simulink model "ImpedanceControl"  (R2017a)
(part 7 of 14)

(((real(dq6.*cos(q6).*(sin(q2-q3).*sin(q5).*8.191520442889917e-1-cos(q2-q3).*cos(q4).*cos(q5)+cos(q2-q3).*sin(q4).*sin(q5).*5.735764363510462e-1))+real(sin(q6).*(dq5.*sin(q2-q3).*cos(q5).*8.191520442889917e-1+cos(q2-q3).*sin(q5).*(dq2-dq3).*8.191520442889917e-1+dq4.*cos(q2-q3).*cos(q4).*sin(q5).*5.735764363510462e-1+dq4.*cos(q2-q3).*cos(q5).*sin(q4)+dq5.*cos(q2-q3).*cos(q4).*sin(q5)+dq5.*cos(q2-q3).*cos(q5).*sin(q4).*5.735764363510462e-1+sin(q2-q3).*cos(q4).*cos(q5).*(dq2-dq3)-sin(q2-q3).*sin(q4).*sin(q5).*(dq2-dq3).*5.735764363510462e-1))-imag(sin(q2-q3).*sin(q4).*(dq2-dq3)).*4.698463103929542e-1-imag(dq5.*sin(q5).*(sin(q2-q3).*8.191520442889917e-1+cos(q2-q3).*sin(q4).*5.735764363510462e-1)).*8.191520442889917e-1-imag(cos(q2-q3).*(dq2-dq3)).*3.289899283371657e-1-real(cos(q6).*(cos(q5).*(cos(q2-q3).*(dq2-dq3).*8.191520442889917e-1+dq4.*cos(q2-q3).*cos(q4).*5.735764363510462e-1-sin(q2-q3).*sin(q4).*(dq2-dq3).*5.735764363510462e-1).*5.735764363510462e-1+cos(q2-q3).*(dq2-dq3).*4.698463103929542e-1-dq4.*cos(q2-q3).*cos(q4).*6.710100716628342e-1+sin(q2-q3).*sin(q4).*(dq2-dq3).*6.710100716628342e-1-dq5.*sin(q5).*(sin(q2-q3).*8.191520442889917e-1+cos(q2-q3).*sin(q4).*5.735764363510462e-1).*5.735764363510462e-1+dq5.*cos(q2-q3).*cos(q4).*cos(q5).*5.735764363510462e-1-dq4.*cos(q2-q3).*sin(q4).*sin(q5).*5.735764363510462e-1-sin(q2-q3).*cos(q4).*sin(q5).*(dq2-dq3).*5.735764363510462e-1))+imag(cos(q5).*(cos(q2-q3).*(dq2-dq3).*8.191520442889917e-1+dq4.*cos(q2-q3).*cos(q4).*5.735764363510462e-1-sin(q2-q3).*sin(q4).*(dq2-dq3).*5.735764363510462e-1)).*8.191520442889917e-1+real(dq6.*sin(q6).*(sin(q2-q3).*4.698463103929542e-1-cos(q2-q3).*sin(q4).*6.710100716628342e-1+cos(q5).*(sin(q2-q3).*8.191520442889917e-1+cos(q2-q3).*sin(q4).*5.735764363510462e-1).*5.735764363510462e-1+cos(q2-q3).*cos(q4).*sin(q5).*5.735764363510462e-1))+imag(dq5.*cos(q2-q3).*cos(q4).*cos(q5)).*8.191520442889917e-1-imag(dq4.*cos(q2-q3).*sin(q4).*sin(q5)).*8.191520442889917e-1+imag(dq4.*cos(q2-q3).*cos(q4)).*4.698463103929542e-1-imag(sin(q2-q3).*cos(q4).*sin(q5).*(dq2-dq3)).*8.191520442889917e-1)./(real(cos(q2-q3)).*3.289899283371657e-1+real(sin(q2-q3).*cos(q4).*sin(q5)).*8.191520442889917e-1+real(sin(q2-q3).*sin(q4)).*4.698463103929542e-1+imag(sin(q6).*(cos(q2-q3).*sin(q5).*8.191520442889917e-1+sin(q2-q3).*cos(q4).*cos(q5)-sin(q2-q3).*sin(q4).*sin(q5).*5.735764363510462e-1))-real(cos(q5).*(cos(q2-q3).*8.191520442889917e-1-sin(q2-q3).*sin(q4).*5.735764363510462e-1)).*8.191520442889917e-1-imag(cos(q6).*(cos(q2-q3).*4.698463103929542e-1+sin(q2-q3).*sin(q4).*6.710100716628342e-1+cos(q5).*(cos(q2-q3).*8.191520442889917e-1-sin(q2-q3).*sin(q4).*5.735764363510462e-1).*5.735764363510462e-1-sin(q2-q3).*cos(q4).*sin(q5).*5.735764363510462e-1)))-(real(sin(q2-q3)).*(-3.289899283371657e-1)+real(cos(q2-q3).*cos(q4).*sin(q5)).*8.191520442889917e-1+real(cos(q2-q3).*sin(q4)).*4.698463103929542e-1-imag(sin(q6).*(sin(q2-q3).*sin(q5).*8.191520442889917e-1-cos(q2-q3).*cos(q4).*cos(q5)+cos(q2-q3).*sin(q4).*sin(q5).*5.735764363510462e-1))+real(cos(q5).*(sin(q2-q3).*8.191520442889917e-1+cos(q2-q3).*sin(q4).*5.735764363510462e-1)).*8.191520442889917e-1+imag(cos(q6).*(sin(q2-q3).*4.698463103929542e-1-cos(q2-q3).*sin(q4).*6.710100716628342e-1+cos(q5).*(sin(q2-q3).*8.191520442889917e-1+cos(q2-q3).*sin(q4).*5.735764363510462e-1).*5.735764363510462e-1+cos(q2-q3).*cos(q4).*sin(q5).*5.735764363510462e-1))).*1.0./(real(cos(q2-q3)).*3.289899283371657e-1+real(sin(q2-q3).*cos(q4).*sin(q5)).*8.191520442889917e-1+real(sin(q2-q3).*sin(q4)).*4.698463103929542e-1+imag(sin(q6).*(cos(q2-q3).*sin(q5).*8.191520442889917e-1+sin(q2-q3).*cos(q4).*cos(q5)-sin(q2-q3).*sin(q4).*sin(q5).*5.735764363510462e-1))-real(cos(q5).*(cos(q2-q3).*8.191520442889917e-1-sin(q2-q3).*sin(q4).*5.735764363510462e-1)).*8.191520442889917e-1-imag(cos(q6).*(cos(q2-q3).*4.698463103929542e-1+sin(q2-q3).*sin(q4).*6.710100716628342e-1+cos(q5).*(cos(q2-q3).*8.191520442889917e-1-sin(q2-q3).*sin(q4).*5.735764363510462e-1).*5.735764363510462e-1-sin(q2-q3).*cos(q4).*sin(q5).*5.735764363510462e-1))).^2.*(-real(dq6.*cos(q6).*(cos(q2-q3).*sin(q5).*8.191520442889917e-1+sin(q2-q3).*cos(q4).*cos(q5)-sin(q2-q3).*sin(q4).*sin(q5).*5.735764363510462e-1))+imag(cos(q2-q3).*sin(q4).*(dq2-dq3)).*4.698463103929542e-1+imag(dq5.*sin(q5).*(cos(q2-q3).*8.191520442889917e-1-sin(q2-q3).*sin(q4).*5.735764363510462e-1)).*8.191520442889917e-1+real(sin(q6).*(dq5.*cos(q2-q3).*cos(q5).*(-8.191520442889917e-1)+sin(q2-q3).*sin(q5).*(dq2-dq3).*8.191520442889917e-1+dq4.*sin(q2-q3).*cos(q4).*sin(q5).*5.735764363510462e-1+dq4.*sin(q2-q3).*cos(q5).*sin(q4)+dq5.*sin(q2-q3).*cos(q4).*sin(q5)+dq5.*sin(q2-q3).*cos(q5).*sin(q4).*5.735764363510462e-1-cos(q2-q3).*cos(q4).*cos(q5).*(dq2-dq3)+cos(q2-q3).*sin(q4).*sin(q5).*(dq2-dq3).*5.735764363510462e-1))-imag(sin(q2-q3).*(dq2-dq3)).*3.289899283371657e-1-real(cos(q6).*(cos(q5).*(sin(q2-q3).*(dq2-dq3).*8.191520442889917e-1+dq4.*sin(q2-q3).*cos(q4).*5.735764363510462e-1+cos(q2-q3).*sin(q4).*(dq2-dq3).*5.735764363510462e-1).*5.735764363510462e-1+sin(q2-q3).*(dq2-dq3).*4.698463103929542e-1-dq4.*sin(q2-q3).*cos(q4).*6.710100716628342e-1-cos(q2-q3).*sin(q4).*(dq2-dq3).*6.710100716628342e-1+dq5.*sin(q5).*(cos(q2-q3).*8.191520442889917e-1-sin(q2-q3).*sin(q4).*5.735764363510462e-1).*5.735764363510462e-1+dq5.*sin(q2-q3).*cos(q4).*cos(q5).*5.735764363510462e-1-dq4.*sin(q2-q3).*sin(q4).*sin(q5).*5.735764363510462e-1+cos(q2-q3).*cos(q4).*sin(q5).*(dq2-dq3).*5.735764363510462e-1))+imag(cos(q5).*(sin(q2-q3).*(dq2-dq3).*8.191520442889917e-1+dq4.*sin(q2-q3).*cos(q4).*5.735764363510462e-1+cos(q2-q3).*sin(q4).*(dq2-dq3).*5.735764363510462e-1)).*8.191520442889917e-1-real(dq6.*sin(q6).*(cos(q2-q3).*4.698463103929542e-1+sin(q2-q3).*sin(q4).*6.710100716628342e-1+cos(q5).*(cos(q2-q3).*8.191520442889917e-1-sin(q2-q3).*sin(q4).*5.735764363510462e-1).*5.735764363510462e-1-sin(q2-q3).*cos(q4).*sin(q5).*5.735764363510462e-1))+imag(dq5.*sin(q2-q3).*cos(q4).*cos(q5)).*8.191520442889917e-1-imag(dq4.*sin(q2-q3).*sin(q4).*sin(q5)).*8.191520442889917e-1+imag(cos(q2-q3).*cos(q4).*sin(q5).*(dq2-dq3)).*8.191520442889917e-1+imag(dq4.*sin(q2-q3).*cos(q4)).*4.698463103929542e-1)-(imag(sin(q2-q3)).*(-3.289899283371657e-1)+imag(cos(q2-q3).*cos(q4).*sin(q5)).*8.191520442889917e-1+imag(cos(q2-q3).*sin(q4)).*4.698463103929542e-1+real(sin(q6).*(sin(q2-q3).*sin(q5).*8.191520442889917e-1-cos(q2-q3).*cos(q4).*cos(q5)+cos(q2-q3).*sin(q4).*sin(q5).*5.735764363510462e-1))+imag(cos(q5).*(sin(q2-q3).*8.191520442889917e-1+cos(q2-q3).*sin(q4).*5.735764363510462e-1)).*8.191520442889917e-1-real(cos(q6).*(sin(q2-q3).*4.698463103929542e-1-cos(q2-q3).*sin(q4).*6.710100716628342e-1+cos(q5).*(sin(q2-q3).*8.191520442889917e-1+cos(q2-q3).*sin(q4).*5.735764363510462e-1).*5.735764363510462e-1+cos(q2-q3).*cos(q4).*sin(q5).*5.735764363510462e-1))).*1.0./(real(cos(q2-q3)).*3.289899283371657e-1+real(sin(q2-q3).*cos(q4).*sin(q5)).*8.191520442889917e-1+real(sin(q2-q3).*sin(q4)).*4.698463103929542e-1+imag(sin(q6).*(cos(q2-q3).*sin(q5).*8.191520442889917e-1+sin(q2-q3).*cos(q4).*cos(q5)-sin(q2-q3).*sin(q4).*sin(q5).*5.735764363510462e-1))-real(cos(q5).*(cos(q2-q3).*8.191520442889917e-1-sin(q2-q3).*sin(q4).*5.735764363510462e-1)).*8.191520442889917e-1-imag(cos(q6).*(cos(q2-q3).*4.698463103929542e-1+sin(q2-q3).*sin(q4).*6.710100716628342e-1+cos(q5).*(cos(q2-q3).*8.191520442889917e-1-sin(q2-q3).*sin(q4).*5.735764363510462e-1).*5.735764363510462e-1-sin(q2-q3).*cos(q4).*sin(q5).*5.735764363510462e-1))).^2.*(imag(dq6.*cos(q6).*(cos(q2-q3).*sin(q5).*8.191520442889917e-1+sin(q2-q3).*cos(q4).*cos(q5)-sin(q2-q3).*sin(q4).*sin(q5).*5.735764363510462e-1))+real(cos(q2-q3).*sin(q4).*(dq2-dq3)).*4.698463103929542e-1-imag(sin(q6).*(dq5.*cos(q2-q3).*cos(q5).*(-8.191520442889917e-1)+sin(q2-q3).*sin(q5).*(dq2-dq3).*8.191520442889917e-1+dq4.*sin(q2-q3).*cos(q4).*sin(q5).*5.735764363510462e-1+dq4.*sin(q2-q3).*cos(q5).*sin(q4)+dq5.*sin(q2-q3).*cos(q4).*sin(q5)+dq5.*sin(q2-q3).*cos(q5).*sin(q4).*5.735764363510462e-1-cos(q2-q3).*cos(q4).*cos(q5).*(dq2-dq3)+cos(q2-q3).*sin(q4).*sin(q5).*(dq2-dq3).*5.735764363510462e-1))+real(dq5.*sin(q5).*(cos(q2-q3).*8.191520442889917e-1-sin(q2-q3).*sin(q4).*5.735764363510462e-1)).*8.191520442889917e-1-real(sin(q2-q3).*(dq2-dq3)).*3.289899283371657e-1+imag(cos(q6).*(cos(q5).*(sin(q2-q3).*(dq2-dq3).*8.191520442889917e-1+dq4.*sin(q2-q3).*cos(q4).*5.735764363510462e-1+cos(q2-q3).*sin(q4).*(dq2-dq3).*5.735764363510462e-1).*5.735764363510462e-1+sin(q2-q3).*(dq2-dq3).*4.698463103929542e-1-dq4.*sin(q2-q3).*cos(q4).*6.710100716628342e-1-cos(q2-q3).*sin(q4).*(dq2-dq3).*6.710100716628342e-1+dq5.*sin(q5).*(cos(q2-q3).*8.191520442889917e-1-sin(q2-q3).*sin(q4).*5.735764363510462e-1).*5.735764363510462e-1+dq5.*sin(q2-q3).*cos(q4).*cos(q5).*5.735764363510462e-1-dq4.*sin(q2-q3).*sin(q4).*sin(q5).*5.735764363510462e-1+cos(q2-q3).*cos(q4).*sin(q5).*(dq2-dq3).*5.735764363510462e-1))+imag(dq6.*sin(q6).*(cos(q2-q3).*4.698463103929542e-1+sin(q2-q3).*sin(q4).*6.710100716628342e-1+cos(q5).*(cos(q2-q3).*8.191520442889917e-1-sin(q2-q3).*sin(q4).*5.735764363510462e-1).*5.735764363510462e-1-sin(q2-q3).*cos(q4).*sin(q5).*5.735764363510462e-1))+real(cos(q5).*(sin(q2-q3).*(dq2-dq3).*8.191520442889917e-1+dq4.*sin(q2-q3).*cos(q4).*5.735764363510462e-1+cos(q2-q3).*sin(q4).*(dq2-dq3).*5.735764363510462e-1)).*8.191520442889917e-1+real(dq5.*sin(q2-q3).*cos(q4).*cos(q5)).*8.191520442889917e-1-real(dq4.*sin(q2-q3).*sin(q4).*sin(q5)).*8.191520442889917e-1+real(cos(q2-q3).*cos(q4).*sin(q5).*(dq2-dq3)).*8.191520442889917e-1+real(dq4.*sin(q2-q3).*cos(q4)).*4.698463103929542e-1)+(real(cos(q6).*(cos(q2-q3).*4.698463103929542e-1+sin(q2-q3).*sin(q4).*6.710100716628342e-1+cos(q5).*(cos(q2-q3).*8.191520442889917e-1-sin(q2-q3).*sin(q4).*5.735764363510462e-1).*5.735764363510462e-1-sin(q2-q3).*cos(q4).*sin(q5).*5.735764363510462e-1))+imag(cos(q2-q3)).*3.289899283371657e-1+imag(sin(q2-q3).*cos(q4).*sin(q5)).*8.191520442889917e-1+imag(sin(q2-q3).*sin(q4)).*4.698463103929542e-1-real(sin(q6).*(cos(q2-q3).*sin(q5).*8.191520442889917e-1+sin(q2-q3).*cos(q4).*cos(q5)-sin(q2-q3).*sin(q4).*sin(q5).*5.735764363510462e-1))-imag(cos(q5).*(cos(q2-q3).*8.191520442889917e-1-sin(q2-q3).*sin(q4).*5.735764363510462e-1)).*8.191520442889917e-1).*1.0./(real(cos(q2-q3)).*3.289899283371657e-1+real(sin(q2-q3).*cos(q4).*sin(q5)).*8.191520442889917e-1+real(sin(q2-q3).*sin(q4)).*4.698463103929542e-1+imag(sin(q6).*(cos(q2-q3).*sin(q5).*8.191520442889917e-1+sin(q2-q3).*cos(q4).*cos(q5)-sin(q2-q3).*sin(q4).*sin(q5).*5.735764363510462e-1))-real(cos(q5).*(cos(q2-q3).*8.191520442889917e-1-sin(q2-q3).*sin(q4).*5.735764363510462e-1)).*8.191520442889917e-1-imag(cos(q6).*(cos(q2-q3).*4.698463103929542e-1+sin(q2-q3).*sin(q4).*6.710100716628342e-1+cos(q5).*(cos(q2-q3).*8.191520442889917e-1-sin(q2-q3).*sin(q4).*5.735764363510462e-1).*5.735764363510462e-1-sin(q2-q3).*cos(q4).*sin(q5).*5.735764363510462e-1))).^2.*(real(sin(q2-q3).*cos(q4).*sin(q5).*(dq2-dq3)).*8.191520442889917e-1+imag(sin(q6).*(dq5.*sin(q2-q3).*cos(q5).*8.191520442889917e-1+cos(q2-q3).*sin(q5).*(dq2-dq3).*8.191520442889917e-1+dq4.*cos(q2-q3).*cos(q4).*sin(q5).*5.735764363510462e-1+dq4.*cos(q2-q3).*cos(q5).*sin(q4)+dq5.*cos(q2-q3).*cos(q4).*sin(q5)+dq5.*cos(q2-q3).*cos(q5).*sin(q4).*5.735764363510462e-1+sin(q2-q3).*cos(q4).*cos(q5).*(dq2-dq3)-sin(q2-q3).*sin(q4).*sin(q5).*(dq2-dq3).*5.735764363510462e-1))+real(sin(q2-q3).*sin(q4).*(dq2-dq3)).*4.698463103929542e-1-imag(cos(q6).*(cos(q5).*(cos(q2-q3).*(dq2-dq3).*8.191520442889917e-1+dq4.*cos(q2-q3).*cos(q4).*5.735764363510462e-1-sin(q2-q3).*sin(q4).*(dq2-dq3).*5.735764363510462e-1).*5.735764363510462e-1+cos(q2-q3).*(dq2-dq3).*4.698463103929542e-1-dq4.*cos(q2-q3).*cos(q4).*6.710100716628342e-1+sin(q2-q3).*sin(q4).*(dq2-dq3).*6.710100716628342e-1-dq5.*sin(q5).*(sin(q2-q3).*8.191520442889917e-1+cos(q2-q3).*sin(q4).*5.735764363510462e-1).*5.735764363510462e-1+dq5.*cos(q2-q3).*cos(q4).*cos(q5).*5.735764363510462e-1-dq4.*cos(q2-q3).*sin(q4).*sin(q5).*5.735764363510462e-1-sin(q2-q3).*cos(q4).*sin(q5).*(dq2-dq3).*5.735764363510462e-1))+real(dq5.*sin(q5).*(sin(q2-q3).*8.191520442889917e-1+cos(q2-q3).*sin(q4).*5.735764363510462e-1)).*8.191520442889917e-1+real(cos(q2-q3).*(dq2-dq3)).*3.289899283371657e-1+imag(dq6.*sin(q6).*(sin(q2-q3).*4.698463103929542e-1-cos(q2-q3).*sin(q4).*6.710100716628342e-1+cos(q5).*(sin(q2-q3).*8.191520442889917e-1+cos(q2-q3).*sin(q4).*5.735764363510462e-1).*5.735764363510462e-1+cos(q2-q3).*cos(q4).*sin(q5).*5.735764363510462e-1))-real(cos(q5).*(cos(q2-q3).*(dq2-dq3).*8.191520442889917e-1+dq4.*cos(q2-q3).*cos(q4).*5.735764363510462e-1-sin(q2-q3).*sin(q4).*(dq2-dq3).*5.735764363510462e-1)).*8.191520442889917e-1-real(dq5.*cos(q2-q3).*cos(q4).*cos(q5)).*8.191520442889917e-1+real(dq4.*cos(q2-q3).*sin(q4).*sin(q5)).*8.191520442889917e-1-real(dq4.*cos(q2-q3).*cos(q4)).*4.698463103929542e-1+imag(dq6.*cos(q6).*(sin(q2-q3).*sin(q5).*8.191520442889917e-1-cos(q2-q3).*cos(q4).*cos(q5)+cos(q2-q3).*sin(q4).*sin(q5).*5.735764363510462e-1)))+(real(sin(q2-q3)).*(-3.289899283371657e-1)+real(cos(q2-q3).*cos(q4).*sin(q5)).*8.191520442889917e-1+real(cos(q2-q3).*sin(q4)).*4.698463103929542e-1-imag(sin(q6).*(sin(q2-q3).*sin(q5).*8.191520442889917e-1-cos(q2-q3).*cos(q4).*cos(q5)+cos(q2-q3).*sin(q4).*sin(q5).*5.735764363510462e-1))+real(cos(q5).*(sin(q2-q3).*8.191520442889917e-1+cos(q2-q3).*sin(q4).*5.735764363510462e-1)).*8.191520442889917e-1+imag(cos(q6).*(sin(q2-q3).*4.698463103929542e-1-cos(q2-q3).*sin(q4).*6.710100716628342e-1+cos(q5).*(sin(q2-q3).*8.191520442889917e-1+cos(q2-q3).*sin(q4).*5.735764363510462e-1).*5.735764363510462e-1+cos(q2-q3).*cos(q4).*sin(q5).*5.735764363510462e-1))).*(real(cos(q6).*(cos(q2-q3).*4.698463103929542e-1+sin(q2-q3).*sin(q4).*6.710100716628342e-1+cos(q5).*(cos(q2-q3).*8.191520442889917e-1-sin(q2-q3).*sin(q4).*5.735764363510462e-1).*5.735764363510462e-1-sin(q2-q3).*cos(q4).*sin(q5).*5.735764363510462e-1))+imag(cos(q2-q3)).*3.289899283371657e-1+imag(sin(q2-q3).*cos(q4).*sin(q5)).*8.191520442889917e-1+imag(sin(q2-q3).*sin(q4)).*4.698463103929542e-1-real(sin(q6).*(cos(q2-q3).*sin(q5).*8.191520442889917e-1+sin(q2-q3).*cos(q4).*cos(q5)-sin(q2-q3).*sin(q4).*sin(q5).*5.735764363510462e-1))-imag(cos(q5).*(cos(q2-q3).*8.191520442889917e-1-sin(q2-q3).*sin(q4).*5.735764363510462e-1)).*8.191520442889917e-1).*1.0./(real(cos(q2-q3)).*3.289899283371657e-1+real(sin(q2-q3).*cos(q4).*sin(q5)).*8.191520442889917e-1+real(sin(q2-q3).*sin(q4)).*4.698463103929542e-1+imag(sin(q6).*(cos(q2-q3).*sin(q5).*8.191520442889917e-1+sin(q2-q3).*cos(q4).*cos(q5)-sin(q2-q3).*sin(q4).*sin(q5).*5.735764363510462e-1))-real(cos(q5).*(cos(q2-q3).*8.191520442889917e-1-sin(q2-q3).*sin(q4).*5.735764363510462e-1)).*8.191520442889917e-1-imag(cos(q6).*(cos(q2-q3).*4.698463103929542e-1+sin(q2-q3).*sin(q4).*6.710100716628342e-1+cos(q5).*(cos(q2-q3).*8.191520442889917e-1-sin(q2-q3).*sin(q4).*5.735764363510462e-1).*5.735764363510462e-1-sin(q2-q3).*cos(q4).*sin(q5).*5.735764363510462e-1))).^3.*(imag(dq6.*cos(q6).*(cos(q2-q3).*sin(q5).*8.191520442889917e-1+sin(q2-q3).*cos(q4).*cos(q5)-sin(q2-q3).*sin(q4).*sin(q5).*5.735764363510462e-1))+real(cos(q2-q3).*sin(q4).*(dq2-dq3)).*4.698463103929542e-1-imag(sin(q6).*(dq5.*cos(q2-q3).*cos(q5).*(-8.191520442889917e-1)+sin(q2-q3).*sin(q5).*(dq2-dq3).*8.191520442889917e-1+dq4.*sin(q2-q3).*cos(q4).*sin(q5).*5.735764363510462e-1+dq4.*sin(q2-q3).*cos(q5).*sin(q4)+dq5.*sin(q2-q3).*cos(q4).*sin(q5)+dq5.*sin(q2-q3).*cos(q5).*sin(q4).*5.735764363510462e-1-cos(q2-q3).*cos(q4).*cos(q5).*(dq2-dq3)+cos(q2-q3).*sin(q4).*sin(q5).*(dq2-dq3).*5.735764363510462e-1))+real(dq5.*sin(q5).*(cos(q2-q3).*8.191520442889917e-1-sin(q2-q3).*sin(q4).*5.735764363510462e-1)).*8.191520442889917e-1-real(sin(q2-q3).*(dq2-dq3)).*3.289899283371657e-1+imag(cos(q6).*(cos(q5).*(sin(q2-q3).*(dq2-dq3).*8.191520442889917e-1+dq4.*sin(q2-q3).*cos(q4).*5.735764363510462e-1+cos(q2-q3).*sin(q4).*(dq2-dq3).*5.735764363510462e-1).*5.735764363510462e-1+sin(q2-q3).*(dq2-dq3).*4.698463103929542e-1-dq4.*sin(q2-q3).*cos(q4).*6.710100716628342e-1-cos(q2-q3).*sin(q4).*(dq2-dq3).*6.710100716628342e-1+dq5.*sin(q5).*(cos(q2-q3).*8.191520442889917e-1-sin(q2-q3).*sin(q4).*5.735764363510462e-1).*5.735764363510462e-1+dq5.*sin(q2-q3).*cos(q4).*cos(q5).*5.735764363510462e-1-dq4.*sin(q2-q3).*sin(q4).*sin(q5).*5.735764363510462e-1+cos(q2-q3).*cos(q4).*sin(q5).*(dq2-dq3).*5.735764363510462e-1))+imag(dq6.*sin(q6).*(cos(q2-q3).*4.698463103929542e-1+sin(q2-q3).*sin(q4).*6.710100716628342e-1+cos(q5).*(cos(q2-q3).*8.191520442889917e-1-sin(q2-q3).*sin(q4).*5.735764363510462e-1).*5.735764363510462e-1-sin(q2-q3).*cos(q4).*sin(q5).*5.735764363510462e-1))+real(cos(q5).*(sin(q2-q3).*(dq2-dq3).*8.191520442889917e-1+dq4.*sin(q2-q3).*cos(q4).*5.735764363510462e-1+cos(q2-q3).*sin(q4).*(dq2-dq3).*5.735764363510462e-1)).*8.191520442889917e-1+real(dq5.*sin(q2-q3).*cos(q4).*cos(q5)).*8.191520442889917e-1-real(dq4.*sin(q2-q3).*sin(q4).*sin(q5)).*8.191520442889917e-1+real(cos(q2-q3).*cos(q4).*sin(q5).*(dq2-dq3)).*8.191520442889917e-1+real(dq4.*sin(q2-q3).*cos(q4)).*4.698463103929542e-1).*2.0).*(real(cos(q2-q3)).*3.289899283371657e-1+real(sin(q2-q3).*cos(q4).*sin(q5)).*8.191520442889917e-1+real(sin(q2-q3).*sin(q4)).*4.698463103929542e-1+imag(sin(q6).*(cos(q2-q3).*sin(q5).*8.191520442889917e-1+sin(q2-q3).*cos(q4).*cos(q5)-sin(q2-q3).*sin(q4).*sin(q5).*5.735764363510462e-1))-real(cos(q5).*(cos(q2-q3).*8.191520442889917e-1-sin(q2-q3).*sin(q4).*5.735764363510462e-1)).*8.191520442889917e-1-imag(cos(q6).*(cos(q2-q3).*4.698463103929542e-1+sin(q2-q3).*sin(q4).*6.710100716628342e-1+cos(q5).*(cos(q2-q3).*8.191520442889917e-1-sin(q2-q3).*sin(q4).*5.735764363510462e-1).*5.735764363510462e-1-sin(q2-q3).*cos(q4).*sin(q5).*5.735764363510462e-1))).^2)./((real(cos(q6).*(cos(q2-q3).*4.698463103929542e-1+sin(q2-q3).*sin(q4).*6.710100716628342e-1+cos(q5).*(cos(q2-q3).*8.191520442889917e-1-sin(q2-q3).*sin(q4).*5.735764363510462e-1).*5.735764363510462e-1-sin(q2-q3).*cos(q4).*sin(q5).*5.735764363510462e-1))+imag(cos(q2-q3)).*3.289899283371657e-1+imag(sin(q2-q3).*cos(q4).*sin(q5)).*8.191520442889917e-1+imag(sin(q2-q3).*sin(q4)).*4.698463103929542e-1-real(sin(q6).*(cos(q2-q3).*sin(q5).*8.191520442889917e-1+sin(q2-q3).*cos(q4).*cos(q5)-sin(q2-q3).*sin(q4).*sin(q5).*5.735764363510462e-1))-imag(cos(q5).*(cos(q2-q3).*8.191520442889917e-1-sin(q2-q3).*sin(q4).*5.735764363510462e-1)).*8.191520442889917e-1).^2+(real(cos(q2-q3)).*3.289899283371657e-1+real(sin(q2-q3).*cos(q4).*sin(q5)).*8.191520442889917e-1+real(sin(q2-q3).*sin(q4)).*4.698463103929542e-1+imag(sin(q6).*(cos(q2-q3).*sin(q5).*8.191520442889917e-1+sin(q2-q3).*cos(q4).*cos(q5)-sin(q2-q3).*sin(q4).*sin(q5).*5.735764363510462e-1))-real(cos(q5).*(cos(q2-q3).*8.191520442889917e-1-sin(q2-q3).*sin(q4).*5.735764363510462e-1)).*8.191520442889917e-1-imag(cos(q6).*(cos(q2-q3).*4.698463103929542e-1+sin(q2-q3).*sin(q4).*6.710100716628342e-1+cos(q5).*(cos(q2-q3).*8.191520442889917e-1-sin(q2-q3).*sin(q4).*5.735764363510462e-1).*5.735764363510462e-1-sin(q2-q3).*cos(q4).*sin(q5).*5.735764363510462e-1))).^2)-((imag(sin(q2-q3)).*(-3.289899283371657e-1)+imag(cos(q2-q3).*cos(q4).*sin(q5)).*8.191520442889917e-1+imag(cos(q2-q3).*sin(q4)).*4.698463103929542e-1+real(sin(q6).*(sin(q2-q3).*sin(q5).*8.191520442889917e-1-cos(q2-q3).*cos(q4).*cos(q5)+cos(q2-q3).*sin(q4).*sin(q5).*5.735764363510462e-1))+imag(cos(q5).*(sin(q2-q3).*8.191520442889917e-1+cos(q2-q3).*sin(q4).*5.735764363510462e-1)).*8.191520442889917e-1-real(cos(q6).*(sin(q2-q3).*4.698463103929542e-1-cos(q2-q3).*sin(q4).*6.710100716628342e-1+cos(q5).*(sin(q2-q3).*8.191520442889917e-1+cos(q2-q3).*sin(q4).*5.735764363510462e-1).*5.735764363510462e-1+cos(q2-q3).*cos(q4).*sin(q5).*5.735764363510462e-1)))./(real(cos(q2-q3)).*3.289899283371657e-1+real(sin(q2-q3).*cos(q4).*sin(q5)).*8.191520442889917e-1+real(sin(q2-q3).*sin(q4)).*4.698463103929542e-1+imag(sin(q6).*(cos(q2-q3).*sin(q5).*8.191520442889917e-1+sin(q2-q3).*cos(q4).*cos(q5)-sin(q2-q3).*sin(q4).*sin(q5).*5.735764363510462e-1))-real(cos(q5).*(cos(q2-q3).*8.191520442889917e-1-sin(q2-q3).*sin(q4).*5.735764363510462e-1)).*8.191520442889917e-1-imag(cos(q6).*(cos(q2-q3).*4.698463103929542e-1+sin(q2-q3).*sin(q4).*6.710100716628342e-1+cos(q5).*(cos(q2-q3).*8.191520442889917e-1-sin(q2-q3).*sin(q4).*5.735764363510462e-1).*5.735764363510462e-1-sin(q2-q3).*cos(q4).*sin(q5).*5.735764363510462e-1)))-(real(sin(q2-q3)).*(-3.289899283371657e-1)+real(cos(q2-q3).*cos(q4).*sin(q5)).*8.191520442889917e-1+real(cos(q2-q3).*sin(q4)).*4.698463103929542e-1-imag(sin(q6).*(sin(q2-q3).*sin(q5).*8.191520442889917e-1-cos(q2-q3).*cos(q4).*cos(q5)+cos(q2-q3).*sin(q4).*sin(q5).*5.735764363510462e-1))+real(cos(q5).*(sin(q2-q3).*8.191520442889917e-1+cos(q2-q3).*sin(q4).*5.735764363510462e-1)).*8.191520442889917e-1+imag(cos(q6).*(sin(q2-q3).*4.698463103929542e-1-cos(q2-q3).*sin(q4).*6.710100716628342e-1+cos(q5).*(sin(q2-q3).*8.191520442889917e-1+cos(q2-q3).*sin(q4).*5.735764363510462e-1).*5.735764363510462e-1+cos(q2-q3).*cos(q4).*sin(q5).*5.735764363510462e-1))).*(real(cos(q6).*(cos(q2-q3).*4.698463103929542e-1+sin(q2-q3).*sin(q4).*6.710100716628342e-1+cos(q5).*(cos(q2-q3).*8.191520442889917e-1-sin(q2-q3).*sin(q4).*5.735764363510462e-1).*5.735764363510462e-1-sin(q2-q3).*cos(q4).*sin(q5).*5.735764363510462e-1))+imag(cos(q2-q3)).*3.289899283371657e-1+imag(sin(q2-q3).*cos(q4).*sin(q5)).*8.191520442889917e-1+imag(sin(q2-q3).*sin(q4)).*4.698463103929542e-1-real(sin(q6).*(cos(q2-q3).*sin(q5).*8.191520442889917e-1+sin(q2-q3).*cos(q4).*cos(q5)-sin(q2-q3).*sin(q4).*sin(q5).*5.735764363510462e-1))-imag(cos(q5).*(cos(q2-q3).*8.191520442889917e-1-sin(q2-q3).*sin(q4).*5.735764363510462e-1)).*8.191520442889917e-1).*1.0./(real(cos(q2-q3)).*3.289899283371657e-1+real(sin(q2-q3).*cos(q4).*sin(q5)).*8.191520442889917e-1+real(sin(q2-q3).*sin(q4)).*4.698463103929542e-1+imag(sin(q6).*(cos(q2-q3).*sin(q5).*8.191520442889917e-1+sin(q2-q3).*cos(q4).*cos(q5)-sin(q2-q3).*sin(q4).*sin(q5).*5.735764363510462e-1))-real(cos(q5).*(cos(q2-q3).*8.191520442889917e-1-sin(q2-q3).*sin(q4).*5.735764363510462e-1)).*8.191520442889917e-1-imag(cos(q6).*(cos(q2-q3).*4.698463103929542e-1+sin(q2-q3).*sin(q4).*6.710100716628342e-1+cos(q5).*(cos(q2-q3).*8.191520442889917e-1-sin(q2-q3).*sin(q4).*5.735764363510462e-1).*5.735764363510462e-1-sin(q2-q3).*cos(q4).*sin(q5).*5.735764363510462e-1))).^2).*1.0./((real(cos(q6).*(cos(q2-q3).*4.698463103929542e-1+sin(q2-q3).*sin(q4).*6.710100716628342e-1+cos(q5).*(cos(q2-q3).*8.191520442889917e-1-sin(q2-q3).*sin(q4).*5.735764363510462e-1).*5.735764363510462e-1-sin(q2-q3).*cos(q4).*sin(q5).*5.735764363510462e-1))+imag(cos(q2-q3)).*3.289899283371657e-1+imag(sin(q2-q3).*cos(q4).*sin(q5)).*8.191520442889917e-1+imag(sin(q2-q3).*sin(q4)).*4.698463103929542e-1-real(sin(q6).*(cos(q2-q3).*sin(q5).*8.191520442889917e-1+sin(q2-q3).*cos(q4).*cos(q5)-sin(q2-q3).*sin(q4).*sin(q5).*5.735764363510462e-1))-imag(cos(q5).*(cos(q2-q3).*8.191520442889917e-1-sin(q2-q3).*sin(q4).*5.735764363510462e-1)).*8.191520442889917e-1).^2+(real(cos(q2-q3)).*3.289899283371657e-1+real(sin(q2-q3).*cos(q4).*sin(q5)).*8.191520442889917e-1+real(sin(q2-q3).*sin(q4)).*4.698463103929542e-1+imag(sin(q6).*(cos(q2-q3).*sin(q5).*8.191520442889917e-1+sin(q2-q3).*cos(q4).*cos(q5)-sin(q2-q3).*sin(q4).*sin(q5).*5.735764363510462e-1))-real(cos(q5).*(cos(q2-q3).*8.191520442889917e-1-sin(q2-q3).*sin(q4).*5.735764363510462e-1)).*8.191520442889917e-1-imag(cos(q6).*(cos(q2-q3).*4.698463103929542e-1+sin(q2-q3).*sin(q4).*6.710100716628342e-1+cos(q5).*(cos(q2-q3).*8.191520442889917e-1-sin(q2-q3).*sin(q4).*5.735764363510462e-1).*5.735764363510462e-1-sin(q2-q3).*cos(q4).*sin(q5).*5.735764363510462e-1))).^2).^2.*((real(cos(q6).*(cos(q2-q3).*4.698463103929542e-1+sin(q2-q3).*sin(q4).*6.710100716628342e-1+cos(q5).*(cos(q2-q3).*8.191520442889917e-1-sin(q2-q3).*sin(q4).*5.735764363510462e-1).*5.735764363510462e-1-sin(q2-q3).*cos(q4).*sin(q5).*5.735764363510462e-1))+imag(cos(q2-q3)).*3.289899283371657e-1+imag(sin(q2-q3).*cos(q4).*sin(q5)).*8.191520442889917e-1+imag(sin(q2-q3).*sin(q4)).*4.698463103929542e-1-real(sin(q6).*(cos(q2-q3).*sin(q5).*8.191520442889917e-1+sin(q2-q3).*cos(q4).*cos(q5)-sin(q2-q3).*sin(q4).*sin(q5).*5.735764363510462e-1))-imag(cos(q5).*(cos(q2-q3).*8.191520442889917e-1-sin(q2-q3).*sin(q4).*5.735764363510462e-1)).*8.191520442889917e-1).*(-real(dq6.*cos(q6).*(cos(q2-q3).*sin(q5).*8.191520442889917e-1+sin(q2-q3).*cos(q4).*cos(q5)-sin(q2-q3).*sin(q4).*sin(q5).*5.735764363510462e-1))+imag(cos(q2-q3).*sin(q4).*(dq2-dq3)).*4.698463103929542e-1+imag(dq5.*sin(q5).*(cos(q2-q3).*8.191520442889917e-1-sin(q2-q3).*sin(q4).*5.735764363510462e-1)).*8.191520442889917e-1+real(sin(q6).*(dq5.*cos(q2-q3).*cos(q5).*(-8.191520442889917e-1)+sin(q2-q3).*sin(q5).*(dq2-dq3).*8.191520442889917e-1+dq4.*sin(q2-q3).*cos(q4).*sin(q5).*5.735764363510462e-1+dq4.*sin(q2-q3).*cos(q5).*sin(q4)+dq5.*sin(q2-q3).*cos(q4).*sin(q5)+dq5.*sin(q2-q3).*cos(q5).*sin(q4).*5.735764363510462e-1-cos(q2-q3).*cos(q4).*cos(q5).*(dq2-dq3)+cos(q2-q3).*sin(q4).*sin(q5).*(dq2-dq3).*5.735764363510462e-1))-imag(sin(q2-q3).*(dq2-dq3)).*3.289899283371657e-1-real(cos(q6).*(cos(q5).*(sin(q2-q3).*(dq2-dq3).*8.191520442889917e-1+dq4.*sin(q2-q3).*cos(q4).*5.735764363510462e-1+cos(q2-q3).*sin(q4).*(dq2-dq3).*5.735764363510462e-1).*5.735764363510462e-1+sin(q2-q3).*(dq2-dq3).*4.698463103929542e-1-dq4.*sin(q2-q3).*cos(q4).*6.710100716628342e-1-cos(q2-q3).*sin(q4).*(dq2-dq3).*6.710100716628342e-1+dq5.*sin(q5).*(cos(q2-q3).*8.191520442889917e-1-sin(q2-q3).*sin(q4).*5.735764363510462e-1).*5.735764363510462e-1+dq5.*sin(q2-q3).*cos(q4).*cos(q5).*5.735764363510462e-1-dq4.*sin(q2-q3).*sin(q4).*sin(q5).*5.735764363510462e-1+cos(q2-q3).*cos(q4).*sin(q5).*(dq2-dq3).*5.735764363510462e-1))+imag(cos(q5).*(sin(q2-q3).*(dq2-dq3).*8.191520442889917e-1+dq4.*sin(q2-q3).*cos(q4).*5.735764363510462e-1+cos(q2-q3).*sin(q4).*(dq2-dq3).*5.735764363510462e-1)).*8.191520442889917e-1-real(dq6.*sin(q6).*(cos(q2-q3).*4.698463103929542e-1+sin(q2-q3).*sin(q4).*6.710100716628342e-1+cos(q5).*(cos(q2-q3).*8.191520442889917e-1-sin(q2-q3).*sin(q4).*5.735764363510462e-1).*5.735764363510462e-1-sin(q2-q3).*cos(q4).*sin(q5).*5.735764363510462e-1))+imag(dq5.*sin(q2-q3).*cos(q4).*cos(q5)).*8.191520442889917e-1-imag(dq4.*sin(q2-q3).*sin(q4).*sin(q5)).*8.191520442889917e-1+imag(cos(q2-q3).*cos(q4).*sin(q5).*(dq2-dq3)).*8.191520442889917e-1+imag(dq4.*sin(q2-q3).*cos(q4)).*4.698463103929542e-1).*2.0+(real(cos(q2-q3)).*3.289899283371657e-1+real(sin(q2-q3).*cos(q4).*sin(q5)).*8.191520442889917e-1+real(sin(q2-q3).*sin(q4)).*4.698463103929542e-1+imag(sin(q6).*(cos(q2-q3).*sin(q5).*8.191520442889917e-1+sin(q2-q3).*cos(q4).*cos(q5)-sin(q2-q3).*sin(q4).*sin(q5).*5.735764363510462e-1))-real(cos(q5).*(cos(q2-q3).*8.191520442889917e-1-sin(q2-q3).*sin(q4).*5.735764363510462e-1)).*8.191520442889917e-1-imag(cos(q6).*(cos(q2-q3).*4.698463103929542e-1+sin(q2-q3).*sin(q4).*6.710100716628342e-1+cos(q5).*(cos(q2-q3).*8.191520442889917e-1-sin(q2-q3).*sin(q4).*5.735764363510462e-1).*5.735764363510462e-1-sin(q2-q3).*cos(q4).*sin(q5).*5.735764363510462e-1))).*(imag(dq6.*cos(q6).*(cos(q2-q3).*sin(q5).*8.191520442889917e-1+sin(q2-q3).*cos(q4).*cos(q5)-sin(q2-q3).*sin(q4).*sin(q5).*5.735764363510462e-1))+real(cos(q2-q3).*sin(q4).*(dq2-dq3)).*4.698463103929542e-1-imag(sin(q6).*(dq5.*cos(q2-q3).*cos(q5).*(-8.191520442889917e-1)+sin(q2-q3).*sin(q5).*(dq2-dq3).*8.191520442889917e-1+dq4.*sin(q2-q3).*cos(q4).*sin(q5).*5.735764363510462e-1+dq4.*sin(q2-q3).*cos(q5).*sin(q4)+dq5.*sin(q2-q3).*cos(q4).*sin(q5)+dq5.*sin(q2-q3).*cos(q5).*sin(q4).*5.735764363510462e-1-cos(q2-q3).*cos(q4).*cos(q5).*(dq2-dq3)+cos(q2-q3).*sin(q4).*sin(q5).*(dq2-dq3).*5.735764363510462e-1))+real(dq5.*sin(q5).*(cos(q2-q3).*8.191520442889917e-1-sin(q2-q3).*sin(q4).*5.735764363510462e-1)).*8.191520442889917e-1-real(sin(q2-q3).*(dq2-dq3)).*3.289899283371657e-1+imag(cos(q6).*(cos(q5).*(sin(q2-q3).*(dq2-dq3).*8.191520442889917e-1+dq4.*sin(q2-q3).*cos(q4).*5.735764363510462e-1+cos(q2-q3).*sin(q4).*(dq2-dq3).*5.735764363510462e-1).*5.735764363510462e-1+sin(q2-q3).*(dq2-dq3).*4.698463103929542e-1-dq4.*sin(q2-q3).*cos(q4).*6.710100716628342e-1-cos(q2-q3).*sin(q4).*(dq2-dq3).*6.710100716628342e-1+dq5.*sin(q5).*(cos(q2-q3).*8.191520442889917e-1-sin(q2-q3).*sin(q4).*5.735764363510462e-1).*5.735764363510462e-1+dq5.*sin(q2-q3).*cos(q4).*cos(q5).*5.735764363510462e-1-dq4.*sin(q2-q3).*sin(q4).*sin(q5).*5.735764363510462e-1+cos(q2-q3).*cos(q4).*sin(q5).*(dq2-dq3).*5.735764363510462e-1))+imag(dq6.*sin(q6).*(cos(q2-q3).*4.698463103929542e-1+sin(q2-q3).*sin(q4).*6.710100716628342e-1+cos(q5).*(cos(q2-q3).*8.191520442889917e-1-sin(q2-q3).*sin(q4).*5.735764363510462e-1).*5.735764363510462e-1-sin(q2-q3).*cos(q4).*sin(q5).*5.735764363510462e-1))+real(cos(q5).*(sin(q2-q3).*(dq2-dq3).*8.191520442889917e-1+dq4.*sin(q2-q3).*cos(q4).*5.735764363510462e-1+cos(q2-q3).*sin(q4).*(dq2-dq3).*5.735764363510462e-1)).*8.191520442889917e-1+real(dq5.*sin(q2-q3).*cos(q4).*cos(q5)).*8.191520442889917e-1-real(dq4.*sin(q2-q3).*sin(q4).*sin(q5)).*8.191520442889917e-1+real(cos(q2-q3).*cos(q4).*sin(q5).*(dq2-dq3)).*8.191520442889917e-1+real(dq4.*sin(q2-q3).*cos(q4)).*4.698463103929542e-1).*2.0).*(real(cos(q2-q3)).*3.289899283371657e-1+real(sin(q2-q3).*cos(q4).*sin(q5)).*8.191520442889917e-1+real(sin(q2-q3).*sin(q4)).*4.698463103929542e-1+imag(sin(q6).*(cos(q2-q3).*sin(q5).*8.191520442889917e-1+sin(q2-q3).*cos(q4).*cos(q5)-sin(q2-q3).*sin(q4).*sin(q5).*5.735764363510462e-1))-real(cos(q5).*(cos(q2-q3).*8.191520442889917e-1-sin(q2-q3).*sin(q4).*5.735764363510462e-1)).*8.191520442889917e-1-imag(cos(q6).*(cos(q2-q3).*4.698463103929542e-1+sin(q2-q3).*sin(q4).*6.710100716628342e-1+cos(q5).*(cos(q2-q3).*8.191520442889917e-1-sin(q2-q3).*sin(q4).*5.735764363510462e-1).*5.735764363510462e-1-sin(q2-q3).*cos(q4).*sin(q5).*5.735764363510462e-1))).^2+(((imag(sin(q2-q3)).*(-3.289899283371657e-1)+imag(cos(q2-q3).*cos(q4).*sin(q5)).*8.191520442889917e-1+imag(cos(q2-q3).*sin(q4)).*4.698463103929542e-1+real(sin(q6).*(sin(q2-q3).*sin(q5).*8.191520442889917e-1-cos(q2-q3).*cos(q4).*cos(q5)+cos(q2-q3).*sin(q4).*sin(q5).*5.735764363510462e-1))+imag(cos(q5).*(sin(q2-q3).*8.191520442889917e-1+cos(q2-q3).*sin(q4).*5.735764363510462e-1)).*8.191520442889917e-1-real(cos(q6).*(sin(q2-q3).*4.698463103929542e-1-cos(q2-q3).*sin(q4).*6.710100716628342e-1+cos(q5).*(sin(q2-q3).*8.191520442889917e-1+cos(q2-q3).*sin(q4).*5.735764363510462e-1).*5.735764363510462e-1+cos(q2-q3).*cos(q4).*sin(q5).*5.735764363510462e-1)))./(real(cos(q2-q3)).*3.289899283371657e-1+real(sin(q2-q3).*cos(q4).*sin(q5)).*8.191520442889917e-1+real(sin(q2-q3).*sin(q4)).*4.698463103929542e-1+imag(sin(q6).*(cos(q2-q3).*sin(q5).*8.191520442889917e-1+sin(q2-q3).*cos(q4).*cos(q5)-sin(q2-q3).*sin(q4).*sin(q5).*5.735764363510462e-1))-real(cos(q5).*(cos(q2-q3).*8.191520442889917e-1-sin(q2-q3).*sin(q4).*5.735764363510462e-1)).*8.191520442889917e-1-imag(cos(q6).*(cos(q2-q3).*4.698463103929542e-1+sin(q2-q3).*sin(q4).*6.710100716628342e-1+cos(q5).*(cos(q2-q3).*8.191520442889917e-1-sin(q2-q3).*sin(q4).*5.735764363510462e-1).*5.735764363510462e-1-sin(q2-q3).*cos(q4).*sin(q5).*5.735764363510462e-1)))-(real(sin(q2-q3)).*(-3.289899283371657e-1)+real(cos(q2-q3).*cos(q4).*sin(q5)).*8.191520442889917e-1+real(cos(q2-q3).*sin(q4)).*4.698463103929542e-1-imag(sin(q6).*(sin(q2-q3).*sin(q5).*8.191520442889917e-1-cos(q2-q3).*cos(q4).*cos(q5)+cos(q2-q3).*sin(q4).*sin(q5).*5.735764363510462e-1))+real(cos(q5).*(sin(q2-q3).*8.191520442889917e-1+cos(q2-q3).*sin(q4).*5.735764363510462e-1)).*8.191520442889917e-1+imag(cos(q6).*(sin(q2-q3).*4.698463103929542e-1-cos(q2-q3).*sin(q4).*6.710100716628342e-1+cos(q5).*(sin(q2-q3).*8.191520442889917e-1+cos(q2-q3).*sin(q4).*5.735764363510462e-1).*5.735764363510462e-1+cos(q2-q3).*cos(q4).*sin(q5).*5.735764363510462e-1))).*(real(cos(q6).*(cos(q2-q3).*4.698463103929542e-1+sin(q2-q3).*sin(q4).*6.710100716628342e-1+cos(q5).*(cos(q2-q3).*8.191520442889917e-1-sin(q2-q3).*sin(q4).*5.735764363510462e-1).*5.735764363510462e-1-sin(q2-q3).*cos(q4).*sin(q5).*5.735764363510462e-1))+imag(cos(q2-q3)).*3.289899283371657e-1+imag(sin(q2-q3).*cos(q4).*sin(q5)).*8.191520442889917e-1+imag(sin(q2-q3).*sin(q4)).*4.698463103929542e-1-real(sin(q6).*(cos(q2-q3).*sin(q5).*8.191520442889917e-1+sin(q2-q3).*cos(q4).*cos(q5)-sin(q2-q3).*sin(q4).*sin(q5).*5.735764363510462e-1))-imag(cos(q5).*(cos(q2-q3).*8.191520442889917e-1-sin(q2-q3).*sin(q4).*5.735764363510462e-1)).*8.191520442889917e-1).*1.0./(real(cos(q2-q3)).*3.289899283371657e-1+real(sin(q2-q3).*cos(q4).*sin(q5)).*8.191520442889917e-1+real(sin(q2-q3).*sin(q4)).*4.698463103929542e-1+imag(sin(q6).*(cos(q2-q3).*sin(q5).*8.191520442889917e-1+sin(q2-q3).*cos(q4).*cos(q5)-sin(q2-q3).*sin(q4).*sin(q5).*5.735764363510462e-1))-real(cos(q5).*(cos(q2-q3).*8.191520442889917e-1-sin(q2-q3).*sin(q4).*5.735764363510462e-1)).*8.191520442889917e-1-imag(cos(q6).*(cos(q2-q3).*4.698463103929542e-1+sin(q2-q3).*sin(q4).*6.710100716628342e-1+cos(q5).*(cos(q2-q3).*8.191520442889917e-1-sin(q2-q3).*sin(q4).*5.735764363510462e-1).*5.735764363510462e-1-sin(q2-q3).*cos(q4).*sin(q5).*5.735764363510462e-1))).^2).*(real(cos(q2-q3)).*3.289899283371657e-1+real(sin(q2-q3).*cos(q4).*sin(q5)).*8.191520442889917e-1+real(sin(q2-q3).*sin(q4)).*4.698463103929542e-1+imag(sin(q6).*(cos(q2-q3).*sin(q5).*8.191520442889917e-1+sin(q2-q3).*cos(q4).*cos(q5)-sin(q2-q3).*sin(q4).*sin(q5).*5.735764363510462e-1))-real(cos(q5).*(cos(q2-q3).*8.191520442889917e-1-sin(q2-q3).*sin(q4).*5.735764363510462e-1)).*8.191520442889917e-1-imag(cos(q6).*(cos(q2-q3).*4.698463103929542e-1+sin(q2-q3).*sin(q4).*6.710100716628342e-1+cos(q5).*(cos(q2-q3).*8.191520442889917e-1-sin(q2-q3).*sin(q4).*5.735764363510462e-1).*5.735764363510462e-1-sin(q2-q3).*cos(q4).*sin(q5).*5.735764363510462e-1))).*(imag(dq6.*cos(q6).*(cos(q2-q3).*sin(q5).*8.191520442889917e-1+sin(q2-q3).*cos(q4).*cos(q5)-sin(q2-q3).*sin(q4).*sin(q5).*5.735764363510462e-1))+real(cos(q2-q3).*sin(q4).*(dq2-dq3)).*4.698463103929542e-1-imag(sin(q6).*(dq5.*cos(q2-q3).*cos(q5).*(-8.191520442889917e-1)+sin(q2-q3).*sin(q5).*(dq2-dq3).*8.191520442889917e-1+dq4.*sin(q2-q3).*cos(q4).*sin(q5).*5.735764363510462e-1+dq4.*sin(q2-q3).*cos(q5).*sin(q4)+dq5.*sin(q2-q3).*cos(q4).*sin(q5)+dq5.*sin(q2-q3).*cos(q5).*sin(q4).*5.735764363510462e-1-cos(q2-q3).*cos(q4).*cos(q5).*(dq2-dq3)+cos(q2-q3).*sin(q4).*sin(q5).*(dq2-dq3).*5.735764363510462e-1))+real(dq5.*sin(q5).*(cos(q2-q3).*8.191520442889917e-1-sin(q2-q3).*sin(q4).*5.735764363510462e-1)).*8.191520442889917e-1-real(sin(q2-q3).*(dq2-dq3)).*3.289899283371657e-1+imag(cos(q6).*(cos(q5).*(sin(q2-q3).*(dq2-dq3).*8.191520442889917e-1+dq4.*sin(q2-q3).*cos(q4).*5.735764363510462e-1+cos(q2-q3).*sin(q4).*(dq2-dq3).*5.735764363510462e-1).*5.735764363510462e-1+sin(q2-q3).*(dq2-dq3).*4.698463103929542e-1-dq4.*sin(q2-q3).*cos(q4).*6.710100716628342e-1-cos(q2-q3).*sin(q4).*(dq2-dq3).*6.710100716628342e-1+dq5.*sin(q5).*(cos(q2-q3).*8.191520442889917e-1-sin(q2-q3).*sin(q4).*5.735764363510462e-1).*5.735764363510462e-1+dq5.*sin(q2-q3).*cos(q4).*cos(q5).*5.735764363510462e-1-dq4.*sin(q2-q3).*sin(q4).*sin(q5).*5.735764363510462e-1+cos(q2-q3).*cos(q4).*sin(q5).*(dq2-dq3).*5.735764363510462e-1))+imag(dq6.*sin(q6).*(cos(q2-q3).*4.698463103929542e-1+sin(q2-q3).*sin(q4).*6.710100716628342e-1+cos(q5).*(cos(q2-q3).*8.191520442889917e-1-sin(q2-q3).*sin(q4).*5.735764363510462e-1).*5.735764363510462e-1-sin(q2-q3).*cos(q4).*sin(q5).*5.735764363510462e-1))+real(cos(q5).*(sin(q2-q3).*(dq2-dq3).*8.191520442889917e-1+dq4.*sin(q2-q3).*cos(q4).*5.735764363510462e-1+cos(q2-q3).*sin(q4).*(dq2-dq3).*5.735764363510462e-1)).*8.191520442889917e-1+real(dq5.*sin(q2-q3).*cos(q4).*cos(q5)).*8.191520442889917e-1-real(dq4.*sin(q2-q3).*sin(q4).*sin(q5)).*8.191520442889917e-1+real(cos(q2-q3).*cos(q4).*sin(q5).*(dq2-dq3)).*8.191520442889917e-1+real(dq4.*sin(q2-q3).*cos(q4)).*4.698463103929542e-1).*2.0)./((real(cos(q6).*(cos(q2-q3).*4.698463103929542e-1+sin(q2-q3).*sin(q4).*6.710100716628342e-1+cos(q5).*(cos(q2-q3).*8.191520442889917e-1-sin(q2-q3).*sin(q4).*5.735764363510462e-1).*5.735764363510462e-1-sin(q2-q3).*cos(q4).*sin(q5).*5.735764363510462e-1))+imag(cos(q2-q3)).*3.289899283371657e-1+imag(sin(q2-q3).*cos(q4).*sin(q5)).*8.191520442889917e-1+imag(sin(q2-q3).*sin(q4)).*4.698463103929542e-1-real(sin(q6).*(cos(q2-q3).*sin(q5).*8.191520442889917e-1+sin(q2-q3).*cos(q4).*cos(q5)-sin(q2-q3).*sin(q4).*sin(q5).*5.735764363510462e-1))-imag(cos(q5).*(cos(q2-q3).*8.191520442889917e-1-sin(q2-q3).*sin(q4).*5.735764363510462e-1)).*8.191520442889917e-1).^2+(real(cos(q2-q3)).*3.289899283371657e-1+real(sin(q2-q3).*cos(q4).*sin(q5)).*8.191520442889917e-1+real(sin(q2-q3).*sin(q4)).*4.698463103929542e-1+imag(sin(q6).*(cos(q2-q3).*sin(q5).*8.191520442889917e-1+sin(q2-q3).*cos(q4).*cos(q5)-sin(q2-q3).*sin(q4).*sin(q5).*5.735764363510462e-1))-real(cos(q5).*(cos(q2-q3).*8.191520442889917e-1-sin(q2-q3).*sin(q4).*5.735764363510462e-1)).*8.191520442889917e-1-imag(cos(q6).*(cos(q2-q3).*4.698463103929542e-1+sin(q2-q3).*sin(q4).*6.710100716628342e-1+cos(q5).*(cos(q2-q3).*8.191520442889917e-1-sin(q2-q3).*sin(q4).*5.735764363510462e-1).*5.735764363510462e-1-sin(q2-q3).*cos(q4).*sin(q5).*5.735764363510462e-1))).^2),cos(q1).*cos(q5).*(sin(q2-q3).*(dq2-dq3).*7.378265682839366e15+dq4.*sin(q2-q3).*cos(q4).*5.166317250038137e15+cos(q2-q3).*sin(q4).*(dq2-dq3).*5.166317250038137e15).*(-1.915122192329876e-17)+dq1.*cos(q2-q3).*sin(q1).*3.665070063091676e-1+sin(q2-q3).*cos(q1).*(dq2-dq3).*3.665070063091676e-1-dq4.*sin(q2-q3).*cos(q1).*cos(q4).*1.675571321083729e-1+dq1.*sin(q2-q3).*sin(q1).*sin(q4).*1.675571321083729e-1-cos(q2-q3).*cos(q1).*sin(q4).*(dq2-dq3).*1.675571321083729e-1-dq1.*cos(q5).*sin(q1).*(cos(q2-q3).*7.378265682839366e15-sin(q2-q3).*sin(q4).*5.166317250038137e15).*1.915122192329876e-17-dq5.*cos(q1).*sin(q5).*(cos(q2-q3).*7.378265682839366e15-sin(q2-q3).*sin(q4).*5.166317250038137e15).*1.915122192329876e-17-dq5.*sin(q2-q3).*cos(q1).*cos(q4).*cos(q5).*1.724988718349159e-1+dq1.*sin(q2-q3).*cos(q4).*sin(q1).*sin(q5).*1.724988718349159e-1+dq4.*sin(q2-q3).*cos(q1).*sin(q4).*sin(q5).*1.724988718349159e-1-cos(q2-q3).*cos(q1).*cos(q4).*sin(q5).*(dq2-dq3).*1.724988718349159e-1,cos(q5).*sin(q1).*(sin(q2-q3).*(dq2-dq3).*7.378265682839366e15+dq4.*sin(q2-q3).*cos(q4).*5.166317250038137e15+cos(q2-q3).*sin(q4).*(dq2-dq3).*5.166317250038137e15).*(-1.915122192329876e-17)-dq1.*cos(q2-q3).*cos(q1).*3.665070063091676e-1+sin(q2-q3).*sin(q1).*(dq2-dq3).*3.665070063091676e-1-dq1.*sin(q2-q3).*cos(q1).*sin(q4).*1.675571321083729e-1-dq4.*sin(q2-q3).*cos(q4).*sin(q1).*1.675571321083729e-1-cos(q2-q3).*sin(q1).*sin(q4).*(dq2-dq3).*1.675571321083729e-1+dq1.*cos(q1).*cos(q5).*(cos(q2-q3).*7.378265682839366e15-sin(q2-q3).*sin(q4).*5.166317250038137e15).*1.915122192329876e-17-dq5.*sin(q1).*sin(q5).*(cos(q2-q3).*7.378265682839366e15-sin(q2-q3).*sin(q4).*5.166317250038137e15).*1.915122192329876e-17-dq1.*sin(q2-q3).*cos(q1).*cos(q4).*sin(q5).*1.724988718349159e-1-dq5.*sin(q2-q3).*cos(q4).*cos(q5).*sin(q1).*1.724988718349159e-1+dq4.*sin(q2-q3).*sin(q1).*sin(q4).*sin(q5).*1.724988718349159e-1-cos(q2-q3).*cos(q4).*sin(q1).*sin(q5).*(dq2-dq3).*1.724988718349159e-1,cos(q5).*(cos(q2-q3).*(dq2-dq3).*8.191520442889917e-1+dq4.*cos(q2-q3).*cos(q4).*5.735764363510462e-1-sin(q2-q3).*sin(q4).*(dq2-dq3).*5.735764363510462e-1).*1.724988718349159e-1-cos(q2-q3).*(dq2-dq3).*3.665070063091676e-1+dq4.*cos(q2-q3).*cos(q4).*1.675571321083729e-1-sin(q2-q3).*sin(q4).*(dq2-dq3).*1.675571321083729e-1-dq5.*sin(q5).*(sin(q2-q3).*8.191520442889917e-1+cos(q2-q3).*sin(q4).*5.735764363510462e-1).*1.724988718349159e-1+dq5.*cos(q2-q3).*cos(q4).*cos(q5).*1.724988718349159e-1-dq4.*cos(q2-q3).*sin(q4).*sin(q5).*1.724988718349159e-1-sin(q2-q3).*cos(q4).*sin(q5).*(dq2-dq3).*1.724988718349159e-1,-((real(sin(q6).*(cos(q4).*sin(q1).*(-6.710100716628342e-1)+cos(q5).*(cos(q4).*sin(q1).*5.735764363510462e-1+sin(q2-q3).*cos(q1).*8.191520442889917e-1+cos(q2-q3).*cos(q1).*sin(q4).*5.735764363510462e-1).*5.735764363510462e-1+sin(q2-q3).*cos(q1).*4.698463103929542e-1+sin(q5).*(-sin(q1).*sin(q4)+cos(q1).*cos(q2).*cos(q3).*cos(q4)+cos(q1).*cos(q4).*sin(q2).*sin(q3)).*5.735764363510462e-1-cos(q2-q3).*cos(q1).*sin(q4).*6.710100716628342e-1))+real(cos(q6).*(sin(q5).*(cos(q4).*sin(q1).*5.735764363510462e-1+sin(q2-q3).*cos(q1).*8.191520442889917e-1+cos(q2-q3).*cos(q1).*sin(q4).*5.735764363510462e-1)-cos(q5).*(-sin(q1).*sin(q4)+cos(q1).*cos(q2).*cos(q3).*cos(q4)+cos(q1).*cos(q4).*sin(q2).*sin(q3))))-imag(sin(q6).*(cos(q1).*cos(q4).*6.710100716628342e-1+cos(q5).*(cos(q1).*cos(q4).*(-5.735764363510462e-1)+sin(q2-q3).*sin(q1).*8.191520442889917e-1+cos(q2-q3).*sin(q1).*sin(q4).*5.735764363510462e-1).*5.735764363510462e-1+sin(q2-q3).*sin(q1).*4.698463103929542e-1+sin(q5).*(cos(q1).*sin(q4)+cos(q2).*cos(q3).*cos(q4).*sin(q1)+cos(q4).*sin(q1).*sin(q2).*sin(q3)).*5.735764363510462e-1-cos(q2-q3).*sin(q1).*sin(q4).*6.710100716628342e-1))-imag(cos(q6).*(sin(q5).*(cos(q1).*cos(q4).*(-5.735764363510462e-1)+sin(q2-q3).*sin(q1).*8.191520442889917e-1+cos(q2-q3).*sin(q1).*sin(q4).*5.735764363510462e-1)-cos(q5).*(cos(q1).*sin(q4)+cos(q2).*cos(q3).*cos(q4).*sin(q1)+cos(q4).*sin(q1).*sin(q2).*sin(q3))))).^2.*((imag(cos(q6).*(-sin(q5).*(dq1.*cos(q2-q3).*sin(q1).*8.191520442889917e-1+sin(q2-q3).*cos(q1).*(dq2-dq3).*8.191520442889917e-1+dq4.*sin(q2-q3).*cos(q1).*cos(q4).*5.735764363510462e-1-dq1.*sin(q2-q3).*sin(q1).*sin(q4).*5.735764363510462e-1+cos(q2-q3).*cos(q1).*sin(q4).*(dq2-dq3).*5.735764363510462e-1)+cos(q5).*(dq2.*cos(q1).*cos(q2).*cos(q3).*cos(q4)-dq3.*cos(q1).*cos(q2).*cos(q3).*cos(q4)+dq1.*cos(q2).*cos(q4).*sin(q1).*sin(q3)-dq1.*cos(q3).*cos(q4).*sin(q1).*sin(q2)+dq2.*cos(q1).*cos(q4).*sin(q2).*sin(q3)-dq3.*cos(q1).*cos(q4).*sin(q2).*sin(q3)+dq4.*cos(q1).*cos(q2).*sin(q3).*sin(q4)-dq4.*cos(q1).*cos(q3).*sin(q2).*sin(q4))+dq5.*cos(q5).*(cos(q2-q3).*cos(q1).*8.191520442889917e-1-sin(q2-q3).*cos(q1).*sin(q4).*5.735764363510462e-1)+dq5.*sin(q5).*(cos(q1).*cos(q2).*cos(q4).*sin(q3)-cos(q1).*cos(q3).*cos(q4).*sin(q2))))+real(dq6.*cos(q6).*(cos(q5).*(cos(q2-q3).*sin(q1).*8.191520442889917e-1-sin(q2-q3).*sin(q1).*sin(q4).*5.735764363510462e-1).*5.735764363510462e-1+sin(q5).*(cos(q2).*cos(q4).*sin(q1).*sin(q3)-cos(q3).*cos(q4).*sin(q1).*sin(q2)).*5.735764363510462e-1+cos(q2-q3).*sin(q1).*4.698463103929542e-1+sin(q2-q3).*sin(q1).*sin(q4).*6.710100716628342e-1))+real(sin(q6).*(cos(q5).*(dq1.*cos(q2-q3).*cos(q1).*(-8.191520442889917e-1)+sin(q2-q3).*sin(q1).*(dq2-dq3).*8.191520442889917e-1+dq1.*sin(q2-q3).*cos(q1).*sin(q4).*5.735764363510462e-1+dq4.*sin(q2-q3).*cos(q4).*sin(q1).*5.735764363510462e-1+cos(q2-q3).*sin(q1).*sin(q4).*(dq2-dq3).*5.735764363510462e-1).*(-5.735764363510462e-1)+sin(q5).*(dq1.*cos(q1).*cos(q2).*cos(q4).*sin(q3)-dq1.*cos(q1).*cos(q3).*cos(q4).*sin(q2)-dq2.*cos(q2).*cos(q3).*cos(q4).*sin(q1)+dq3.*cos(q2).*cos(q3).*cos(q4).*sin(q1)-dq2.*cos(q4).*sin(q1).*sin(q2).*sin(q3)+dq3.*cos(q4).*sin(q1).*sin(q2).*sin(q3)-dq4.*cos(q2).*sin(q1).*sin(q3).*sin(q4)+dq4.*cos(q3).*sin(q1).*sin(q2).*sin(q4)).*5.735764363510462e-1+dq5.*cos(q5).*(cos(q2).*cos(q4).*sin(q1).*sin(q3)-cos(q3).*cos(q4).*sin(q1).*sin(q2)).*5.735764363510462e-1+dq1.*cos(q2-q3).*cos(q1).*4.698463103929542e-1-dq5.*sin(q5).*(cos(q2-q3).*sin(q1).*8.191520442889917e-1-sin(q2-q3).*sin(q1).*sin(q4).*5.735764363510462e-1).*5.735764363510462e-1-sin(q2-q3).*sin(q1).*(dq2-dq3).*4.698463103929542e-1+dq1.*sin(q2-q3).*cos(q1).*sin(q4).*6.710100716628342e-1+dq4.*sin(q2-q3).*cos(q4).*sin(q1).*6.710100716628342e-1+cos(q2-q3).*sin(q1).*sin(q4).*(dq2-dq3).*6.710100716628342e-1))-imag(sin(q6).*(sin(q5).*(dq2.*cos(q1).*cos(q2).*cos(q3).*cos(q4)-dq3.*cos(q1).*cos(q2).*cos(q3).*cos(q4)+dq1.*cos(q2).*cos(q4).*sin(q1).*sin(q3)-dq1.*cos(q3).*cos(q4).*sin(q1).*sin(q2)+dq2.*cos(q1).*cos(q4).*sin(q2).*sin(q3)-dq3.*cos(q1).*cos(q4).*sin(q2).*sin(q3)+dq4.*cos(q1).*cos(q2).*sin(q3).*sin(q4)-dq4.*cos(q1).*cos(q3).*sin(q2).*sin(q4)).*5.735764363510462e-1+cos(q5).*(dq1.*cos(q2-q3).*sin(q1).*8.191520442889917e-1+sin(q2-q3).*cos(q1).*(dq2-dq3).*8.191520442889917e-1+dq4.*sin(q2-q3).*cos(q1).*cos(q4).*5.735764363510462e-1-dq1.*sin(q2-q3).*sin(q1).*sin(q4).*5.735764363510462e-1+cos(q2-q3).*cos(q1).*sin(q4).*(dq2-dq3).*5.735764363510462e-1).*5.735764363510462e-1-dq5.*cos(q5).*(cos(q1).*cos(q2).*cos(q4).*sin(q3)-cos(q1).*cos(q3).*cos(q4).*sin(q2)).*5.735764363510462e-1+dq5.*sin(q5).*(cos(q2-q3).*cos(q1).*8.191520442889917e-1-sin(q2-q3).*cos(q1).*sin(q4).*5.735764363510462e-1).*5.735764363510462e-1+dq1.*cos(q2-q3).*sin(q1).*4.698463103929542e-1+sin(q2-q3).*cos(q1).*(dq2-dq3).*4.698463103929542e-1-dq4.*sin(q2-q3).*cos(q1).*cos(q4).*6.710100716628342e-1+dq1.*sin(q2-q3).*sin(q1).*sin(q4).*6.710100716628342e-1-cos(q2-q3).*cos(q1).*sin(q4).*(dq2-dq3).*6.710100716628342e-1))+imag(dq6.*sin(q6).*(cos(q5).*(cos(q1).*cos(q2).*cos(q4).*sin(q3)-cos(q1).*cos(q3).*cos(q4).*sin(q2))-sin(q5).*(cos(q2-q3).*cos(q1).*8.191520442889917e-1-sin(q2-q3).*cos(q1).*sin(q4).*5.735764363510462e-1)))-real(cos(q6).*(sin(q5).*(dq1.*cos(q2-q3).*cos(q1).*(-8.191520442889917e-1)+sin(q2-q3).*sin(q1).*(dq2-dq3).*8.191520442889917e-1+dq1.*sin(q2-q3).*cos(q1).*sin(q4).*5.735764363510462e-1+dq4.*sin(q2-q3).*cos(q4).*sin(q1).*5.735764363510462e-1+cos(q2-q3).*sin(q1).*sin(q4).*(dq2-dq3).*5.735764363510462e-1)+cos(q5).*(dq1.*cos(q1).*cos(q2).*cos(q4).*sin(q3)-dq1.*cos(q1).*cos(q3).*cos(q4).*sin(q2)-dq2.*cos(q2).*cos(q3).*cos(q4).*sin(q1)+dq3.*cos(q2).*cos(q3).*cos(q4).*sin(q1)-dq2.*cos(q4).*sin(q1).*sin(q2).*sin(q3)+dq3.*cos(q4).*sin(q1).*sin(q2).*sin(q3)-dq4.*cos(q2).*sin(q1).*sin(q3).*sin(q4)+dq4.*cos(q3).*sin(q1).*sin(q2).*sin(q4))-dq5.*cos(q5).*(cos(q2-q3).*sin(q1).*8.191520442889917e-1-sin(q2-q3).*sin(q1).*sin(q4).*5.735764363510462e-1)-dq5.*sin(q5).*(cos(q2).*cos(q4).*sin(q1).*sin(q3)-cos(q3).*cos(q4).*sin(q1).*sin(q2))))+imag(dq6.*cos(q6).*(cos(q5).*(cos(q2-q3).*cos(q1).*8.191520442889917e-1-sin(q2-q3).*cos(q1).*sin(q4).*5.735764363510462e-1).*5.735764363510462e-1+sin(q5).*(cos(q1).*cos(q2).*cos(q4).*sin(q3)-cos(q1).*cos(q3).*cos(q4).*sin(q2)).*5.735764363510462e-1+cos(q2-q3).*cos(q1).*4.698463103929542e-1+sin(q2-q3).*cos(q1).*sin(q4).*6.710100716628342e-1))+real(dq6.*sin(q6).*(cos(q5).*(cos(q2).*cos(q4).*sin(q1).*sin(q3)-cos(q3).*cos(q4).*sin(q1).*sin(q2))-sin(q5).*(cos(q2-q3).*sin(q1).*8.191520442889917e-1-sin(q2-q3).*sin(q1).*sin(q4).*5.735764363510462e-1))))./(real(sin(q6).*(cos(q4).*sin(q1).*(-6.710100716628342e-1)+cos(q5).*(cos(q4).*sin(q1).*5.735764363510462e-1+sin(q2-q3).*cos(q1).*8.191520442889917e-1+cos(q2-q3).*cos(q1).*sin(q4).*5.735764363510462e-1).*5.735764363510462e-1+sin(q2-q3).*cos(q1).*4.698463103929542e-1+sin(q5).*(-sin(q1).*sin(q4)+cos(q1).*cos(q2).*cos(q3).*cos(q4)+cos(q1).*cos(q4).*sin(q2).*sin(q3)).*5.735764363510462e-1-cos(q2-q3).*cos(q1).*sin(q4).*6.710100716628342e-1))+real(cos(q6).*(sin(q5).*(cos(q4).*sin(q1).*5.735764363510462e-1+sin(q2-q3).*cos(q1).*8.191520442889917e-1+cos(q2-q3).*cos(q1).*sin(q4).*5.735764363510462e-1)-cos(q5).*(-sin(q1).*sin(q4)+cos(q1).*cos(q2).*cos(q3).*cos(q4)+cos(q1).*cos(q4).*sin(q2).*sin(q3))))-imag(sin(q6).*(cos(q1).*cos(q4).*6.710100716628342e-1+cos(q5).*(cos(q1).*cos(q4).*(-5.735764363510462e-1)+sin(q2-q3).*sin(q1).*8.191520442889917e-1+cos(q2-q3).*sin(q1).*sin(q4).*5.735764363510462e-1).*5.735764363510462e-1+sin(q2-q3).*sin(q1).*4.698463103929542e-1+sin(q5).*(cos(q1).*sin(q4)+cos(q2).*cos(q3).*cos(q4).*sin(q1)+cos(q4).*sin(q1).*sin(q2).*sin(q3)).*5.735764363510462e-1-cos(q2-q3).*sin(q1).*sin(q4).*6.710100716628342e-1))-imag(cos(q6).*(sin(q5).*(cos(q1).*cos(q4).*(-5.735764363510462e-1)+sin(q2-q3).*sin(q1).*8.191520442889917e-1+cos(q2-q3).*sin(q1).*sin(q4).*5.735764363510462e-1)-cos(q5).*(cos(q1).*sin(q4)+cos(q2).*cos(q3).*cos(q4).*sin(q1)+cos(q4).*sin(q1).*sin(q2).*sin(q3)))))+1.0./(real(sin(q6).*(cos(q4).*sin(q1).*(-6.710100716628342e-1)+cos(q5).*(cos(q4).*sin(q1).*5.735764363510462e-1+sin(q2-q3).*cos(q1).*8.191520442889917e-1+cos(q2-q3).*cos(q1).*sin(q4).*5.735764363510462e-1).*5.735764363510462e-1+sin(q2-q3).*cos(q1).*4.698463103929542e-1+sin(q5).*(-sin(q1).*sin(q4)+cos(q1).*cos(q2).*cos(q3).*cos(q4)+cos(q1).*cos(q4).*sin(q2).*sin(q3)).*5.735764363510462e-1-cos(q2-q3).*cos(q1).*sin(q4).*6.710100716628342e-1))+real(cos(q6).*(sin(q5).*(cos(q4).*sin(q1).*5.735764363510462e-1+sin(q2-q3).*cos(q1).*8.191520442889917e-1+cos(q2-q3).*cos(q1).*sin(q4).*5.735764363510462e-1)-cos(q5).*(-sin(q1).*sin(q4)+cos(q1).*cos(q2).*cos(q3).*cos(q4)+cos(q1).*cos(q4).*sin(q2).*sin(q3))))-imag(sin(q6).*(cos(q1).*cos(q4).*6.710100716628342e-1+cos(q5).*(cos(q1).*cos(q4).*(-5.735764363510462e-1)+sin(q2-q3).*sin(q1).*8.191520442889917e-1+cos(q2-q3).*sin(q1).*sin(q4).*5.735764363510462e-1).*5.735764363510462e-1+sin(q2-q3).*sin(q1).*4.698463103929542e-1+sin(q5).*(cos(q1).*sin(q4)+cos(q2).*cos(q3).*cos(q4).*sin(q1)+cos(q4).*sin(q1).*sin(q2).*sin(q3)).*5.735764363510462e-1-cos(q2-q3).*sin(q1).*sin(q4).*6.710100716628342e-1))-imag(cos(q6).*(sin(q5).*(cos(q1).*cos(q4).*(-5.735764363510462e-1)+sin(q2-q3).*sin(q1).*8.191520442889917e-1+cos(q2-q3).*sin(q1).*sin(q4).*5.735764363510462e-1)-cos(q5).*(cos(q1).*sin(q4)+cos(q2).*cos(q3).*cos(q4).*sin(q1)+cos(q4).*sin(q1).*sin(q2).*sin(q3))))).^2.*(imag(sin(q6).*(cos(q4).*sin(q1).*(-6.710100716628342e-1)+cos(q5).*(cos(q4).*sin(q1).*5.735764363510462e-1+sin(q2-q3).*cos(q1).*8.191520442889917e-1+cos(q2-q3).*cos(q1).*sin(q4).*5.735764363510462e-1).*5.735764363510462e-1+sin(q2-q3).*cos(q1).*4.698463103929542e-1+sin(q5).*(-sin(q1).*sin(q4)+cos(q1).*cos(q2).*cos(q3).*cos(q4)+cos(q1).*cos(q4).*sin(q2).*sin(q3)).*5.735764363510462e-1-cos(q2-q3).*cos(q1).*sin(q4).*6.710100716628342e-1))+imag(cos(q6).*(sin(q5).*(cos(q4).*sin(q1).*5.735764363510462e-1+sin(q2-q3).*cos(q1).*8.191520442889917e-1+cos(q2-q3).*cos(q1).*sin(q4).*5.735764363510462e-1)-cos(q5).*(-sin(q1).*sin(q4)+cos(q1).*cos(q2).*cos(q3).*cos(q4)+cos(q1).*cos(q4).*sin(q2).*sin(q3))))+real(sin(q6).*(cos(q1).*cos(q4).*6.710100716628342e-1+cos(q5).*(cos(q1).*cos(q4).*(-5.735764363510462e-1)+sin(q2-q3).*sin(q1).*8.191520442889917e-1+cos(q2-q3).*sin(q1).*sin(q4).*5.735764363510462e-1).*5.735764363510462e-1+sin(q2-q3).*sin(q1).*4.698463103929542e-1+sin(q5).*(cos(q1).*sin(q4)+cos(q2).*cos(q3).*cos(q4).*sin(q1)+cos(q4).*sin(q1).*sin(q2).*sin(q3)).*5.735764363510462e-1-cos(q2-q3).*sin(q1).*sin(q4).*6.710100716628342e-1))+real(cos(q6).*(sin(q5).*(cos(q1).*cos(q4).*(-5.735764363510462e-1)+sin(q2-q3).*sin(q1).*8.191520442889917e-1+cos(q2-q3).*sin(q1).*sin(q4).*5.735764363510462e-1)-cos(q5).*(cos(q1).*sin(q4)+cos(q2).*cos(q3).*cos(q4).*sin(q1)+cos(q4).*sin(q1).*sin(q2).*sin(q3))))).*(imag(dq6.*cos(q6).*(cos(q5).*(cos(q2-q3).*sin(q1).*8.191520442889917e-1-sin(q2-q3).*sin(q1).*sin(q4).*5.735764363510462e-1).*5.735764363510462e-1+sin(q5).*(cos(q2).*cos(q4).*sin(q1).*sin(q3)-cos(q3).*cos(q4).*sin(q1).*sin(q2)).*5.735764363510462e-1+cos(q2-q3).*sin(q1).*4.698463103929542e-1+sin(q2-q3).*sin(q1).*sin(q4).*6.710100716628342e-1))+imag(sin(q6).*(cos(q5).*(dq1.*cos(q2-q3).*cos(q1).*(-8.191520442889917e-1)+sin(q2-q3).*sin(q1).*(dq2-dq3).*8.191520442889917e-1+dq1.*sin(q2-q3).*cos(q1).*sin(q4).*5.735764363510462e-1+dq4.*sin(q2-q3).*cos(q4).*sin(q1).*5.735764363510462e-1+cos(q2-q3).*sin(q1).*sin(q4).*(dq2-dq3).*5.735764363510462e-1).*(-5.735764363510462e-1)+sin(q5).*(dq1.*cos(q1).*cos(q2).*cos(q4).*sin(q3)-dq1.*cos(q1).*cos(q3).*cos(q4).*sin(q2)-dq2.*cos(q2).*cos(q3).*cos(q4).*sin(q1)+dq3.*cos(q2).*cos(q3).*cos(q4).*sin(q1)-dq2.*cos(q4).*sin(q1).*sin(q2).*sin(q3)+dq3.*cos(q4).*sin(q1).*sin(q2).*sin(q3)-dq4.*cos(q2).*sin(q1).*sin(q3).*sin(q4)+dq4.*cos(q3).*sin(q1).*sin(q2).*sin(q4)).*5.735764363510462e-1+dq5.*cos(q5).*(cos(q2).*cos(q4).*sin(q1).*sin(q3)-cos(q3).*cos(q4).*sin(q1).*sin(q2)).*5.735764363510462e-1+dq1.*cos(q2-q3).*cos(q1).*4.698463103929542e-1-dq5.*sin(q5).*(cos(q2-q3).*sin(q1).*8.191520442889917e-1-sin(q2-q3).*sin(q1).*sin(q4).*5.735764363510462e-1).*5.735764363510462e-1-sin(q2-q3).*sin(q1).*(dq2-dq3).*4.698463103929542e-1+dq1.*sin(q2-q3).*cos(q1).*sin(q4).*6.710100716628342e-1+dq4.*sin(q2-q3).*cos(q4).*sin(q1).*6.710100716628342e-1+cos(q2-q3).*sin(q1).*sin(q4).*(dq2-dq3).*6.710100716628342e-1))-real(cos(q6).*(-sin(q5).*(dq1.*cos(q2-q3).*sin(q1).*8.191520442889917e-1+sin(q2-q3).*cos(q1).*(dq2-dq3).*8.191520442889917e-1+dq4.*sin(q2-q3).*cos(q1).*cos(q4).*5.735764363510462e-1-dq1.*sin(q2-q3).*sin(q1).*sin(q4).*5.735764363510462e-1+cos(q2-q3).*cos(q1).*sin(q4).*(dq2-dq3).*5.735764363510462e-1)+cos(q5).*(dq2.*cos(q1).*cos(q2).*cos(q3).*cos(q4)-dq3.*cos(q1).*cos(q2).*cos(q3).*cos(q4)+dq1.*cos(q2).*cos(q4).*sin(q1).*sin(q3)-dq1.*cos(q3).*cos(q4).*sin(q1).*sin(q2)+dq2.*cos(q1).*cos(q4).*sin(q2).*sin(q3)-dq3.*cos(q1).*cos(q4).*sin(q2).*sin(q3)+dq4.*cos(q1).*cos(q2).*sin(q3).*sin(q4)-dq4.*cos(q1).*cos(q3).*sin(q2).*sin(q4))+dq5.*cos(q5).*(cos(q2-q3).*cos(q1).*8.191520442889917e-1-sin(q2-q3).*cos(q1).*sin(q4).*5.735764363510462e-1)+dq5.*sin(q5).*(cos(q1).*cos(q2).*cos(q4).*sin(q3)-cos(q1).*cos(q3).*cos(q4).*sin(q2))))+real(sin(q6).*(sin(q5).*(dq2.*cos(q1).*cos(q2).*cos(q3).*cos(q4)-dq3.*cos(q1).*cos(q2).*cos(q3).*cos(q4)+dq1.*cos(q2).*cos(q4).*sin(q1).*sin(q3)-dq1.*cos(q3).*cos(q4).*sin(q1).*sin(q2)+dq2.*cos(q1).*cos(q4).*sin(q2).*sin(q3)-dq3.*cos(q1).*cos(q4).*sin(q2).*sin(q3)+dq4.*cos(q1).*cos(q2).*sin(q3).*sin(q4)-dq4.*cos(q1).*cos(q3).*sin(q2).*sin(q4)).*5.735764363510462e-1+cos(q5).*(dq1.*cos(q2-q3).*sin(q1).*8.191520442889917e-1+sin(q2-q3).*cos(q1).*(dq2-dq3).*8.191520442889917e-1+dq4.*sin(q2-q3).*cos(q1).*cos(q4).*5.735764363510462e-1-dq1.*sin(q2-q3).*sin(q1).*sin(q4).*5.735764363510462e-1+cos(q2-q3).*cos(q1).*sin(q4).*(dq2-dq3).*5.735764363510462e-1).*5.735764363510462e-1-dq5.*cos(q5).*(cos(q1).*cos(q2).*cos(q4).*sin(q3)-cos(q1).*cos(q3).*cos(q4).*sin(q2)).*5.735764363510462e-1+dq5.*sin(q5).*(cos(q2-q3).*cos(q1).*8.191520442889917e-1-sin(q2-q3).*cos(q1).*sin(q4).*5.735764363510462e-1).*5.735764363510462e-1+dq1.*cos(q2-q3).*sin(q1).*4.698463103929542e-1+sin(q2-q3).*cos(q1).*(dq2-dq3).*4.698463103929542e-1-dq4.*sin(q2-q3).*cos(q1).*cos(q4).*6.710100716628342e-1+dq1.*sin(q2-q3).*sin(q1).*sin(q4).*6.710100716628342e-1-cos(q2-q3).*cos(q1).*sin(q4).*(dq2-dq3).*6.710100716628342e-1))-real(dq6.*sin(q6).*(cos(q5).*(cos(q1).*cos(q2).*cos(q4).*sin(q3)-cos(q1).*cos(q3).*cos(q4).*sin(q2))-sin(q5).*(cos(q2-q3).*cos(q1).*8.191520442889917e-1-sin(q2-q3).*cos(q1).*sin(q4).*5.735764363510462e-1)))-imag(cos(q6).*(sin(q5).*(dq1.*cos(q2-q3).*cos(q1).*(-8.191520442889917e-1)+sin(q2-q3).*sin(q1).*(dq2-dq3).*8.191520442889917e-1+dq1.*sin(q2-q3).*cos(q1).*sin(q4).*5.735764363510462e-1+dq4.*sin(q2-q3).*cos(q4).*sin(q1).*5.735764363510462e-1+cos(q2-q3).*sin(q1).*sin(q4).*(dq2-dq3).*5.735764363510462e-1)+cos(q5).*(dq1.*cos(q1).*cos(q2).*cos(q4).*sin(q3)-dq1.*cos(q1).*cos(q3).*cos(q4).*sin(q2)-dq2.*cos(q2).*cos(q3).*cos(q4).*sin(q1)+dq3.*cos(q2).*cos(q3).*cos(q4).*sin(q1)-dq2.*cos(q4).*sin(q1).*sin(q2).*sin(q3)+dq3.*cos(q4).*sin(q1).*sin(q2).*sin(q3)-dq4.*cos(q2).*sin(q1).*sin(q3).*sin(q4)+dq4.*cos(q3).*sin(q1).*sin(q2).*sin(q4))-dq5.*cos(q5).*(cos(q2-q3).*sin(q1).*8.191520442889917e-1-sin(q2-q3).*sin(q1).*sin(q4).*5.735764363510462e-1)-dq5.*sin(q5).*(cos(q2).*cos(q4).*sin(q1).*sin(q3)-cos(q3).*cos(q4).*sin(q1).*sin(q2))))-real(dq6.*cos(q6).*(cos(q5).*(cos(q2-q3).*cos(q1).*8.191520442889917e-1-sin(q2-q3).*cos(q1).*sin(q4).*5.735764363510462e-1).*5.735764363510462e-1+sin(q5).*(cos(q1).*cos(q2).*cos(q4).*sin(q3)-cos(q1).*cos(q3).*cos(q4).*sin(q2)).*5.735764363510462e-1+cos(q2-q3).*cos(q1).*4.698463103929542e-1+sin(q2-q3).*cos(q1).*sin(q4).*6.710100716628342e-1))+imag(dq6.*sin(q6).*(cos(q5).*(cos(q2).*cos(q4).*sin(q1).*sin(q3)-cos(q3).*cos(q4).*sin(q1).*sin(q2))-sin(q5).*(cos(q2-q3).*sin(q1).*8.191520442889917e-1-sin(q2-q3).*sin(q1).*sin(q4).*5.735764363510462e-1))))-1.0./(real(sin(q6).*(cos(q4).*sin(q1).*(-6.710100716628342e-1)+cos(q5).*(cos(q4).*sin(q1).*5.735764363510462e-1+sin(q2-q3).*cos(q1).*8.191520442889917e-1+cos(q2-q3).*cos(q1).*sin(q4).*5.735764363510462e-1).*5.735764363510462e-1+sin(q2-q3).*cos(q1).*4.698463103929542e-1+sin(q5).*(-sin(q1).*sin(q4)+cos(q1).*cos(q2).*cos(q3).*cos(q4)+cos(q1).*cos(q4).*sin(q2).*sin(q3)).*5.735764363510462e-1-cos(q2-q3).*cos(q1).*sin(q4).*6.710100716628342e-1))+real(cos(q6).*(sin(q5).*(cos(q4).*sin(q1).*5.735764363510462e-1+sin(q2-q3).*cos(q1).*8.191520442889917e-1+cos(q2-q3).*cos(q1).*sin(q4).*5.735764363510462e-1)-cos(q5).*(-sin(q1).*sin(q4)+cos(q1).*cos(q2).*cos(q3).*cos(q4)+cos(q1).*cos(q4).*sin(q2).*sin(q3))))-imag(sin(q6).*(cos(q1).*cos(q4).*6.710100716628342e-1+cos(q5).*(cos(q1).*cos(q4).*(-5.735764363510462e-1)+sin(q2-q3).*sin(q1).*8.191520442889917e-1+cos(q2-q3).*sin(q1).*sin(q4).*5.735764363510462e-1).*5.735764363510462e-1+sin(q2-q3).*sin(q1).*4.698463103929542e-1+sin(q5).*(cos(q1).*sin(q4)+cos(q2).*cos(q3).*cos(q4).*sin(q1)+cos(q4).*sin(q1).*sin(q2).*sin(q3)).*5.735764363510462e-1-cos(q2-q3).*sin(q1).*sin(q4).*6.710100716628342e-1))-imag(cos(q6).*(sin(q5).*(cos(q1).*cos(q4).*(-5.735764363510462e-1)+sin(q2-q3).*sin(q1).*8.191520442889917e-1+cos(q2-q3).*sin(q1).*sin(q4).*5.735764363510462e-1)-cos(q5).*(cos(q1).*sin(q4)+cos(q2).*cos(q3).*cos(q4).*sin(q1)+cos(q4).*sin(q1).*sin(q2).*sin(q3))))).^2.*(imag(cos(q6).*(cos(q5).*(cos(q1).*cos(q2).*cos(q4).*sin(q3)-cos(q1).*cos(q3).*cos(q4).*sin(q2))-sin(q5).*(cos(q2-q3).*cos(q1).*8.191520442889917e-1-sin(q2-q3).*cos(q1).*sin(q4).*5.735764363510462e-1)))-imag(sin(q6).*(cos(q5).*(cos(q2-q3).*cos(q1).*8.191520442889917e-1-sin(q2-q3).*cos(q1).*sin(q4).*5.735764363510462e-1).*5.735764363510462e-1+sin(q5).*(cos(q1).*cos(q2).*cos(q4).*sin(q3)-cos(q1).*cos(q3).*cos(q4).*sin(q2)).*5.735764363510462e-1+cos(q2-q3).*cos(q1).*4.698463103929542e-1+sin(q2-q3).*cos(q1).*sin(q4).*6.710100716628342e-1))+real(cos(q6).*(cos(q5).*(cos(q2).*cos(q4).*sin(q1).*sin(q3)-cos(q3).*cos(q4).*sin(q1).*sin(q2))-sin(q5).*(cos(q2-q3).*sin(q1).*8.191520442889917e-1-sin(q2-q3).*sin(q1).*sin(q4).*5.735764363510462e-1)))-real(sin(q6).*(cos(q5).*(cos(q2-q3).*sin(q1).*8.191520442889917e-1-sin(q2-q3).*sin(q1).*sin(q4).*5.735764363510462e-1).*5.735764363510462e-1+sin(q5).*(cos(q2).*cos(q4).*sin(q1).*sin(q3)-cos(q3).*cos(q4).*sin(q1).*sin(q2)).*5.735764363510462e-1+cos(q2-q3).*sin(q1).*4.698463103929542e-1+sin(q2-q3).*sin(q1).*sin(q4).*6.710100716628342e-1))).*(-real(cos(q6).*(-sin(q5).*(dq1.*cos(q1).*cos(q4).*(-5.735764363510462e-1)+dq4.*sin(q1).*sin(q4).*5.735764363510462e-1+dq1.*sin(q2-q3).*sin(q1).*8.191520442889917e-1-cos(q2-q3).*cos(q1).*(dq2-dq3).*8.191520442889917e-1-dq4.*cos(q2-q3).*cos(q1).*cos(q4).*5.735764363510462e-1+dq1.*cos(q2-q3).*sin(q1).*sin(q4).*5.735764363510462e-1+sin(q2-q3).*cos(q1).*sin(q4).*(dq2-dq3).*5.735764363510462e-1)+cos(q5).*(dq1.*cos(q1).*sin(q4)+dq4.*cos(q4).*sin(q1)+dq1.*cos(q2).*cos(q3).*cos(q4).*sin(q1)-dq2.*cos(q1).*cos(q2).*cos(q4).*sin(q3)+dq2.*cos(q1).*cos(q3).*cos(q4).*sin(q2)+dq3.*cos(q1).*cos(q2).*cos(q4).*sin(q3)-dq3.*cos(q1).*cos(q3).*cos(q4).*sin(q2)+dq4.*cos(q1).*cos(q2).*cos(q3).*sin(q4)+dq1.*cos(q4).*sin(q1).*sin(q2).*sin(q3)+dq4.*cos(q1).*sin(q2).*sin(q3).*sin(q4))+dq5.*cos(q5).*(cos(q4).*sin(q1).*5.735764363510462e-1+sin(q2-q3).*cos(q1).*8.191520442889917e-1+cos(q2-q3).*cos(q1).*sin(q4).*5.735764363510462e-1)+dq5.*sin(q5).*(-sin(q1).*sin(q4)+cos(q1).*cos(q2).*cos(q3).*cos(q4)+cos(q1).*cos(q4).*sin(q2).*sin(q3))))+real(sin(q6).*(sin(q5).*(dq1.*cos(q1).*sin(q4)+dq4.*cos(q4).*sin(q1)+dq1.*cos(q2).*cos(q3).*cos(q4).*sin(q1)-dq2.*cos(q1).*cos(q2).*cos(q4).*sin(q3)+dq2.*cos(q1).*cos(q3).*cos(q4).*sin(q2)+dq3.*cos(q1).*cos(q2).*cos(q4).*sin(q3)-dq3.*cos(q1).*cos(q3).*cos(q4).*sin(q2)+dq4.*cos(q1).*cos(q2).*cos(q3).*sin(q4)+dq1.*cos(q4).*sin(q1).*sin(q2).*sin(q3)+dq4.*cos(q1).*sin(q2).*sin(q3).*sin(q4)).*5.735764363510462e-1+cos(q5).*(dq1.*cos(q1).*cos(q4).*(-5.735764363510462e-1)+dq4.*sin(q1).*sin(q4).*5.735764363510462e-1+dq1.*sin(q2-q3).*sin(q1).*8.191520442889917e-1-cos(q2-q3).*cos(q1).*(dq2-dq3).*8.191520442889917e-1-dq4.*cos(q2-q3).*cos(q1).*cos(q4).*5.735764363510462e-1+dq1.*cos(q2-q3).*sin(q1).*sin(q4).*5.735764363510462e-1+sin(q2-q3).*cos(q1).*sin(q4).*(dq2-dq3).*5.735764363510462e-1).*5.735764363510462e-1+dq1.*cos(q1).*cos(q4).*6.710100716628342e-1-dq4.*sin(q1).*sin(q4).*6.710100716628342e-1+dq5.*sin(q5).*(cos(q4).*sin(q1).*5.735764363510462e-1+sin(q2-q3).*cos(q1).*8.191520442889917e-1+cos(q2-q3).*cos(q1).*sin(q4).*5.735764363510462e-1).*5.735764363510462e-1-dq5.*cos(q5).*(-sin(q1).*sin(q4)+cos(q1).*cos(q2).*cos(q3).*cos(q4)+cos(q1).*cos(q4).*sin(q2).*sin(q3)).*5.735764363510462e-1+dq1.*sin(q2-q3).*sin(q1).*4.698463103929542e-1-cos(q2-q3).*cos(q1).*(dq2-dq3).*4.698463103929542e-1+dq4.*cos(q2-q3).*cos(q1).*cos(q4).*6.710100716628342e-1-dq1.*cos(q2-q3).*sin(q1).*sin(q4).*6.710100716628342e-1-sin(q2-q3).*cos(q1).*sin(q4).*(dq2-dq3).*6.710100716628342e-1))+imag(cos(q6).*(sin(q5).*(dq1.*cos(q4).*sin(q1).*5.735764363510462e-1+dq4.*cos(q1).*sin(q4).*5.735764363510462e-1+dq1.*sin(q2-q3).*cos(q1).*8.191520442889917e-1+cos(q2-q3).*sin(q1).*(dq2-dq3).*8.191520442889917e-1+dq1.*cos(q2-q3).*cos(q1).*sin(q4).*5.735764363510462e-1+dq4.*cos(q2-q3).*cos(q4).*sin(q1).*5.735764363510462e-1-sin(q2-q3).*sin(q1).*sin(q4).*(dq2-dq3).*5.735764363510462e-1)-cos(q5).*(dq4.*cos(q1).*cos(q4)-dq1.*sin(q1).*sin(q4)+dq1.*cos(q1).*cos(q2).*cos(q3).*cos(q4)+dq1.*cos(q1).*cos(q4).*sin(q2).*sin(q3)+dq2.*cos(q2).*cos(q4).*sin(q1).*sin(q3)-dq2.*cos(q3).*cos(q4).*sin(q1).*sin(q2)-dq3.*cos(q2).*cos(q4).*sin(q1).*sin(q3)+dq3.*cos(q3).*cos(q4).*sin(q1).*sin(q2)-dq4.*cos(q2).*cos(q3).*sin(q1).*sin(q4)-dq4.*sin(q1).*sin(q2).*sin(q3).*sin(q4))+dq5.*cos(q5).*(cos(q1).*cos(q4).*(-5.735764363510462e-1)+sin(q2-q3).*sin(q1).*8.191520442889917e-1+cos(q2-q3).*sin(q1).*sin(q4).*5.735764363510462e-1)+dq5.*sin(q5).*(cos(q1).*sin(q4)+cos(q2).*cos(q3).*cos(q4).*sin(q1)+cos(q4).*sin(q1).*sin(q2).*sin(q3))))-real(dq6.*cos(q6).*(cos(q4).*sin(q1).*(-6.710100716628342e-1)+cos(q5).*(cos(q4).*sin(q1).*5.735764363510462e-1+sin(q2-q3).*cos(q1).*8.191520442889917e-1+cos(q2-q3).*cos(q1).*sin(q4).*5.735764363510462e-1).*5.735764363510462e-1+sin(q2-q3).*cos(q1).*4.698463103929542e-1+sin(q5).*(-sin(q1).*sin(q4)+cos(q1).*cos(q2).*cos(q3).*cos(q4)+cos(q1).*cos(q4).*sin(q2).*sin(q3)).*5.735764363510462e-1-cos(q2-q3).*cos(q1).*sin(q4).*6.710100716628342e-1))+imag(dq6.*cos(q6).*(cos(q1).*cos(q4).*6.710100716628342e-1+cos(q5).*(cos(q1).*cos(q4).*(-5.735764363510462e-1)+sin(q2-q3).*sin(q1).*8.191520442889917e-1+cos(q2-q3).*sin(q1).*sin(q4).*5.735764363510462e-1).*5.735764363510462e-1+sin(q2-q3).*sin(q1).*4.698463103929542e-1+sin(q5).*(cos(q1).*sin(q4)+cos(q2).*cos(q3).*cos(q4).*sin(q1)+cos(q4).*sin(q1).*sin(q2).*sin(q3)).*5.735764363510462e-1-cos(q2-q3).*sin(q1).*sin(q4).*6.710100716628342e-1))+real(dq6.*sin(q6).*(sin(q5).*(cos(q4).*sin(q1).*5.735764363510462e-1+sin(q2-q3).*cos(q1).*8.191520442889917e-1+cos(q2-q3).*cos(q1).*sin(q4).*5.735764363510462e-1)-cos(q5).*(-sin(q1).*sin(q4)+cos(q1).*cos(q2).*cos(q3).*cos(q4)+cos(q1).*cos(q4).*sin(q2).*sin(q3))))-imag(dq6.*sin(q6).*(sin(q5).*(cos(q1).*cos(q4).*(-5.735764363510462e-1)+sin(q2-q3).*sin(q1).*8.191520442889917e-1+cos(q2-q3).*sin(q1).*sin(q4).*5.735764363510462e-1)-cos(q5).*(cos(q1).*sin(q4)+cos(q2).*cos(q3).*cos(q4).*sin(q1)+cos(q4).*sin(q1).*sin(q2).*sin(q3))))+imag(sin(q6).*(cos(q5).*(dq1.*cos(q4).*sin(q1).*5.735764363510462e-1+dq4.*cos(q1).*sin(q4).*5.735764363510462e-1+dq1.*sin(q2-q3).*cos(q1).*8.191520442889917e-1+cos(q2-q3).*sin(q1).*(dq2-dq3).*8.191520442889917e-1+dq1.*cos(q2-q3).*cos(q1).*sin(q4).*5.735764363510462e-1+dq4.*cos(q2-q3).*cos(q4).*sin(q1).*5.735764363510462e-1-sin(q2-q3).*sin(q1).*sin(q4).*(dq2-dq3).*5.735764363510462e-1).*5.735764363510462e-1+sin(q5).*(dq4.*cos(q1).*cos(q4)-dq1.*sin(q1).*sin(q4)+dq1.*cos(q1).*cos(q2).*cos(q3).*cos(q4)+dq1.*cos(q1).*cos(q4).*sin(q2).*sin(q3)+dq2.*cos(q2).*cos(q4).*sin(q1).*sin(q3)-dq2.*cos(q3).*cos(q4).*sin(q1).*sin(q2)-dq3.*cos(q2).*cos(q4).*sin(q1).*sin(q3)+dq3.*cos(q3).*cos(q4).*sin(q1).*sin(q2)-dq4.*cos(q2).*cos(q3).*sin(q1).*sin(q4)-dq4.*sin(q1).*sin(q2).*sin(q3).*sin(q4)).*5.735764363510462e-1-dq1.*cos(q4).*sin(q1).*6.710100716628342e-1-dq4.*cos(q1).*sin(q4).*6.710100716628342e-1+dq1.*sin(q2-q3).*cos(q1).*4.698463103929542e-1-dq5.*sin(q5).*(cos(q1).*cos(q4).*(-5.735764363510462e-1)+sin(q2-q3).*sin(q1).*8.191520442889917e-1+cos(q2-q3).*sin(q1).*sin(q4).*5.735764363510462e-1).*5.735764363510462e-1+dq5.*cos(q5).*(cos(q1).*sin(q4)+cos(q2).*cos(q3).*cos(q4).*sin(q1)+cos(q4).*sin(q1).*sin(q2).*sin(q3)).*5.735764363510462e-1+cos(q2-q3).*sin(q1).*(dq2-dq3).*4.698463103929542e-1-dq1.*cos(q2-q3).*cos(q1).*sin(q4).*6.710100716628342e-1-dq4.*cos(q2-q3).*cos(q4).*sin(q1).*6.710100716628342e-1+sin(q2-q3).*sin(q1).*sin(q4).*(dq2-dq3).*6.710100716628342e-1)))+1.0./(real(sin(q6).*(cos(q4).*sin(q1).*(-6.710100716628342e-1)+cos(q5).*(cos(q4).*sin(q1).*5.735764363510462e-1+sin(q2-q3).*cos(q1).*8.191520442889917e-1+cos(q2-q3).*cos(q1).*sin(q4).*5.735764363510462e-1).*5.735764363510462e-1+sin(q2-q3).*cos(q1).*4.698463103929542e-1+sin(q5).*(-sin(q1).*sin(q4)+cos(q1).*cos(q2).*cos(q3).*cos(q4)+cos(q1).*cos(q4).*sin(q2).*sin(q3)).*5.735764363510462e-1-cos(q2-q3).*cos(q1).*sin(q4).*6.710100716628342e-1))+real(cos(q6).*(sin(q5).*(cos(q4).*sin(q1).*5.735764363510462e-1+sin(q2-q3).*cos(q1).*8.191520442889917e-1+cos(q2-q3).*cos(q1).*sin(q4).*5.735764363510462e-1)-cos(q5).*(-sin(q1).*sin(q4)+cos(q1).*cos(q2).*cos(q3).*cos(q4)+cos(q1).*cos(q4).*sin(q2).*sin(q3))))-imag(sin(q6).*(cos(q1).*cos(q4).*6.710100716628342e-1+cos(q5).*(cos(q1).*cos(q4).*(-5.735764363510462e-1)+sin(q2-q3).*sin(q1).*8.191520442889917e-1+cos(q2-q3).*sin(q1).*sin(q4).*5.735764363510462e-1).*5.735764363510462e-1+sin(q2-q3).*sin(q1).*4.698463103929542e-1+sin(q5).*(cos(q1).*sin(q4)+cos(q2).*cos(q3).*cos(q4).*sin(q1)+cos(q4).*sin(q1).*sin(q2).*sin(q3)).*5.735764363510462e-1-cos(q2-q3).*sin(q1).*sin(q4).*6.710100716628342e-1))-imag(cos(q6).*(sin(q5).*(cos(q1).*cos(q4).*(-5.735764363510462e-1)+sin(q2-q3).*sin(q1).*8.191520442889917e-1+cos(q2-q3).*sin(q1).*sin(q4).*5.735764363510462e-1)-cos(q5).*(cos(q1).*sin(q4)+cos(q2).*cos(q3).*cos(q4).*sin(q1)+cos(q4).*sin(q1).*sin(q2).*sin(q3))))).^2.*(real(cos(q6).*(cos(q5).*(cos(q1).*cos(q2).*cos(q4).*sin(q3)-cos(q1).*cos(q3).*cos(q4).*sin(q2))-sin(q5).*(cos(q2-q3).*cos(q1).*8.191520442889917e-1-sin(q2-q3).*cos(q1).*sin(q4).*5.735764363510462e-1)))-imag(cos(q6).*(cos(q5).*(cos(q2).*cos(q4).*sin(q1).*sin(q3)-cos(q3).*cos(q4).*sin(q1).*sin(q2))-sin(q5).*(cos(q2-q3).*sin(q1).*8.191520442889917e-1-sin(q2-q3).*sin(q1).*sin(q4).*5.735764363510462e-1)))-real(sin(q6).*(cos(q5).*(cos(q2-q3).*cos(q1).*8.191520442889917e-1-sin(q2-q3).*cos(q1).*sin(q4).*5.735764363510462e-1).*5.735764363510462e-1+sin(q5).*(cos(q1).*cos(q2).*cos(q4).*sin(q3)-cos(q1).*cos(q3).*cos(q4).*sin(q2)).*5.735764363510462e-1+cos(q2-q3).*cos(q1).*4.698463103929542e-1+sin(q2-q3).*cos(q1).*sin(q4).*6.710100716628342e-1))+imag(sin(q6).*(cos(q5).*(cos(q2-q3).*sin(q1).*8.191520442889917e-1-sin(q2-q3).*sin(q1).*sin(q4).*5.735764363510462e-1).*5.735764363510462e-1+sin(q5).*(cos(q2).*cos(q4).*sin(q1).*sin(q3)-cos(q3).*cos(q4).*sin(q1).*sin(q2)).*5.735764363510462e-1+cos(q2-q3).*sin(q1).*4.698463103929542e-1+sin(q2-q3).*sin(q1).*sin(q4).*6.710100716628342e-1))).*(real(sin(q6).*(cos(q5).*(dq1.*cos(q4).*sin(q1).*5.735764363510462e-1+dq4.*cos(q1).*sin(q4).*5.735764363510462e-1+dq1.*sin(q2-q3).*cos(q1).*8.191520442889917e-1+cos(q2-q3).*sin(q1).*(dq2-dq3).*8.191520442889917e-1+dq1.*cos(q2-q3).*cos(q1).*sin(q4).*5.735764363510462e-1+dq4.*cos(q2-q3).*cos(q4).*sin(q1).*5.735764363510462e-1-sin(q2-q3).*sin(q1).*sin(q4).*(dq2-dq3).*5.735764363510462e-1).*5.735764363510462e-1+sin(q5).*(dq4.*cos(q1).*cos(q4)-dq1.*sin(q1).*sin(q4)+dq1.*cos(q1).*cos(q2).*cos(q3).*cos(q4)+dq1.*cos(q1).*cos(q4).*sin(q2).*sin(q3)+dq2.*cos(q2).*cos(q4).*sin(q1).*sin(q3)-dq2.*cos(q3).*cos(q4).*sin(q1).*sin(q2)-dq3.*cos(q2).*cos(q4).*sin(q1).*sin(q3)+dq3.*cos(q3).*cos(q4).*sin(q1).*sin(q2)-dq4.*cos(q2).*cos(q3).*sin(q1).*sin(q4)-dq4.*sin(q1).*sin(q2).*sin(q3).*sin(q4)).*5.735764363510462e-1-dq1.*cos(q4).*sin(q1).*6.710100716628342e-1-dq4.*cos(q1).*sin(q4).*6.710100716628342e-1+dq1.*sin(q2-q3).*cos(q1).*4.698463103929542e-1-dq5.*sin(q5).*(cos(q1).*cos(q4).*(-5.735764363510462e-1)+sin(q2-q3).*sin(q1).*8.191520442889917e-1+cos(q2-q3).*sin(q1).*sin(q4).*5.735764363510462e-1).*5.735764363510462e-1+dq5.*cos(q5).*(cos(q1).*sin(q4)+cos(q2).*cos(q3).*cos(q4).*sin(q1)+cos(q4).*sin(q1).*sin(q2).*sin(q3)).*5.735764363510462e-1+cos(q2-q3).*sin(q1).*(dq2-dq3).*4.698463103929542e-1-dq1.*cos(q2-q3).*cos(q1).*sin(q4).*6.710100716628342e-1-dq4.*cos(q2-q3).*cos(q4).*sin(q1).*6.710100716628342e-1+sin(q2-q3).*sin(q1).*sin(q4).*(dq2-dq3).*6.710100716628342e-1))+imag(cos(q6).*(-sin(q5).*(dq1.*cos(q1).*cos(q4).*(-5.735764363510462e-1)+dq4.*sin(q1).*sin(q4).*5.735764363510462e-1+dq1.*sin(q2-q3).*sin(q1).*8.191520442889917e-1-cos(q2-q3).*cos(q1).*(dq2-dq3).*8.191520442889917e-1-dq4.*cos(q2-q3).*cos(q1).*cos(q4).*5.735764363510462e-1+dq1.*cos(q2-q3).*sin(q1).*sin(q4).*5.735764363510462e-1+sin(q2-q3).*cos(q1).*sin(q4).*(dq2-dq3).*5.735764363510462e-1)+cos(q5).*(dq1.*cos(q1).*sin(q4)+dq4.*cos(q4).*sin(q1)+dq1.*cos(q2).*cos(q3).*cos(q4).*sin(q1)-dq2.*cos(q1).*cos(q2).*cos(q4).*sin(q3)+dq2.*cos(q1).*cos(q3).*cos(q4).*sin(q2)+dq3.*cos(q1).*cos(q2).*cos(q4).*sin(q3)-dq3.*cos(q1).*cos(q3).*cos(q4).*sin(q2)+dq4.*cos(q1).*cos(q2).*cos(q3).*sin(q4)+dq1.*cos(q4).*sin(q1).*sin(q2).*sin(q3)+dq4.*cos(q1).*sin(q2).*sin(q3).*sin(q4))+dq5.*cos(q5).*(cos(q4).*sin(q1).*5.735764363510462e-1+sin(q2-q3).*cos(q1).*8.191520442889917e-1+cos(q2-q3).*cos(q1).*sin(q4).*5.735764363510462e-1)+dq5.*sin(q5).*(-sin(q1).*sin(q4)+cos(q1).*cos(q2).*cos(q3).*cos(q4)+cos(q1).*cos(q4).*sin(q2).*sin(q3))))-imag(sin(q6).*(sin(q5).*(dq1.*cos(q1).*sin(q4)+dq4.*cos(q4).*sin(q1)+dq1.*cos(q2).*cos(q3).*cos(q4).*sin(q1)-dq2.*cos(q1).*cos(q2).*cos(q4).*sin(q3)+dq2.*cos(q1).*cos(q3).*cos(q4).*sin(q2)+dq3.*cos(q1).*cos(q2).*cos(q4).*sin(q3)-dq3.*cos(q1).*cos(q3).*cos(q4).*sin(q2)+dq4.*cos(q1).*cos(q2).*cos(q3).*sin(q4)+dq1.*cos(q4).*sin(q1).*sin(q2).*sin(q3)+dq4.*cos(q1).*sin(q2).*sin(q3).*sin(q4)).*5.735764363510462e-1+cos(q5).*(dq1.*cos(q1).*cos(q4).*(-5.735764363510462e-1)+dq4.*sin(q1).*sin(q4).*5.735764363510462e-1+dq1.*sin(q2-q3).*sin(q1).*8.191520442889917e-1-cos(q2-q3).*cos(q1).*(dq2-dq3).*8.191520442889917e-1-dq4.*cos(q2-q3).*cos(q1).*cos(q4).*5.735764363510462e-1+dq1.*cos(q2-q3).*sin(q1).*sin(q4).*5.735764363510462e-1+sin(q2-q3).*cos(q1).*sin(q4).*(dq2-dq3).*5.735764363510462e-1).*5.735764363510462e-1+dq1.*cos(q1).*cos(q4).*6.710100716628342e-1-dq4.*sin(q1).*sin(q4).*6.710100716628342e-1+dq5.*sin(q5).*(cos(q4).*sin(q1).*5.735764363510462e-1+sin(q2-q3).*cos(q1).*8.191520442889917e-1+cos(q2-q3).*cos(q1).*sin(q4).*5.735764363510462e-1).*5.735764363510462e-1-dq5.*cos(q5).*(-sin(q1).*sin(q4)+cos(q1).*cos(q2).*cos(q3).*cos(q4)+cos(q1).*cos(q4).*sin(q2).*sin(q3)).*5.735764363510462e-1+dq1.*sin(q2-q3).*sin(q1).*4.698463103929542e-1-cos(q2-q3).*cos(q1).*(dq2-dq3).*4.698463103929542e-1+dq4.*cos(q2-q3).*cos(q1).*cos(q4).*6.710100716628342e-1-dq1.*cos(q2-q3).*sin(q1).*sin(q4).*6.710100716628342e-1-sin(q2-q3).*cos(q1).*sin(q4).*(dq2-dq3).*6.710100716628342e-1))+imag(dq6.*cos(q6).*(cos(q4).*sin(q1).*(-6.710100716628342e-1)+cos(q5).*(cos(q4).*sin(q1).*5.735764363510462e-1+sin(q2-q3).*cos(q1).*8.191520442889917e-1+cos(q2-q3).*cos(q1).*sin(q4).*5.735764363510462e-1).*5.735764363510462e-1+sin(q2-q3).*cos(q1).*4.698463103929542e-1+sin(q5).*(-sin(q1).*sin(q4)+cos(q1).*cos(q2).*cos(q3).*cos(q4)+cos(q1).*cos(q4).*sin(q2).*sin(q3)).*5.735764363510462e-1-cos(q2-q3).*cos(q1).*sin(q4).*6.710100716628342e-1))+real(cos(q6).*(sin(q5).*(dq1.*cos(q4).*sin(q1).*5.735764363510462e-1+dq4.*cos(q1).*sin(q4).*5.735764363510462e-1+dq1.*sin(q2-q3).*cos(q1).*8.191520442889917e-1+cos(q2-q3).*sin(q1).*(dq2-dq3).*8.191520442889917e-1+dq1.*cos(q2-q3).*cos(q1).*sin(q4).*5.735764363510462e-1+dq4.*cos(q2-q3).*cos(q4).*sin(q1).*5.735764363510462e-1-sin(q2-q3).*sin(q1).*sin(q4).*(dq2-dq3).*5.735764363510462e-1)-cos(q5).*(dq4.*cos(q1).*cos(q4)-dq1.*sin(q1).*sin(q4)+dq1.*cos(q1).*cos(q2).*cos(q3).*cos(q4)+dq1.*cos(q1).*cos(q4).*sin(q2).*sin(q3)+dq2.*cos(q2).*cos(q4).*sin(q1).*sin(q3)-dq2.*cos(q3).*cos(q4).*sin(q1).*sin(q2)-dq3.*cos(q2).*cos(q4).*sin(q1).*sin(q3)+dq3.*cos(q3).*cos(q4).*sin(q1).*sin(q2)-dq4.*cos(q2).*cos(q3).*sin(q1).*sin(q4)-dq4.*sin(q1).*sin(q2).*sin(q3).*sin(q4))+dq5.*cos(q5).*(cos(q1).*cos(q4).*(-5.735764363510462e-1)+sin(q2-q3).*sin(q1).*8.191520442889917e-1+cos(q2-q3).*sin(q1).*sin(q4).*5.735764363510462e-1)+dq5.*sin(q5).*(cos(q1).*sin(q4)+cos(q2).*cos(q3).*cos(q4).*sin(q1)+cos(q4).*sin(q1).*sin(q2).*sin(q3))))+real(dq6.*cos(q6).*(cos(q1).*cos(q4).*6.710100716628342e-1+cos(q5).*(cos(q1).*cos(q4).*(-5.735764363510462e-1)+sin(q2-q3).*sin(q1).*8.191520442889917e-1+cos(q2-q3).*sin(q1).*sin(q4).*5.735764363510462e-1).*5.735764363510462e-1+sin(q2-q3).*sin(q1).*4.698463103929542e-1+sin(q5).*(cos(q1).*sin(q4)+cos(q2).*cos(q3).*cos(q4).*sin(q1)+cos(q4).*sin(q1).*sin(q2).*sin(q3)).*5.735764363510462e-1-cos(q2-q3).*sin(q1).*sin(q4).*6.710100716628342e-1))-imag(dq6.*sin(q6).*(sin(q5).*(cos(q4).*sin(q1).*5.735764363510462e-1+sin(q2-q3).*cos(q1).*8.191520442889917e-1+cos(q2-q3).*cos(q1).*sin(q4).*5.735764363510462e-1)-cos(q5).*(-sin(q1).*sin(q4)+cos(q1).*cos(q2).*cos(q3).*cos(q4)+cos(q1).*cos(q4).*sin(q2).*sin(q3))))-real(dq6.*sin(q6).*(sin(q5).*(cos(q1).*cos(q4).*(-5.735764363510462e-1)+sin(q2-q3).*sin(q1).*8.191520442889917e-1+cos(q2-q3).*sin(q1).*sin(q4).*5.735764363510462e-1)-cos(q5).*(cos(q1).*sin(q4)+cos(q2).*cos(q3).*cos(q4).*sin(q1)+cos(q4).*sin(q1).*sin(q2).*sin(q3)))))+1.0./(real(sin(q6).*(cos(q4).*sin(q1).*(-6.710100716628342e-1)+cos(q5).*(cos(q4).*sin(q1).*5.735764363510462e-1+sin(q2-q3).*cos(q1).*8.191520442889917e-1+cos(q2-q3).*cos(q1).*sin(q4).*5.735764363510462e-1).*5.735764363510462e-1+sin(q2-q3).*cos(q1).*4.698463103929542e-1+sin(q5).*(-sin(q1).*sin(q4)+cos(q1).*cos(q2).*cos(q3).*cos(q4)+cos(q1).*cos(q4).*sin(q2).*sin(q3)).*5.735764363510462e-1-cos(q2-q3).*cos(q1).*sin(q4).*6.710100716628342e-1))+real(cos(q6).*(sin(q5).*(cos(q4).*sin(q1).*5.735764363510462e-1+sin(q2-q3).*cos(q1).*8.191520442889917e-1+cos(q2-q3).*cos(q1).*sin(q4).*5.735764363510462e-1)-cos(q5).*(-sin(q1).*sin(q4)+cos(q1).*cos(q2).*cos(q3).*cos(q4)+cos(q1).*cos(q4).*sin(q2).*sin(q3))))-imag(sin(q6).*(cos(q1).*cos(q4).*6.710100716628342e-1+cos(q5).*(cos(q1).*cos(q4).*(-5.735764363510462e-1)+sin(q2-q3).*sin(q1).*8.191520442889917e-1+cos(q2-q3).*sin(q1).*sin(q4).*5.735764363510462e-1).*5.735764363510462e-1+sin(q2-q3).*sin(q1).*4.698463103929542e-1+sin(q5).*(cos(q1).*sin(q4)+cos(q2).*cos(q3).*cos(q4).*sin(q1)+cos(q4).*sin(q1).*sin(q2).*sin(q3)).*5.735764363510462e-1-cos(q2-q3).*sin(q1).*sin(q4).*6.710100716628342e-1))-imag(cos(q6).*(sin(q5).*(cos(q1).*cos(q4).*(-5.735764363510462e-1)+sin(q2-q3).*sin(q1).*8.191520442889917e-1+cos(q2-q3).*sin(q1).*sin(q4).*5.735764363510462e-1)-cos(q5).*(cos(q1).*sin(q4)+cos(q2).*cos(q3).*cos(q4).*sin(q1)+cos(q4).*sin(q1).*sin(q2).*sin(q3))))).^3.*(real(cos(q6).*(cos(q5).*(cos(q1).*cos(q2).*cos(q4).*sin(q3)-cos(q1).*cos(q3).*cos(q4).*sin(q2))-sin(q5).*(cos(q2-q3).*cos(q1).*8.191520442889917e-1-sin(q2-q3).*cos(q1).*sin(q4).*5.735764363510462e-1)))-imag(cos(q6).*(cos(q5).*(cos(q2).*cos(q4).*sin(q1).*sin(q3)-cos(q3).*cos(q4).*sin(q1).*sin(q2))-sin(q5).*(cos(q2-q3).*sin(q1).*8.191520442889917e-1-sin(q2-q3).*sin(q1).*sin(q4).*5.735764363510462e-1)))-real(sin(q6).*(cos(q5).*(cos(q2-q3).*cos(q1).*8.191520442889917e-1-sin(q2-q3).*cos(q1).*sin(q4).*5.735764363510462e-1).*5.735764363510462e-1+sin(q5).*(cos(q1).*cos(q2).*cos(q4).*sin(q3)-cos(q1).*cos(q3).*cos(q4).*sin(q2)).*5.735764363510462e-1+cos(q2-q3).*cos(q1).*4.698463103929542e-1+sin(q2-q3).*cos(q1).*sin(q4).*6.710100716628342e-1))+imag(sin(q6).*(cos(q5).*(cos(q2-q3).*sin(q1).*8.191520442889917e-1-sin(q2-q3).*sin(q1).*sin(q4).*5.735764363510462e-1).*5.735764363510462e-1+sin(q5).*(cos(q2).*cos(q4).*sin(q1).*sin(q3)-cos(q3).*cos(q4).*sin(q1).*sin(q2)).*5.735764363510462e-1+cos(q2-q3).*sin(q1).*4.698463103929542e-1+sin(q2-q3).*sin(q1).*sin(q4).*6.710100716628342e-1))).*(imag(sin(q6).*(cos(q4).*sin(q1).*(-6.710100716628342e-1)+cos(q5).*(cos(q4).*sin(q1).*5.735764363510462e-1+sin(q2-q3).*cos(q1).*8.191520442889917e-1+cos(q2-q3).*cos(q1).*sin(q4).*5.735764363510462e-1).*5.735764363510462e-1+sin(q2-q3).*cos(q1).*4.698463103929542e-1+sin(q5).*(-sin(q1).*sin(q4)+cos(q1).*cos(q2).*cos(q3).*cos(q4)+cos(q1).*cos(q4).*sin(q2).*sin(q3)).*5.735764363510462e-1-cos(q2-q3).*cos(q1).*sin(q4).*6.710100716628342e-1))+imag(cos(q6).*(sin(q5).*(cos(q4).*sin(q1).*5.735764363510462e-1+sin(q2-q3).*cos(q1).*8.191520442889917e-1+cos(q2-q3).*cos(q1).*sin(q4).*5.735764363510462e-1)-cos(q5).*(-sin(q1).*sin(q4)+cos(q1).*cos(q2).*cos(q3).*cos(q4)+cos(q1).*cos(q4).*sin(q2).*sin(q3))))+real(sin(q6).*(cos(q1).*cos(q4).*6.710100716628342e-1+cos(q5).*(cos(q1).*cos(q4).*(-5.735764363510462e-1)+sin(q2-q3).*sin(q1).*8.191520442889917e-1+cos(q2-q3).*sin(q1).*sin(q4).*5.735764363510462e-1).*5.735764363510462e-1+sin(q2-q3).*sin(q1).*4.698463103929542e-1+sin(q5).*(cos(q1).*sin(q4)+cos(q2).*cos(q3).*cos(q4).*sin(q1)+cos(q4).*sin(q1).*sin(q2).*sin(q3)).*5.735764363510462e-1-cos(q2-q3).*sin(q1).*sin(q4).*6.710100716628342e-1))+real(cos(q6).*(sin(q5).*(cos(q1).*cos(q4).*(-5.735764363510462e-1)+sin(q2-q3).*sin(q1).*8.191520442889917e-1+cos(q2-q3).*sin(q1).*sin(q4).*5.735764363510462e-1)-cos(q5).*(cos(q1).*sin(q4)+cos(q2).*cos(q3).*cos(q4).*sin(q1)+cos(q4).*sin(q1).*sin(q2).*sin(q3))))).*(-real(cos(q6).*(-sin(q5).*(dq1.*cos(q1).*cos(q4).*(-5.735764363510462e-1)+dq4.*sin(q1).*sin(q4).*5.735764363510462e-1+dq1.*sin(q2-q3).*sin(q1).*8.191520442889917e-1-cos(q2-q3).*cos(q1).*(dq2-dq3).*8.191520442889917e-1-dq4.*cos(q2-q3).*cos(q1).*cos(q4).*5.735764363510462e-1+dq1.*cos(q2-q3).*sin(q1).*sin(q4).*5.735764363510462e-1+sin(q2-q3).*cos(q1).*sin(q4).*(dq2-dq3).*5.735764363510462e-1)+cos(q5).*(dq1.*cos(q1).*sin(q4)+dq4.*cos(q4).*sin(q1)+dq1.*cos(q2).*cos(q3).*cos(q4).*sin(q1)-dq2.*cos(q1).*cos(q2).*cos(q4).*sin(q3)+dq2.*cos(q1).*cos(q3).*cos(q4).*sin(q2)+dq3.*cos(q1).*cos(q2).*cos(q4).*sin(q3)-dq3.*cos(q1).*cos(q3).*cos(q4).*sin(q2)+dq4.*cos(q1).*cos(q2).*cos(q3).*sin(q4)+dq1.*cos(q4).*sin(q1).*sin(q2).*sin(q3)+dq4.*cos(q1).*sin(q2).*sin(q3).*sin(q4))+dq5.*cos(q5).*(cos(q4).*sin(q1).*5.735764363510462e-1+sin(q2-q3).*cos(q1).*8.191520442889917e-1+cos(q2-q3).*cos(q1).*sin(q4).*5.735764363510462e-1)+dq5.*sin(q5).*(-sin(q1).*sin(q4)+cos(q1).*cos(q2).*cos(q3).*cos(q4)+cos(q1).*cos(q4).*sin(q2).*sin(q3))))+real(sin(q6).*(sin(q5).*(dq1.*cos(q1).*sin(q4)+dq4.*cos(q4).*sin(q1)+dq1.*cos(q2).*cos(q3).*cos(q4).*sin(q1)-dq2.*cos(q1).*cos(q2).*cos(q4).*sin(q3)+dq2.*cos(q1).*cos(q3).*cos(q4).*sin(q2)+dq3.*cos(q1).*cos(q2).*cos(q4).*sin(q3)-dq3.*cos(q1).*cos(q3).*cos(q4).*sin(q2)+dq4.*cos(q1).*cos(q2).*cos(q3).*sin(q4)+dq1.*cos(q4).*sin(q1).*sin(q2).*sin(q3)+dq4.*cos(q1).*sin(q2).*sin(q3).*sin(q4)).*5.735764363510462e-1+cos(q5).*(dq1.*cos(q1).*cos(q4).*(-5.735764363510462e-1)+dq4.*sin(q1).*sin(q4).*5.735764363510462e-1+dq1.*sin(q2-q3).*sin(q1).*8.191520442889917e-1-cos(q2-q3).*cos(q1).*(dq2-dq3).*8.191520442889917e-1-dq4.*cos(q2-q3).*cos(q1).*cos(q4).*5.735764363510462e-1+dq1.*cos(q2-q3).*sin(q1).*sin(q4).*5.735764363510462e-1+sin(q2-q3).*cos(q1).*sin(q4).*(dq2-dq3).*5.735764363510462e-1).*5.735764363510462e-1+dq1.*cos(q1).*cos(q4).*6.710100716628342e-1-dq4.*sin(q1).*sin(q4).*6.710100716628342e-1+dq5.*sin(q5).*(cos(q4).*sin(q1).*5.735764363510462e-1+sin(q2-q3).*cos(q1).*8.191520442889917e-1+cos(q2-q3).*cos(q1).*sin(q4).*5.735764363510462e-1).*5.735764363510462e-1-dq5.*cos(q5).*(-sin(q1).*sin(q4)+cos(q1).*cos(q2).*cos(q3).*cos(q4)+cos(q1).*cos(q4).*sin(q2).*sin(q3)).*5.735764363510462e-1+dq1.*sin(q2-q3).*sin(q1).*4.698463103929542e-1-cos(q2-q3).*cos(q1).*(dq2-dq3).*4.698463103929542e-1+dq4.*cos(q2-q3).*cos(q1).*cos(q4).*6.710100716628342e-1-dq1.*cos(q2-q3).*sin(q1).*sin(q4).*6.710100716628342e-1-sin(q2-q3).*cos(q1).*sin(q4).*(dq2-dq3).*6.710100716628342e-1))+imag(cos(q6).*(sin(q5).*(dq1.*cos(q4).*sin(q1).*5.735764363510462e-1+dq4.*cos(q1).*sin(q4).*5.735764363510462e-1+dq1.*sin(q2-q3).*cos(q1).*8.191520442889917e-1+cos(q2-q3).*sin(q1).*(dq2-dq3).*8.191520442889917e-1+dq1.*cos(q2-q3).*cos(q1).*sin(q4).*5.735764363510462e-1+dq4.*cos(q2-q3).*cos(q4).*sin(q1).*5.735764363510462e-1-sin(q2-q3).*sin(q1).*sin(q4).*(dq2-dq3).*5.735764363510462e-1)-cos(q5).*(dq4.*cos(q1).*cos(q4)-dq1.*sin(q1).*sin(q4)+dq1.*cos(q1).*cos(q2).*cos(q3).*cos(q4)+dq1.*cos(q1).*cos(q4).*sin(q2).*sin(q3)+dq2.*cos(q2).*cos(q4).*sin(q1).*sin(q3)-dq2.*cos(q3).*cos(q4).*sin(q1).*sin(q2)-dq3.*cos(q2).*cos(q4).*sin(q1).*sin(q3)+dq3.*cos(q3).*cos(q4).*sin(q1).*sin(q2)-dq4.*cos(q2).*cos(q3).*sin(q1).*sin(q4)-dq4.*sin(q1).*sin(q2).*sin(q3).*sin(q4))+dq5.*cos(q5).*(cos(q1).*cos(q4).*(-5.735764363510462e-1)+sin(q2-q3).*sin(q1).*8.191520442889917e-1+cos(q2-q3).*sin(q1).*sin(q4).*5.735764363510462e-1)+dq5.*sin(q5).*(cos(q1).*sin(q4)+cos(q2).*cos(q3).*cos(q4).*sin(q1)+cos(q4).*sin(q1).*sin(q2).*sin(q3))))-real(dq6.*cos(q6).*(cos(q4).*sin(q1).*(-6.710100716628342e-1)+cos(q5).*(cos(q4).*sin(q1).*5.735764363510462e-1+sin(q2-q3).*cos(q1).*8.191520442889917e-1+cos(q2-q3).*cos(q1).*sin(q4).*5.735764363510462e-1).*5.735764363510462e-1+sin(q2-q3).*cos(q1).*4.698463103929542e-1+sin(q5).*(-sin(q1).*sin(q4)+cos(q1).*cos(q2).*cos(q3).*cos(q4)+cos(q1).*cos(q4).*sin(q2).*sin(q3)).*5.735764363510462e-1-cos(q2-q3).*cos(q1).*sin(q4).*6.710100716628342e-1))+imag(dq6.*cos(q6).*(cos(q1).*cos(q4).*6.710100716628342e-1+cos(q5).*(cos(q1).*cos(q4).*(-5.735764363510462e-1)+sin(q2-q3).*sin(q1).*8.191520442889917e-1+cos(q2-q3).*sin(q1).*sin(q4).*5.735764363510462e-1).*5.735764363510462e-1+sin(q2-q3).*sin(q1).*4.698463103929542e-1+sin(q5).*(cos(q1).*sin(q4)+cos(q2).*cos(q3).*cos(q4).*sin(q1)+cos(q4).*sin(q1).*sin(q2).*sin(q3)).*5.735764363510462e-1-cos(q2-q3).*sin(q1).*sin(q4).*6.710100716628342e-1))+real(dq6.*sin(q6).*(sin(q5).*(cos(q4).*sin(q1).*5.735764363510462e-1+sin(q2-q3).*cos(q1).*8.191520442889917e-1+cos(q2-q3).*cos(q1).*sin(q4).*5.735764363510462e-1)-cos(q5).*(-sin(q1).*sin(q4)+cos(q1).*cos(q2).*cos(q3).*cos(q4)+cos(q1).*cos(q4).*sin(q2).*sin(q3))))-imag(dq6.*sin(q6).*(sin(q5).*(cos(q1).*cos(q4).*(-5.735764363510462e-1)+sin(q2-q3).*sin(q1).*8.191520442889917e-1+cos(q2-q3).*sin(q1).*sin(q4).*5.735764363510462e-1)-cos(q5).*(cos(q1).*sin(q4)+cos(q2).*cos(q3).*cos(q4).*sin(q1)+cos(q4).*sin(q1).*sin(q2).*sin(q3))))+imag(sin(q6).*(cos(q5).*(dq1.*cos(q4).*sin(q1).*5.735764363510462e-1+dq4.*cos(q1).*sin(q4).*5.735764363510462e-1+dq1.*sin(q2-q3).*cos(q1).*8.191520442889917e-1+cos(q2-q3).*sin(q1).*(dq2-dq3).*8.191520442889917e-1+dq1.*cos(q2-q3).*cos(q1).*sin(q4).*5.735764363510462e-1+dq4.*cos(q2-q3).*cos(q4).*sin(q1).*5.735764363510462e-1-sin(q2-q3).*sin(q1).*sin(q4).*(dq2-dq3).*5.735764363510462e-1).*5.735764363510462e-1+sin(q5).*(dq4.*cos(q1).*cos(q4)-dq1.*sin(q1).*sin(q4)+dq1.*cos(q1).*cos(q2).*cos(q3).*cos(q4)+dq1.*cos(q1).*cos(q4).*sin(q2).*sin(q3)+dq2.*cos(q2).*cos(q4).*sin(q1).*sin(q3)-dq2.*cos(q3).*cos(q4).*sin(q1).*sin(q2)-dq3.*cos(q2).*cos(q4).*sin(q1).*sin(q3)+dq3.*cos(q3).*cos(q4).*sin(q1).*sin(q2)-dq4.*cos(q2).*cos(q3).*sin(q1).*sin(q4)-dq4.*sin(q1).*sin(q2).*sin(q3).*sin(q4)).*5.735764363510462e-1-dq1.*cos(q4).*sin(q1).*6.710100716628342e-1-dq4.*cos(q1).*sin(q4).*6.710100716628342e-1+dq1.*sin(q2-q3).*cos(q1).*4.698463103929542e-1-dq5.*sin(q5).*(cos(q1).*cos(q4).*(-5.735764363510462e-1)+sin(q2-q3).*sin(q1).*8.191520442889917e-1+cos(q2-q3).*sin(q1).*sin(q4).*5.735764363510462e-1).*5.735764363510462e-1+dq5.*cos(q5).*(cos(q1).*sin(q4)+cos(q2).*cos(q3).*cos(q4).*sin(q1)+cos(q4).*sin(q1).*sin(q2).*sin(q3)).*5.735764363510462e-1+cos(q2-q3).*sin(q1).*(dq2-dq3).*4.698463103929542e-1-dq1.*cos(q2-q3).*cos(q1).*sin(q4).*6.710100716628342e-1-dq4.*cos(q2-q3).*cos(q4).*sin(q1).*6.710100716628342e-1+sin(q2-q3).*sin(q1).*sin(q4).*(dq2-dq3).*6.710100716628342e-1))).*2.0))./((imag(sin(q6).*(cos(q4).*sin(q1).*(-6.710100716628342e-1)+cos(q5).*(cos(q4).*sin(q1).*5.735764363510462e-1+sin(q2-q3).*cos(q1).*8.191520442889917e-1+cos(q2-q3).*cos(q1).*sin(q4).*5.735764363510462e-1).*5.735764363510462e-1+sin(q2-q3).*cos(q1).*4.698463103929542e-1+sin(q5).*(-sin(q1).*sin(q4)+cos(q1).*cos(q2).*cos(q3).*cos(q4)+cos(q1).*cos(q4).*sin(q2).*sin(q3)).*5.735764363510462e-1-cos(q2-q3).*cos(q1).*sin(q4).*6.710100716628342e-1))+imag(cos(q6).*(sin(q5).*(cos(q4).*sin(q1).*5.735764363510462e-1+sin(q2-q3).*cos(q1).*8.191520442889917e-1+cos(q2-q3).*cos(q1).*sin(q4).*5.735764363510462e-1)-cos(q5).*(-sin(q1).*sin(q4)+cos(q1).*cos(q2).*cos(q3).*cos(q4)+cos(q1).*cos(q4).*sin(q2).*sin(q3))))+real(sin(q6).*(cos(q1).*cos(q4).*6.710100716628342e-1+cos(q5).*(cos(q1).*cos(q4).*(-5.735764363510462e-1)+sin(q2-q3).*sin(q1).*8.191520442889917e-1+cos(q2-q3).*sin(q1).*sin(q4).*5.735764363510462e-1).*5.735764363510462e-1+sin(q2-q3).*sin(q1).*4.698463103929542e-1+sin(q5).*(cos(q1).*sin(q4)+cos(q2).*cos(q3).*cos(q4).*sin(q1)+cos(q4).*sin(q1).*sin(q2).*sin(q3)).*5.735764363510462e-1-cos(q2-q3).*sin(q1).*sin(q4).*6.710100716628342e-1))+real(cos(q6).*(sin(q5).*(cos(q1).*cos(q4).*(-5.735764363510462e-1)+sin(q2-q3).*sin(q1).*8.191520442889917e-1+cos(q2-q3).*sin(q1).*sin(q4).*5.735764363510462e-1)-cos(q5).*(cos(q1).*sin(q4)+cos(q2).*cos(q3).*cos(q4).*sin(q1)+cos(q4).*sin(q1).*sin(q2).*sin(q3))))).^2+(real(sin(q6).*(cos(q4).*sin(q1).*(-6.710100716628342e-1)+cos(q5).*(cos(q4).*sin(q1).*5.735764363510462e-1+sin(q2-q3).*cos(q1).*8.191520442889917e-1+cos(q2-q3).*cos(q1).*sin(q4).*5.735764363510462e-1).*5.735764363510462e-1+sin(q2-q3).*cos(q1).*4.698463103929542e-1+sin(q5).*(-sin(q1).*sin(q4)+cos(q1).*cos(q2).*cos(q3).*cos(q4)+cos(q1).*cos(q4).*sin(q2).*sin(q3)).*5.735764363510462e-1-cos(q2-q3).*cos(q1).*sin(q4).*6.710100716628342e-1))+real(cos(q6).*(sin(q5).*(cos(q4).*sin(q1).*5.735764363510462e-1+sin(q2-q3).*cos(q1).*8.191520442889917e-1+cos(q2-q3).*cos(q1).*sin(q4).*5.735764363510462e-1)-cos(q5).*(-sin(q1).*sin(q4)+cos(q1).*cos(q2).*cos(q3).*cos(q4)+cos(q1).*cos(q4).*sin(q2).*sin(q3))))-imag(sin(q6).*(cos(q1).*cos(q4).*6.710100716628342e-1+cos(q5).*(cos(q1).*cos(q4).*(-5.735764363510462e-1)+sin(q2-q3).*sin(q1).*8.191520442889917e-1+cos(q2-q3).*sin(q1).*sin(q4).*5.735764363510462e-1).*5.735764363510462e-1+sin(q2-q3).*sin(q1).*4.698463103929542e-1+sin(q5).*(cos(q1).*sin(q4)+cos(q2).*cos(q3).*cos(q4).*sin(q1)+cos(q4).*sin(q1).*sin(q2).*sin(q3)).*5.735764363510462e-1-cos(q2-q3).*sin(q1).*sin(q4).*6.710100716628342e-1))-imag(cos(q6).*(sin(q5).*(cos(q1).*cos(q4).*(-5.735764363510462e-1)+sin(q2-q3).*sin(q1).*8.191520442889917e-1+cos(q2-q3).*sin(q1).*sin(q4).*5.735764363510462e-1)-cos(q5).*(cos(q1).*sin(q4)+cos(q2).*cos(q3).*cos(q4).*sin(q1)+cos(q4).*sin(q1).*sin(q2).*sin(q3))))).^2)-(((imag(cos(q6).*(cos(q5).*(cos(q1).*cos(q2).*cos(q4).*sin(q3)-cos(q1).*cos(q3).*cos(q4).*sin(q2))-sin(q5).*(cos(q2-q3).*cos(q1).*8.191520442889917e-1-sin(q2-q3).*cos(q1).*sin(q4).*5.735764363510462e-1)))-imag(sin(q6).*(cos(q5).*(cos(q2-q3).*cos(q1).*8.191520442889917e-1-sin(q2-q3).*cos(q1).*sin(q4).*5.735764363510462e-1).*5.735764363510462e-1+sin(q5).*(cos(q1).*cos(q2).*cos(q4).*sin(q3)-cos(q1).*cos(q3).*cos(q4).*sin(q2)).*5.735764363510462e-1+cos(q2-q3).*cos(q1).*4.698463103929542e-1+sin(q2-q3).*cos(q1).*sin(q4).*6.710100716628342e-1))+real(cos(q6).*(cos(q5).*(cos(q2).*cos(q4).*sin(q1).*sin(q3)-cos(q3).*cos(q4).*sin(q1).*sin(q2))-sin(q5).*(cos(q2-q3).*sin(q1).*8.191520442889917e-1-sin(q2-q3).*sin(q1).*sin(q4).*5.735764363510462e-1)))-real(sin(q6).*(cos(q5).*(cos(q2-q3).*sin(q1).*8.191520442889917e-1-sin(q2-q3).*sin(q1).*sin(q4).*5.735764363510462e-1).*5.735764363510462e-1+sin(q5).*(cos(q2).*cos(q4).*sin(q1).*sin(q3)-cos(q3).*cos(q4).*sin(q1).*sin(q2)).*5.735764363510462e-1+cos(q2-q3).*sin(q1).*4.698463103929542e-1+sin(q2-q3).*sin(q1).*sin(q4).*6.710100716628342e-1)))./(real(sin(q6).*(cos(q4).*sin(q1).*(-6.710100716628342e-1)+cos(q5).*(cos(q4).*sin(q1).*5.735764363510462e-1+sin(q2-q3).*cos(q1).*8.191520442889917e-1+cos(q2-q3).*cos(q1).*sin(q4).*5.735764363510462e-1).*5.735764363510462e-1+sin(q2-q3).*cos(q1).*4.698463103929542e-1+sin(q5).*(-sin(q1).*sin(q4)+cos(q1).*cos(q2).*cos(q3).*cos(q4)+cos(q1).*cos(q4).*sin(q2).*sin(q3)).*5.735764363510462e-1-cos(q2-q3).*cos(q1).*sin(q4).*6.710100716628342e-1))+real(cos(q6).*(sin(q5).*(cos(q4).*sin(q1).*5.735764363510462e-1+sin(q2-q3).*cos(q1).*8.191520442889917e-1+cos(q2-q3).*cos(q1).*sin(q4).*5.735764363510462e-1)-cos(q5).*(-sin(q1).*sin(q4)+cos(q1).*cos(q2).*cos(q3).*cos(q4)+cos(q1).*cos(q4).*sin(q2).*sin(q3))))-imag(sin(q6).*(cos(q1).*cos(q4).*6.710100716628342e-1+cos(q5).*(cos(q1).*cos(q4).*(-5.735764363510462e-1)+sin(q2-q3).*sin(q1).*8.191520442889917e-1+cos(q2-q3).*sin(q1).*sin(q4).*5.735764363510462e-1).*5.735764363510462e-1+sin(q2-q3).*sin(q1).*4.698463103929542e-1+sin(q5).*(cos(q1).*sin(q4)+cos(q2).*cos(q3).*cos(q4).*sin(q1)+cos(q4).*sin(q1).*sin(q2).*sin(q3)).*5.735764363510462e-1-cos(q2-q3).*sin(q1).*sin(q4).*6.710100716628342e-1))-imag(cos(q6).*(sin(q5).*(cos(q1).*cos(q4).*(-5.735764363510462e-1)+sin(q2-q3).*sin(q1).*8.191520442889917e-1+cos(q2-q3).*sin(q1).*sin(q4).*5.735764363510462e-1)-cos(q5).*(cos(q1).*sin(q4)+cos(q2).*cos(q3).*cos(q4).*sin(q1)+cos(q4).*sin(q1).*sin(q2).*sin(q3)))))-1.0./(real(sin(q6).*(cos(q4).*sin(q1).*(-6.710100716628342e-1)+cos(q5).*(cos(q4).*sin(q1).*5.735764363510462e-1+sin(q2-q3).*cos(q1).*8.191520442889917e-1+cos(q2-q3).*cos(q1).*sin(q4).*5.735764363510462e-1).*5.735764363510462e-1+sin(q2-q3).*cos(q1).*4.698463103929542e-1+sin(q5).*(-sin(q1).*sin(q4)+cos(q1).*cos(q2).*cos(q3).*cos(q4)+cos(q1).*cos(q4).*sin(q2).*sin(q3)).*5.735764363510462e-1-cos(q2-q3).*cos(q1).*sin(q4).*6.710100716628342e-1))+real(cos(q6).*(sin(q5).*(cos(q4).*sin(q1).*5.735764363510462e-1+sin(q2-q3).*cos(q1).*8.191520442889917e-1+cos(q2-q3).*cos(q1).*sin(q4).*5.735764363510462e-1)-cos(q5).*(-sin(q1).*sin(q4)+cos(q1).*cos(q2).*cos(q3).*cos(q4)+cos(q1).*cos(q4).*sin(q2).*sin(q3))))-imag(sin(q6).*(cos(q1).*cos(q4).*6.710100716628342e-1+cos(q5).*(cos(q1).*cos(q4).*(-5.735764363510462e-1)+sin(q2-q3).*sin(q1).*8.191520442889917e-1+cos(q2-q3).*sin(q1).*sin(q4).*5.735764363510462e-1).*5.735764363510462e-1+sin(q2-q3).*sin(q1).*4.698463103929542e-1+sin(q5).*(cos(q1).*sin(q4)+cos(q2).*cos(q3).*cos(q4).*sin(q1)+cos(q4).*sin(q1).*sin(q2).*sin(q3)).*5.735764363510462e-1-cos(q2-q3).*sin(q1).*sin(q4).*6.710100716628342e-1))-imag(cos(q6).*(sin(q5).*(cos(q1).*cos(q4).*(-5.735764363510462e-1)+sin(q2-q3).*sin(q1).*8.191520442889917e-1+cos(q2-q3).*sin(q1).*sin(q4).*5.735764363510462e-1)-cos(q5).*(cos(q1).*sin(q4)+cos(q2).*cos(q3).*cos(q4).*sin(q1)+cos(q4).*sin(q1).*sin(q2).*sin(q3))))).^2.*(real(cos(q6).*(cos(q5).*(cos(q1).*cos(q2).*cos(q4).*sin(q3)-cos(q1).*cos(q3).*cos(q4).*sin(q2))-sin(q5).*(cos(q2-q3).*cos(q1).*8.191520442889917e-1-sin(q2-q3).*cos(q1).*sin(q4).*5.735764363510462e-1)))-imag(cos(q6).*(cos(q5).*(cos(q2).*cos(q4).*sin(q1).*sin(q3)-cos(q3).*cos(q4).*sin(q1).*sin(q2))-sin(q5).*(cos(q2-q3).*sin(q1).*8.191520442889917e-1-sin(q2-q3).*sin(q1).*sin(q4).*5.735764363510462e-1)))-real(sin(q6).*(cos(q5).*(cos(q2-q3).*cos(q1).*8.191520442889917e-1-sin(q2-q3).*cos(q1).*sin(q4).*5.735764363510462e-1).*5.735764363510462e-1+sin(q5).*(cos(q1).*cos(q2).*cos(q4).*sin(q3)-cos(q1).*cos(q3).*cos(q4).*sin(q2)).*5.735764363510462e-1+cos(q2-q3).*cos(q1).*4.698463103929542e-1+sin(q2-q3).*cos(q1).*sin(q4).*6.710100716628342e-1))+imag(sin(q6).*(cos(q5).*(cos(q2-q3).*sin(q1).*8.191520442889917e-1-sin(q2-q3).*sin(q1).*sin(q4).*5.735764363510462e-1).*5.735764363510462e-1+sin(q5).*(cos(q2).*cos(q4).*sin(q1).*sin(q3)-cos(q3).*cos(q4).*sin(q1).*sin(q2)).*5.735764363510462e-1+cos(q2-q3).*sin(q1).*4.698463103929542e-1+sin(q2-q3).*sin(q1).*sin(q4).*6.710100716628342e-1))).*(imag(sin(q6).*(cos(q4).*sin(q1).*(-6.710100716628342e-1)+cos(q5).*(cos(q4).*sin(q1).*5.735764363510462e-1+sin(q2-q3).*cos(q1).*8.191520442889917e-1+cos(q2-q3).*cos(q1).*sin(q4).*5.735764363510462e-1).*5.735764363510462e-1+sin(q2-q3).*cos(q1).*4.698463103929542e-1+sin(q5).*(-sin(q1).*sin(q4)+cos(q1).*cos(q2).*cos(q3).*cos(q4)+cos(q1).*cos(q4).*sin(q2).*sin(q3)).*5.735764363510462e-1-cos(q2-q3).*cos(q1).*sin(q4).*6.710100716628342e-1))+imag(cos(q6).*(sin(q5).*(cos(q4).*sin(q1).*5.735764363510462e-1+sin(q2-q3).*cos(q1).*8.191520442889917e-1+cos(q2-q3).*cos(q1).*sin(q4).*5.735764363510462e-1)-cos(q5).*(-sin(q1).*sin(q4)+cos(q1).*cos(q2).*cos(q3).*cos(q4)+cos(q1).*cos(q4).*sin(q2).*sin(q3))))+real(sin(q6).*(cos(q1).*cos(q4).*6.710100716628342e-1+cos(q5).*(cos(q1).*cos(q4).*(-5.735764363510462e-1)+sin(q2-q3).*sin(q1).*8.191520442889917e-1+cos(q2-q3).*sin(q1).*sin(q4).*5.735764363510462e-1).*5.735764363510462e-1+sin(q2-q3).*sin(q1).*4.698463103929542e-1+sin(q5).*(cos(q1).*sin(q4)+cos(q2).*cos(q3).*cos(q4).*sin(q1)+cos(q4).*sin(q1).*sin(q2).*sin(q3)).*5.735764363510462e-1-cos(q2-q3).*sin(q1).*sin(q4).*6.710100716628342e-1))+real(cos(q6).*(sin(q5).*(cos(q1).*cos(q4).*(-5.735764363510462e-1)+sin(q2-q3).*sin(q1).*8.191520442889917e-1+cos(q2-q3).*sin(q1).*sin(q4).*5.735764363510462e-1)-cos(q5).*(cos(q1).*sin(q4)+cos(q2).*cos(q3).*cos(q4).*sin(q1)+cos(q4).*sin(q1).*sin(q2).*sin(q3)))))).*(real(sin(q6).*(cos(q4).*sin(q1).*(-6.710100716628342e-1)+cos(q5).*(cos(q4).*sin(q1).*5.735764363510462e-1+sin(q2-q3).*cos(q1).*8.191520442889917e-1+cos(q2-q3).*cos(q1).*sin(q4).*5.735764363510462e-1).*5.735764363510462e-1+sin(q2-q3).*cos(q1).*4.698463103929542e-1+sin(q5).*(-sin(q1).*sin(q4)+cos(q1).*cos(q2).*cos(q3).*cos(q4)+cos(q1).*cos(q4).*sin(q2).*sin(q3)).*5.735764363510462e-1-cos(q2-q3).*cos(q1).*sin(q4).*6.710100716628342e-1))+real(cos(q6).*(sin(q5).*(cos(q4).*sin(q1).*5.735764363510462e-1+sin(q2-q3).*cos(q1).*8.191520442889917e-1+cos(q2-q3).*cos(q1).*sin(q4).*5.735764363510462e-1)-cos(q5).*(-sin(q1).*sin(q4)+cos(q1).*cos(q2).*cos(q3).*cos(q4)+cos(q1).*cos(q4).*sin(q2).*sin(q3))))-imag(sin(q6).*(cos(q1).*cos(q4).*6.710100716628342e-1+cos(q5).*(cos(q1).*cos(q4).*(-5.735764363510462e-1)+sin(q2-q3).*sin(q1).*8.191520442889917e-1+cos(q2-q3).*sin(q1).*sin(q4).*5.735764363510462e-1).*5.735764363510462e-1+sin(q2-q3).*sin(q1).*4.698463103929542e-1+sin(q5).*(cos(q1).*sin(q4)+cos(q2).*cos(q3).*cos(q4).*sin(q1)+cos(q4).*sin(q1).*sin(q2).*sin(q3)).*5.735764363510462e-1-cos(q2-q3).*sin(q1).*sin(q4).*6.710100716628342e-1))-imag(cos(q6).*(sin(q5).*(cos(q1).*cos(q4).*(-5.735764363510462e-1)+sin(q2-q3).*sin(q1).*8.191520442889917e-1+cos(q2-q3).*sin(q1).*sin(q4).*5.735764363510462e-1)-cos(q5).*(cos(q1).*sin(q4)+cos(q2).*cos(q3).*cos(q4).*sin(q1)+cos(q4).*sin(q1).*sin(q2).*sin(q3))))).*(-real(cos(q6).*(-sin(q5).*(dq1.*cos(q1).*cos(q4).*(-5.735764363510462e-1)+dq4.*sin(q1).*sin(q4).*5.735764363510462e-1+dq1.*sin(q2-q3).*sin(q1).*8.191520442889917e-1-cos(q2-q3).*cos(q1).*(dq2-dq3).*8.191520442889917e-1-dq4.*cos(q2-q3).*cos(q1).*cos(q4).*5.735764363510462e-1+dq1.*cos(q2-q3).*sin(q1).*sin(q4).*5.735764363510462e-1+sin(q2-q3).*cos(q1).*sin(q4).*(dq2-dq3).*5.735764363510462e-1)+cos(q5).*(dq1.*cos(q1).*sin(q4)+dq4.*cos(q4).*sin(q1)+dq1.*cos(q2).*cos(q3).*cos(q4).*sin(q1)-dq2.*cos(q1).*cos(q2).*cos(q4).*sin(q3)+dq2.*cos(q1).*cos(q3).*cos(q4).*sin(q2)+dq3.*cos(q1).*cos(q2).*cos(q4).*sin(q3)-dq3.*cos(q1).*cos(q3).*cos(q4).*sin(q2)+dq4.*cos(q1).*cos(q2).*cos(q3).*sin(q4)+dq1.*cos(q4).*sin(q1).*sin(q2).*sin(q3)+dq4.*cos(q1).*sin(q2).*sin(q3).*sin(q4))+dq5.*cos(q5).*(cos(q4).*sin(q1).*5.735764363510462e-1+sin(q2-q3).*cos(q1).*8.191520442889917e-1+cos(q2-q3).*cos(q1).*sin(q4).*5.735764363510462e-1)+dq5.*sin(q5).*(-sin(q1).*sin(q4)+cos(q1).*cos(q2).*cos(q3).*cos(q4)+cos(q1).*cos(q4).*sin(q2).*sin(q3))))+real(sin(q6).*(sin(q5).*(dq1.*cos(q1).*sin(q4)+dq4.*cos(q4).*sin(q1)+dq1.*cos(q2).*cos(q3).*cos(q4).*sin(q1)-dq2.*cos(q1).*cos(q2).*cos(q4).*sin(q3)+dq2.*cos(q1).*cos(q3).*cos(q4).*sin(q2)+dq3.*cos(q1).*cos(q2).*cos(q4).*sin(q3)-dq3.*cos(q1).*cos(q3).*cos(q4).*sin(q2)+dq4.*cos(q1).*cos(q2).*cos(q3).*sin(q4)+dq1.*cos(q4).*sin(q1).*sin(q2).*sin(q3)+dq4.*cos(q1).*sin(q2).*sin(q3).*sin(q4)).*5.735764363510462e-1+cos(q5).*(dq1.*cos(q1).*cos(q4).*(-5.735764363510462e-1)+dq4.*sin(q1).*sin(q4).*5.735764363510462e-1+dq1.*sin(q2-q3).*sin(q1).*8.191520442889917e-1-cos(q2-q3).*cos(q1).*(dq2-dq3).*8.191520442889917e-1-dq4.*cos(q2-q3).*cos(q1).*cos(q4).*5.735764363510462e-1+dq1.*cos(q2-q3).*sin(q1).*sin(q4).*5.735764363510462e-1+sin(q2-q3).*cos(q1).*sin(q4).*(dq2-dq3).*5.735764363510462e-1).*5.735764363510462e-1+dq1.*cos(q1).*cos(q4).*6.710100716628342e-1-dq4.*sin(q1).*sin(q4).*6.710100716628342e-1+dq5.*sin(q5).*(cos(q4).*sin(q1).*5.735764363510462e-1+sin(q2-q3).*cos(q1).*8.191520442889917e-1+cos(q2-q3).*cos(q1).*sin(q4).*5.735764363510462e-1).*5.735764363510462e-1-dq5.*cos(q5).*(-sin(q1).*sin(q4)+cos(q1).*cos(q2).*cos(q3).*cos(q4)+cos(q1).*cos(q4).*sin(q2).*sin(q3)).*5.735764363510462e-1+dq1.*sin(q2-q3).*sin(q1).*4.698463103929542e-1-cos(q2-q3).*cos(q1).*(dq2-dq3).*4.698463103929542e-1+dq4.*cos(q2-q3).*cos(q1).*cos(q4).*6.710100716628342e-1-dq1.*cos(q2-q3).*sin(q1).*sin(q4).*6.710100716628342e-1-sin(q2-q3).*cos(q1).*sin(q4).*(dq2-dq3).*6.710100716628342e-1))+imag(cos(q6).*(sin(q5).*(dq1.*cos(q4).*sin(q1).*5.735764363510462e-1+dq4.*cos(q1).*sin(q4).*5.735764363510462e-1+dq1.*sin(q2-q3).*cos(q1).*8.191520442889917e-1+cos(q2-q3).*sin(q1).*(dq2-dq3).*8.191520442889917e-1+dq1.*cos(q2-q3).*cos(q1).*sin(q4).*5.735764363510462e-1+dq4.*cos(q2-q3).*cos(q4).*sin(q1).*5.735764363510462e-1-sin(q2-q3).*sin(q1).*sin(q4).*(dq2-dq3).*5.735764363510462e-1)-cos(q5).*(dq4.*cos(q1).*cos(q4)-dq1.*sin(q1).*sin(q4)+dq1.*cos(q1).*cos(q2).*cos(q3).*cos(q4)+dq1.*cos(q1).*cos(q4).*sin(q2).*sin(q3)+dq2.*cos(q2).*cos(q4).*sin(q1).*sin(q3)-dq2.*cos(q3).*cos(q4).*sin(q1).*sin(q2)-dq3.*cos(q2).*cos(q4).*sin(q1).*sin(q3)+dq3.*cos(q3).*cos(q4).*sin(q1).*sin(q2)-dq4.*cos(q2).*cos(q3).*sin(q1).*sin(q4)-dq4.*sin(q1).*sin(q2).*sin(q3).*sin(q4))+dq5.*cos(q5).*(cos(q1).*cos(q4).*(-5.735764363510462e-1)+sin(q2-q3).*sin(q1).*8.191520442889917e-1+cos(q2-q3).*sin(q1).*sin(q4).*5.735764363510462e-1)+dq5.*sin(q5).*(cos(q1).*sin(q4)+cos(q2).*cos(q3).*cos(q4).*sin(q1)+cos(q4).*sin(q1).*sin(q2).*sin(q3))))-real(dq6.*cos(q6).*(cos(q4).*sin(q1).*(-6.710100716628342e-1)+cos(q5).*(cos(q4).*sin(q1).*5.735764363510462e-1+sin(q2-q3).*cos(q1).*8.191520442889917e-1+cos(q2-q3).*cos(q1).*sin(q4).*5.735764363510462e-1).*5.735764363510462e-1+sin(q2-q3).*cos(q1).*4.698463103929542e-1+sin(q5).*(-sin(q1).*sin(q4)+cos(q1).*cos(q2).*cos(q3).*cos(q4)+cos(q1).*cos(q4).*sin(q2).*sin(q3)).*5.735764363510462e-1-cos(q2-q3).*cos(q1).*sin(q4).*6.710100716628342e-1))+imag(dq6.*cos(q6).*(cos(q1).*cos(q4).*6.710100716628342e-1+cos(q5).*(cos(q1).*cos(q4).*(-5.735764363510462e-1)+sin(q2-q3).*sin(q1).*8.191520442889917e-1+cos(q2-q3).*sin(q1).*sin(q4).*5.735764363510462e-1).*5.735764363510462e-1+sin(q2-q3).*sin(q1).*4.698463103929542e-1+sin(q5).*(cos(q1).*sin(q4)+cos(q2).*cos(q3).*cos(q4).*sin(q1)+cos(q4).*sin(q1).*sin(q2).*sin(q3)).*5.735764363510462e-1-cos(q2-q3).*sin(q1).*sin(q4).*6.710100716628342e-1))+real(dq6.*sin(q6).*(sin(q5).*(cos(q4).*sin(q1).*5.735764363510462e-1+sin(q2-q3).*cos(q1).*8.191520442889917e-1+cos(q2-q3).*cos(q1).*sin(q4).*5.735764363510462e-1)-cos(q5).*(-sin(q1).*sin(q4)+cos(q1).*cos(q2).*cos(q3).*cos(q4)+cos(q1).*cos(q4).*sin(q2).*sin(q3))))-imag(dq6.*sin(q6).*(sin(q5).*(cos(q1).*cos(q4).*(-5.735764363510462e-1)+sin(q2-q3).*sin(q1).*8.191520442889917e-1+cos(q2-q3).*sin(q1).*sin(q4).*5.735764363510462e-1)-cos(q5).*(cos(q1).*sin(q4)+cos(q2).*cos(q3).*cos(q4).*sin(q1)+cos(q4).*sin(q1).*sin(q2).*sin(q3))))+imag(sin(q6).*(cos(q5).*(dq1.*cos(q4).*sin(q1).*5.735764363510462e-1+dq4.*cos(q1).*sin(q4).*5.735764363510462e-1+dq1.*sin(q2-q3).*cos(q1).*8.191520442889917e-1+cos(q2-q3).*sin(q1).*(dq2-dq3).*8.191520442889917e-1+dq1.*cos(q2-q3).*cos(q1).*sin(q4).*5.735764363510462e-1+dq4.*cos(q2-q3).*cos(q4).*sin(q1).*5.735764363510462e-1-sin(q2-q3).*sin(q1).*sin(q4).*(dq2-dq3).*5.735764363510462e-1).*5.735764363510462e-1+sin(q5).*(dq4.*cos(q1).*cos(q4)-dq1.*sin(q1).*sin(q4)+dq1.*cos(q1).*cos(q2).*cos(q3).*cos(q4)+dq1.*cos(q1).*cos(q4).*sin(q2).*sin(q3)+dq2.*cos(q2).*cos(q4).*sin(q1).*sin(q3)-dq2.*cos(q3).*cos(q4).*sin(q1).*sin(q2)-dq3.*cos(q2).*cos(q4).*sin(q1).*sin(q3)+dq3.*cos(q3).*cos(q4).*sin(q1).*sin(q2)-dq4.*cos(q2).*cos(q3).*sin(q1).*sin(q4)-dq4.*sin(q1).*sin(q2).*sin(q3).*sin(q4)).*5.735764363510462e-1-dq1.*cos(q4).*sin(q1).*6.710100716628342e-1-dq4.*cos(q1).*sin(q4).*6.710100716628342e-1+dq1.*sin(q2-q3).*cos(q1).*4.698463103929542e-1-dq5.*sin(q5).*(cos(q1).*cos(q4).*(-5.735764363510462e-1)+sin(q2-q3).*sin(q1).*8.191520442889917e-1+cos(q2-q3).*sin(q1).*sin(q4).*5.735764363510462e-1).*5.735764363510462e-1+dq5.*cos(q5).*(cos(q1).*sin(q4)+cos(q2).*cos(q3).*cos(q4).*sin(q1)+cos(q4).*sin(q1).*sin(q2).*sin(q3)).*5.735764363510462e-1+cos(q2-q3).*sin(q1).*(dq2-dq3).*4.698463103929542e-1-dq1.*cos(q2-q3).*cos(q1).*sin(q4).*6.710100716628342e-1-dq4.*cos(q2-q3).*cos(q4).*sin(q1).*6.710100716628342e-1+sin(q2-q3).*sin(q1).*sin(q4).*(dq2-dq3).*6.710100716628342e-1))).*2.0)./((imag(sin(q6).*(cos(q4).*sin(q1).*(-6.710100716628342e-1)+cos(q5).*(cos(q4).*sin(q1).*5.735764363510462e-1+sin(q2-q3).*cos(q1).*8.191520442889917e-1+cos(q2-q3).*cos(q1).*sin(q4).*5.735764363510462e-1).*5.735764363510462e-1+sin(q2-q3).*cos(q1).*4.698463103929542e-1+sin(q5).*(-sin(q1).*sin(q4)+cos(q1).*cos(q2).*cos(q3).*cos(q4)+cos(q1).*cos(q4).*sin(q2).*sin(q3)).*5.735764363510462e-1-cos(q2-q3).*cos(q1).*sin(q4).*6.710100716628342e-1))+imag(cos(q6).*(sin(q5).*(cos(q4).*sin(q1).*5.735764363510462e-1+sin(q2-q3).*cos(q1).*8.191520442889917e-1+cos(q2-q3).*cos(q1).*sin(q4).*5.735764363510462e-1)-cos(q5).*(-sin(q1).*sin(q4)+cos(q1).*cos(q2).*cos(q3).*cos(q4)+cos(q1).*cos(q4).*sin(q2).*sin(q3))))+real(sin(q6).*(cos(q1).*cos(q4).*6.710100716628342e-1+cos(q5).*(cos(q1).*cos(q4).*(-5.735764363510462e-1)+sin(q2-q3).*sin(q1).*8.191520442889917e-1+cos(q2-q3).*sin(q1).*sin(q4).*5.735764363510462e-1).*5.735764363510462e-1+sin(q2-q3).*sin(q1).*4.698463103929542e-1+sin(q5).*(cos(q1).*sin(q4)+cos(q2).*cos(q3).*cos(q4).*sin(q1)+cos(q4).*sin(q1).*sin(q2).*sin(q3)).*5.735764363510462e-1-cos(q2-q3).*sin(q1).*sin(q4).*6.710100716628342e-1))+real(cos(q6).*(sin(q5).*(cos(q1).*cos(q4).*(-5.735764363510462e-1)+sin(q2-q3).*sin(q1).*8.191520442889917e-1+cos(q2-q3).*sin(q1).*sin(q4).*5.735764363510462e-1)-cos(q5).*(cos(q1).*sin(q4)+cos(q2).*cos(q3).*cos(q4).*sin(q1)+cos(q4).*sin(q1).*sin(q2).*sin(q3))))).^2+(real(sin(q6).*(cos(q4).*sin(q1).*(-6.710100716628342e-1)+cos(q5).*(cos(q4).*sin(q1).*5.735764363510462e-1+sin(q2-q3).*cos(q1).*8.191520442889917e-1+cos(q2-q3).*cos(q1).*sin(q4).*5.735764363510462e-1).*5.735764363510462e-1+sin(q2-q3).*cos(q1).*4.698463103929542e-1+sin(q5).*(-sin(q1).*sin(q4)+cos(q1).*cos(q2).*cos(q3).*cos(q4)+cos(q1).*cos(q4).*sin(q2).*sin(q3)).*5.735764363510462e-1-cos(q2-q3).*cos(q1).*sin(q4).*6.710100716628342e-1))+real(cos(q6).*(sin(q5).*(cos(q4).*sin(q1).*5.735764363510462e-1+sin(q2-q3).*cos(q1).*8.191520442889917e-1+cos(q2-q3).*cos(q1).*sin(q4).*5.735764363510462e-1)-cos(q5).*(-sin(q1).*sin(q4)+cos(q1).*cos(q2).*cos(q3).*cos(q4)+cos(q1).*cos(q4).*sin(q2).*sin(q3))))-imag(sin(q6).*(cos(q1).*cos(q4).*6.710100716628342e-1+cos(q5).*(cos(q1).*cos(q4).*(-5.735764363510462e-1)+sin(q2-q3).*sin(q1).*8.191520442889917e-1+cos(q2-q3).*sin(q1).*sin(q4).*5.735764363510462e-1).*5.735764363510462e-1+sin(q2-q3).*sin(q1).*4.698463103929542e-1+sin(q5).*(cos(q1).*sin(q4)+cos(q2).*cos(q3).*cos(q4).*sin(q1)+cos(q4).*sin(q1).*sin(q2).*sin(q3)).*5.735764363510462e-1-cos(q2-q3).*sin(q1).*sin(q4).*6.710100716628342e-1))-imag(cos(q6).*(sin(q5).*(cos(q1).*cos(q4).*(-5.735764363510462e-1)+sin(q2-q3).*sin(q1).*8.191520442889917e-1+cos(q2-q3).*sin(q1).*sin(q4).*5.735764363510462e-1)-cos(q5).*(cos(q1).*sin(q4)+cos(q2).*cos(q3).*cos(q4).*sin(q1)+cos(q4).*sin(q1).*sin(q2).*sin(q3))))).^2)+((real(sin(q6).*(cos(q4).*sin(q1).*(-6.710100716628342e-1)+cos(q5).*(cos(q4).*sin(q1).*5.735764363510462e-1+sin(q2-q3).*cos(q1).*8.191520442889917e-1+cos(q2-q3).*cos(q1).*sin(q4).*5.735764363510462e-1).*5.735764363510462e-1+sin(q2-q3).*cos(q1).*4.698463103929542e-1+sin(q5).*(-sin(q1).*sin(q4)+cos(q1).*cos(q2).*cos(q3).*cos(q4)+cos(q1).*cos(q4).*sin(q2).*sin(q3)).*5.735764363510462e-1-cos(q2-q3).*cos(q1).*sin(q4).*6.710100716628342e-1))+real(cos(q6).*(sin(q5).*(cos(q4).*sin(q1).*5.735764363510462e-1+sin(q2-q3).*cos(q1).*8.191520442889917e-1+cos(q2-q3).*cos(q1).*sin(q4).*5.735764363510462e-1)-cos(q5).*(-sin(q1).*sin(q4)+cos(q1).*cos(q2).*cos(q3).*cos(q4)+cos(q1).*cos(q4).*sin(q2).*sin(q3))))-imag(sin(q6).*(cos(q1).*cos(q4).*6.710100716628342e-1+cos(q5).*(cos(q1).*cos(q4).*(-5.735764363510462e-1)+sin(q2-q3).*sin(q1).*8.191520442889917e-1+cos(q2-q3).*sin(q1).*sin(q4).*5.735764363510462e-1).*5.735764363510462e-1+sin(q2-q3).*sin(q1).*4.698463103929542e-1+sin(q5).*(cos(q1).*sin(q4)+cos(q2).*cos(q3).*cos(q4).*sin(q1)+cos(q4).*sin(q1).*sin(q2).*sin(q3)).*5.735764363510462e-1-cos(q2-q3).*sin(q1).*sin(q4).*6.710100716628342e-1))-imag(cos(q6).*(sin(q5).*(cos(q1).*cos(q4).*(-5.735764363510462e-1)+sin(q2-q3).*sin(q1).*8.191520442889917e-1+cos(q2-q3).*sin(q1).*sin(q4).*5.735764363510462e-1)-cos(q5).*(cos(q1).*sin(q4)+cos(q2).*cos(q3).*cos(q4).*sin(q1)+cos(q4).*sin(q1).*sin(q2).*sin(q3))))).*(-real(cos(q6).*(-sin(q5).*(dq1.*cos(q1).*cos(q4).*(-5.735764363510462e-1)+dq4.*sin(q1).*sin(q4).*5.735764363510462e-1+dq1.*sin(q2-q3).*sin(q1).*8.191520442889917e-1-cos(q2-q3).*cos(q1).*(dq2-dq3).*8.191520442889917e-1-dq4.*cos(q2-q3).*cos(q1).*cos(q4).*5.735764363510462e-1+dq1.*cos(q2-q3).*sin(q1).*sin(q4).*5.735764363510462e-1+sin(q2-q3).*cos(q1).*sin(q4).*(dq2-dq3).*5.735764363510462e-1)+cos(q5).*(dq1.*cos(q1).*sin(q4)+dq4.*cos(q4).*sin(q1)+dq1.*cos(q2).*cos(q3).*cos(q4).*sin(q1)-dq2.*cos(q1).*cos(q2).*cos(q4).*sin(q3)+dq2.*cos(q1).*cos(q3).*cos(q4).*sin(q2)+dq3.*cos(q1).*cos(q2).*cos(q4).*sin(q3)-dq3.*cos(q1).*cos(q3).*cos(q4).*sin(q2)+dq4.*cos(q1).*cos(q2).*cos(q3).*sin(q4)+dq1.*cos(q4).*sin(q1).*sin(q2).*sin(q3)+dq4.*cos(q1).*sin(q2).*sin(q3).*sin(q4))+dq5.*cos(q5).*(cos(q4).*sin(q1).*5.735764363510462e-1+sin(q2-q3).*cos(q1).*8.191520442889917e-1+cos(q2-q3).*cos(q1).*sin(q4).*5.735764363510462e-1)+dq5.*sin(q5).*(-sin(q1).*sin(q4)+cos(q1).*cos(q2).*cos(q3).*cos(q4)+cos(q1).*cos(q4).*sin(q2).*sin(q3))))+real(sin(q6).*(sin(q5).*(dq1.*cos(q1).*sin(q4)+dq4.*cos(q4).*sin(q1)+dq1.*cos(q2).*cos(q3).*cos(q4).*sin(q1)-dq2.*cos(q1).*cos(q2).*cos(q4).*sin(q3)+dq2.*cos(q1).*cos(q3).*cos(q4).*sin(q2)+dq3.*cos(q1).*cos(q2).*cos(q4).*sin(q3)-dq3.*cos(q1).*cos(q3).*cos(q4).*sin(q2)+dq4.*cos(q1).*cos(q2).*cos(q3).*sin(q4)+dq1.*cos(q4).*sin(q1).*sin(q2).*sin(q3)+dq4.*cos(q1).*sin(q2).*sin(q3).*sin(q4)).*5.735764363510462e-1+cos(q5).*(dq1.*cos(q1).*cos(q4).*(-5.735764363510462e-1)+dq4.*sin(q1).*sin(q4).*5.735764363510462e-1+dq1.*sin(q2-q3).*sin(q1).*8.191520442889917e-1-cos(q2-q3).*cos(q1).*(dq2-dq3).*8.191520442889917e-1-dq4.*cos(q2-q3).*cos(q1).*cos(q4).*5.735764363510462e-1+dq1.*cos(q2-q3).*sin(q1).*sin(q4).*5.735764363510462e-1+sin(q2-q3).*cos(q1).*sin(q4).*(dq2-dq3).*5.735764363510462e-1).*5.735764363510462e-1+dq1.*cos(q1).*cos(q4).*6.710100716628342e-1-dq4.*sin(q1).*sin(q4).*6.710100716628342e-1+dq5.*sin(q5).*(cos(q4).*sin(q1).*5.735764363510462e-1+sin(q2-q3).*cos(q1).*8.191520442889917e-1+cos(q2-q3).*cos(q1).*sin(q4).*5.735764363510462e-1).*5.735764363510462e-1-dq5.*cos(q5).*(-sin(q1).*sin(q4)+cos(q1).*cos(q2).*cos(q3).*cos(q4)+cos(q1).*cos(q4).*sin(q2).*sin(q3)).*5.735764363510462e-1+dq1.*sin(q2-q3).*sin(q1).*4.698463103929542e-1-cos(q2-q3).*cos(q1).*(dq2-dq3).*4.698463103929542e-1+dq4.*cos(q2-q3).*cos(q1).*cos(q4).*6.710100716628342e-1-dq1.*cos(q2-q3).*sin(q1).*sin(q4).*6.710100716628342e-1-sin(q2-q3).*cos(q1).*sin(q4).*(dq2-dq3).*6.710100716628342e-1))+imag(cos(q6).*(sin(q5).*(dq1.*cos(q4).*sin(q1).*5.735764363510462e-1+dq4.*cos(q1).*sin(q4).*5.735764363510462e-1+dq1.*sin(q2-q3).*cos(q1).*8.191520442889917e-1+cos(q2-q3).*sin(q1).*(dq2-dq3).*8.191520442889917e-1+dq1.*cos(q2-q3).*cos(q1).*sin(q4).*5.735764363510462e-1+dq4.*cos(q2-q3).*cos(q4).*sin(q1).*5.735764363510462e-1-sin(q2-q3).*sin(q1).*sin(q4).*(dq2-dq3).*5.735764363510462e-1)-cos(q5).*(dq4.*cos(q1).*cos(q4)-dq1.*sin(q1).*sin(q4)+dq1.*cos(q1).*cos(q2).*cos(q3).*cos(q4)+dq1.*cos(q1).*cos(q4).*sin(q2).*sin(q3)+dq2.*cos(q2).*cos(q4).*sin(q1).*sin(q3)-dq2.*cos(q3).*cos(q4).*sin(q1).*sin(q2)-dq3.*cos(q2).*cos(q4).*sin(q1).*sin(q3)+dq3.*cos(q3).*cos(q4).*sin(q1).*sin(q2)-dq4.*cos(q2).*cos(q3).*sin(q1).*sin(q4)-dq4.*sin(q1).*sin(q2).*sin(q3).*sin(q4))+dq5.*cos(q5).*(cos(q1).*cos(q4).*(-5.735764363510462e-1)+sin(q2-q3).*sin(q1).*8.191520442889917e-1+cos(q2-q3).*sin(q1).*sin(q4).*5.735764363510462e-1)+dq5.*sin(q5).*(cos(q1).*sin(q4)+cos(q2).*cos(q3).*cos(q4).*sin(q1)+cos(q4).*sin(q1).*sin(q2).*sin(q3))))-real(dq6.*cos(q6).*(cos(q4).*sin(q1).*(-6.710100716628342e-1)+cos(q5).*(cos(q4).*sin(q1).*5.735764363510462e-1+sin(q2-q3).*cos(q1).*8.191520442889917e-1+cos(q2-q3).*cos(q1).*sin(q4).*5.735764363510462e-1).*5.735764363510462e-1+sin(q2-q3).*cos(q1).*4.698463103929542e-1+sin(q5).*(-sin(q1).*sin(q4)+cos(q1).*cos(q2).*cos(q3).*cos(q4)+cos(q1).*cos(q4).*sin(q2).*sin(q3)).*5.735764363510462e-1-cos(q2-q3).*cos(q1).*sin(q4).*6.710100716628342e-1))+imag(dq6.*cos(q6).*(cos(q1).*cos(q4).*6.710100716628342e-1+cos(q5).*(cos(q1).*cos(q4).*(-5.735764363510462e-1)+sin(q2-q3).*sin(q1).*8.191520442889917e-1+cos(q2-q3).*sin(q1).*sin(q4).*5.735764363510462e-1).*5.735764363510462e-1+sin(q2-q3).*sin(q1).*4.698463103929542e-1+sin(q5).*(cos(q1).*sin(q4)+cos(q2).*cos(q3).*cos(q4).*sin(q1)+cos(q4).*sin(q1).*sin(q2).*sin(q3)).*5.735764363510462e-1-cos(q2-q3).*sin(q1).*sin(q4).*6.710100716628342e-1))+real(dq6.*sin(q6).*(sin(q5).*(cos(q4).*sin(q1).*5.735764363510462e-1+sin(q2-q3).*cos(q1).*8.191520442889917e-1+cos(q2-q3).*cos(q1).*sin(q4).*5.735764363510462e-1)-cos(q5).*(-sin(q1).*sin(q4)+cos(q1).*cos(q2).*cos(q3).*cos(q4)+cos(q1).*cos(q4).*sin(q2).*sin(q3))))-imag(dq6.*sin(q6).*(sin(q5).*(cos(q1).*cos(q4).*(-5.735764363510462e-1)+sin(q2-q3).*sin(q1).*8.191520442889917e-1+cos(q2-q3).*sin(q1).*sin(q4).*5.735764363510462e-1)-cos(q5).*(cos(q1).*sin(q4)+cos(q2).*cos(q3).*cos(q4).*sin(q1)+cos(q4).*sin(q1).*sin(q2).*sin(q3))))+imag(sin(q6).*(cos(q5).*(dq1.*cos(q4).*sin(q1).*5.735764363510462e-1+dq4.*cos(q1).*sin(q4).*5.735764363510462e-1+dq1.*sin(q2-q3).*cos(q1).*8.191520442889917e-1+cos(q2-q3).*sin(q1).*(dq2-dq3).*8.191520442889917e-1+dq1.*cos(q2-q3).*cos(q1).*sin(q4).*5.735764363510462e-1+dq4.*cos(q2-q3).*cos(q4).*sin(q1).*5.735764363510462e-1-sin(q2-q3).*sin(q1).*sin(q4).*(dq2-dq3).*5.735764363510462e-1).*5.735764363510462e-1+sin(q5).*(dq4.*cos(q1).*cos(q4)-dq1.*sin(q1).*sin(q4)+dq1.*cos(q1).*cos(q2).*cos(q3).*cos(q4)+dq1.*cos(q1).*cos(q4).*sin(q2).*sin(q3)+dq2.*cos(q2).*cos(q4).*sin(q1).*sin(q3)-dq2.*cos(q3).*cos(q4).*sin(q1).*sin(q2)-dq3.*cos(q2).*cos(q4).*sin(q1).*sin(q3)+dq3.*cos(q3).*cos(q4).*sin(q1).*sin(q2)-dq4.*cos(q2).*cos(q3).*sin(q1).*sin(q4)-dq4.*sin(q1).*sin(q2).*sin(q3).*sin(q4)).*5.735764363510462e-1-dq1.*cos(q4).*sin(q1).*6.710100716628342e-1-dq4.*cos(q1).*sin(q4).*6.710100716628342e-1+dq1.*sin(q2-q3).*cos(q1).*4.698463103929542e-1-dq5.*sin(q5).*(cos(q1).*cos(q4).*(-5.735764363510462e-1)+sin(q2-q3).*sin(q1).*8.191520442889917e-1+cos(q2-q3).*sin(q1).*sin(q4).*5.735764363510462e-1).*5.735764363510462e-1+dq5.*cos(q5).*(cos(q1).*sin(q4)+cos(q2).*cos(q3).*cos(q4).*sin(q1)+cos(q4).*sin(q1).*sin(q2).*sin(q3)).*5.735764363510462e-1+cos(q2-q3).*sin(q1).*(dq2-dq3).*4.698463103929542e-1-dq1.*cos(q2-q3).*cos(q1).*sin(q4).*6.710100716628342e-1-dq4.*cos(q2-q3).*cos(q4).*sin(q1).*6.710100716628342e-1+sin(q2-q3).*sin(q1).*sin(q4).*(dq2-dq3).*6.710100716628342e-1))).*2.0-(imag(sin(q6).*(cos(q4).*sin(q1).*(-6.710100716628342e-1)+cos(q5).*(cos(q4).*sin(q1).*5.735764363510462e-1+sin(q2-q3).*cos(q1).*8.191520442889917e-1+cos(q2-q3).*cos(q1).*sin(q4).*5.735764363510462e-1).*5.735764363510462e-1+sin(q2-q3).*cos(q1).*4.698463103929542e-1+sin(q5).*(-sin(q1).*sin(q4)+cos(q1).*cos(q2).*cos(q3).*cos(q4)+cos(q1).*cos(q4).*sin(q2).*sin(q3)).*5.735764363510462e-1-cos(q2-q3).*cos(q1).*sin(q4).*6.710100716628342e-1))+imag(cos(q6).*(sin(q5).*(cos(q4).*sin(q1).*5.735764363510462e-1+sin(q2-q3).*cos(q1).*8.191520442889917e-1+cos(q2-q3).*cos(q1).*sin(q4).*5.735764363510462e-1)-cos(q5).*(-sin(q1).*sin(q4)+cos(q1).*cos(q2).*cos(q3).*cos(q4)+cos(q1).*cos(q4).*sin(q2).*sin(q3))))+real(sin(q6).*(cos(q1).*cos(q4).*6.710100716628342e-1+cos(q5).*(cos(q1).*cos(q4).*(-5.735764363510462e-1)+sin(q2-q3).*sin(q1).*8.191520442889917e-1+cos(q2-q3).*sin(q1).*sin(q4).*5.735764363510462e-1).*5.735764363510462e-1+sin(q2-q3).*sin(q1).*4.698463103929542e-1+sin(q5).*(cos(q1).*sin(q4)+cos(q2).*cos(q3).*cos(q4).*sin(q1)+cos(q4).*sin(q1).*sin(q2).*sin(q3)).*5.735764363510462e-1-cos(q2-q3).*sin(q1).*sin(q4).*6.710100716628342e-1))+real(cos(q6).*(sin(q5).*(cos(q1).*cos(q4).*(-5.735764363510462e-1)+sin(q2-q3).*sin(q1).*8.191520442889917e-1+cos(q2-q3).*sin(q1).*sin(q4).*5.735764363510462e-1)-cos(q5).*(cos(q1).*sin(q4)+cos(q2).*cos(q3).*cos(q4).*sin(q1)+cos(q4).*sin(q1).*sin(q2).*sin(q3))))).*(real(sin(q6).*(cos(q5).*(dq1.*cos(q4).*sin(q1).*5.735764363510462e-1+dq4.*cos(q1).*sin(q4).*5.735764363510462e-1+dq1.*sin(q2-q3).*cos(q1).*8.191520442889917e-1+cos(q2-q3).*sin(q1).*(dq2-dq3).*8.191520442889917e-1+dq1.*cos(q2-q3).*cos(q1).*sin(q4).*5.735764363510462e-1+dq4.*cos(q2-q3).*cos(q4).*sin(q1).*5.735764363510462e-1-sin(q2-q3).*sin(q1).*sin(q4).*(dq2-dq3).*5.735764363510462e-1).*5.735764363510462e-1+sin(q5).*(dq4.*cos(q1).*cos(q4)-dq1.*sin(q1).*sin(q4)+dq1.*cos(q1).*cos(q2).*cos(q3).*cos(q4)+dq1.*cos(q1).*cos(q4).*sin(q2).*sin(q3)+dq2.*cos(q2).*cos(q4).*sin(q1).*sin(q3)-dq2.*cos(q3).*cos(q4).*sin(q1).*sin(q2)-dq3.*cos(q2).*cos(q4).*sin(q1).*sin(q3)+dq3.*cos(q3).*cos(q4).*sin(q1).*sin(q2)-dq4.*cos(q2).*cos(q3).*sin(q1).*sin(q4)-dq4.*sin(q1).*sin(q2).*sin(q3).*sin(q4)).*5.735764363510462e-1-dq1.*cos(q4).*sin(q1).*6.710100716628342e-1-dq4.*cos(q1).*sin(q4).*6.710100716628342e-1+dq1.*sin(q2-q3).*cos(q1).*4.698463103929542e-1-dq5.*sin(q5).*(cos(q1).*cos(q4).*(-5.735764363510462e-1)+sin(q2-q3).*sin(q1).*8.191520442889917e-1+cos(q2-q3).*sin(q1).*sin(q4).*5.735764363510462e-1).*5.735764363510462e-1+dq5.*cos(q5).*(cos(q1).*sin(q4)+cos(q2).*cos(q3).*cos(q4).*sin(q1)+cos(q4).*sin(q1).*sin(q2).*sin(q3)).*5.735764363510462e-1+cos(q2-q3).*sin(q1).*(dq2-dq3).*4.698463103929542e-1-dq1.*cos(q2-q3).*cos(q1).*sin(q4).*6.710100716628342e-1-dq4.*cos(q2-q3).*cos(q4).*sin(q1).*6.710100716628342e-1+sin(q2-q3).*sin(q1).*sin(q4).*(dq2-dq3).*6.710100716628342e-1))+imag(cos(q6).*(-sin(q5).*(dq1.*cos(q1).*cos(q4).*(-5.735764363510462e-1)+dq4.*sin(q1).*sin(q4).*5.735764363510462e-1+dq1.*sin(q2-q3).*sin(q1).*8.191520442889917e-1-cos(q2-q3).*cos(q1).*(dq2-dq3).*8.191520442889917e-1-dq4.*cos(q2-q3).*cos(q1).*cos(q4).*5.735764363510462e-1+dq1.*cos(q2-q3).*sin(q1).*sin(q4).*5.735764363510462e-1+sin(q2-q3).*cos(q1).*sin(q4).*(dq2-dq3).*5.735764363510462e-1)+cos(q5).*(dq1.*cos(q1).*sin(q4)+dq4.*cos(q4).*sin(q1)+dq1.*cos(q2).*cos(q3).*cos(q4).*sin(q1)-dq2.*cos(q1).*cos(q2).*cos(q4).*sin(q3)+dq2.*cos(q1).*cos(q3).*cos(q4).*sin(q2)+dq3.*cos(q1).*cos(q2).*cos(q4).*sin(q3)-dq3.*cos(q1).*cos(q3).*cos(q4).*sin(q2)+dq4.*cos(q1).*cos(q2).*cos(q3).*sin(q4)+dq1.*cos(q4).*sin(q1).*sin(q2).*sin(q3)+dq4.*cos(q1).*sin(q2).*sin(q3).*sin(q4))+dq5.*cos(q5).*(cos(q4).*sin(q1).*5.735764363510462e-1+sin(q2-q3).*cos(q1).*8.191520442889917e-1+cos(q2-q3).*cos(q1).*sin(q4).*5.735764363510462e-1)+dq5.*sin(q5).*(-sin(q1).*sin(q4)+cos(q1).*cos(q2).*cos(q3).*cos(q4)+cos(q1).*cos(q4).*sin(q2).*sin(q3))))-imag(sin(q6).*(sin(q5).*(dq1.*cos(q1).*sin(q4)+dq4.*cos(q4).*sin(q1)+dq1.*cos(q2).*cos(q3).*cos(q4).*sin(q1)-dq2.*cos(q1).*cos(q2).*cos(q4).*sin(q3)+dq2.*cos(q1).*cos(q3).*cos(q4).*sin(q2)+dq3.*cos(q1).*cos(q2).*cos(q4).*sin(q3)-dq3.*cos(q1).*cos(q3).*cos(q4).*sin(q2)+dq4.*cos(q1).*cos(q2).*cos(q3).*sin(q4)+dq1.*cos(q4).*sin(q1).*sin(q2).*sin(q3)+dq4.*cos(q1).*sin(q2).*sin(q3).*sin(q4)).*5.735764363510462e-1+cos(q5).*(dq1.*cos(q1).*cos(q4).*(-5.735764363510462e-1)+dq4.*sin(q1).*sin(q4).*5.735764363510462e-1+dq1.*sin(q2-q3).*sin(q1).*8.191520442889917e-1-cos(q2-q3).*cos(q1).*(dq2-dq3).*8.191520442889917e-1-dq4.*cos(q2-q3).*cos(q1).*cos(q4).*5.735764363510462e-1+dq1.*cos(q2-q3).*sin(q1).*sin(q4).*5.735764363510462e-1+sin(q2-q3).*cos(q1).*sin(q4).*(dq2-dq3).*5.735764363510462e-1).*5.735764363510462e-1+dq1.*cos(q1).*cos(q4).*6.710100716628342e-1-dq4.*sin(q1).*sin(q4).*6.710100716628342e-1+dq5.*sin(q5).*(cos(q4).*sin(q1).*5.735764363510462e-1+sin(q2-q3).*cos(q1).*8.191520442889917e-1+cos(q2-q3).*cos(q1).*sin(q4).*5.735764363510462e-1).*5.735764363510462e-1-dq5.*cos(q5).*(-sin(q1).*sin(q4)+cos(q1).*cos(q2).*cos(q3).*cos(q4)+cos(q1).*cos(q4).*sin(q2).*sin(q3)).*5.735764363510462e-1+dq1.*sin(q2-q3).*sin(q1).*4.698463103929542e-1-cos(q2-q3).*cos(q1).*(dq2-dq3).*4.698463103929542e-1+dq4.*cos(q2-q3).*cos(q1).*cos(q4).*6.710100716628342e-1-dq1.*cos(q2-q3).*sin(q1).*sin(q4).*6.710100716628342e-1-sin(q2-q3).*cos(q1).*sin(q4).*(dq2-dq3).*6.710100716628342e-1))+imag(dq6.*cos(q6).*(cos(q4).*sin(q1).*(-6.710100716628342e-1)+cos(q5).*(cos(q4).*sin(q1).*5.735764363510462e-1+sin(q2-q3).*cos(q1).*8.191520442889917e-1+cos(q2-q3).*cos(q1).*sin(q4).*5.735764363510462e-1).*5.735764363510462e-1+sin(q2-q3).*cos(q1).*4.698463103929542e-1+sin(q5).*(-sin(q1).*sin(q4)+cos(q1).*cos(q2).*cos(q3).*cos(q4)+cos(q1).*cos(q4).*sin(q2).*sin(q3)).*5.735764363510462e-1-cos(q2-q3).*cos(q1).*sin(q4).*6.710100716628342e-1))+real(cos(q6).*(sin(q5).*(dq1.*cos(q4).*sin(q1).*5.735764363510462e-1+dq4.*cos(q1).*sin(q4).*5.735764363510462e-1+dq1.*sin(q2-q3).*cos(q1).*8.191520442889917e-1+cos(q2-q3).*sin(q1).*(dq2-dq3).*8.191520442889917e-1+dq1.*cos(q2-q3).*cos(q1).*sin(q4).*5.735764363510462e-1+dq4.*cos(q2-q3).*cos(q4).*sin(q1).*5.735764363510462e-1-sin(q2-q3).*sin(q1).*sin(q4).*(dq2-dq3).*5.735764363510462e-1)-cos(q5).*(dq4.*cos(q1).*cos(q4)-dq1.*sin(q1).*sin(q4)+dq1.*cos(q1).*cos(q2).*cos(q3).*cos(q4)+dq1.*cos(q1).*cos(q4).*sin(q2).*sin(q3)+dq2.*cos(q2).*cos(q4).*sin(q1).*sin(q3)-dq2.*cos(q3).*cos(q4).*sin(q1).*sin(q2)-dq3.*cos(q2).*cos(q4).*sin(q1).*sin(q3)+dq3.*cos(q3).*cos(q4).*sin(q1).*sin(q2)-dq4.*cos(q2).*cos(q3).*sin(q1).*sin(q4)-dq4.*sin(q1).*sin(q2).*sin(q3).*sin(q4))+dq5.*cos(q5).*(cos(q1).*cos(q4).*(-5.735764363510462e-1)+sin(q2-q3).*sin(q1).*8.191520442889917e-1+cos(q2-q3).*sin(q1).*sin(q4).*5.735764363510462e-1)+dq5.*sin(q5).*(cos(q1).*sin(q4)+cos(q2).*cos(q3).*cos(q4).*sin(q1)+cos(q4).*sin(q1).*sin(q2).*sin(q3))))+real(dq6.*cos(q6).*(cos(q1).*cos(q4).*6.710100716628342e-1+cos(q5).*(cos(q1).*cos(q4).*(-5.735764363510462e-1)+sin(q2-q3).*sin(q1).*8.191520442889917e-1+cos(q2-q3).*sin(q1).*sin(q4).*5.735764363510462e-1).*5.735764363510462e-1+sin(q2-q3).*sin(q1).*4.698463103929542e-1+sin(q5).*(cos(q1).*sin(q4)+cos(q2).*cos(q3).*cos(q4).*sin(q1)+cos(q4).*sin(q1).*sin(q2).*sin(q3)).*5.735764363510462e-1-cos(q2-q3).*sin(q1).*sin(q4).*6.710100716628342e-1))-imag(dq6.*sin(q6).*(sin(q5).*(cos(q4).*sin(q1).*5.735764363510462e-1+sin(q2-q3).*cos(q1).*8.191520442889917e-1+cos(q2-q3).*cos(q1).*sin(q4).*5.735764363510462e-1)-cos(q5).*(-sin(q1).*sin(q4)+cos(q1).*cos(q2).*cos(q3).*cos(q4)+cos(q1).*cos(q4).*sin(q2).*sin(q3))))-real(dq6.*sin(q6).*(sin(q5).*(cos(q1).*cos(q4).*(-5.735764363510462e-1)+sin(q2-q3).*sin(q1).*8.191520442889917e-1+cos(q2-q3).*sin(q1).*sin(q4).*5.735764363510462e-1)-cos(q5).*(cos(q1).*sin(q4)+cos(q2).*cos(q3).*cos(q4).*sin(q1)+cos(q4).*sin(q1).*sin(q2).*sin(q3))))).*2.0).*((imag(cos(q6).*(cos(q5).*(cos(q1).*cos(q2).*cos(q4).*sin(q3)-cos(q1).*cos(q3).*cos(q4).*sin(q2))-sin(q5).*(cos(q2-q3).*cos(q1).*8.191520442889917e-1-sin(q2-q3).*cos(q1).*sin(q4).*5.735764363510462e-1)))-imag(sin(q6).*(cos(q5).*(cos(q2-q3).*cos(q1).*8.191520442889917e-1-sin(q2-q3).*cos(q1).*sin(q4).*5.735764363510462e-1).*5.735764363510462e-1+sin(q5).*(cos(q1).*cos(q2).*cos(q4).*sin(q3)-cos(q1).*cos(q3).*cos(q4).*sin(q2)).*5.735764363510462e-1+cos(q2-q3).*cos(q1).*4.698463103929542e-1+sin(q2-q3).*cos(q1).*sin(q4).*6.710100716628342e-1))+real(cos(q6).*(cos(q5).*(cos(q2).*cos(q4).*sin(q1).*sin(q3)-cos(q3).*cos(q4).*sin(q1).*sin(q2))-sin(q5).*(cos(q2-q3).*sin(q1).*8.191520442889917e-1-sin(q2-q3).*sin(q1).*sin(q4).*5.735764363510462e-1)))-real(sin(q6).*(cos(q5).*(cos(q2-q3).*sin(q1).*8.191520442889917e-1-sin(q2-q3).*sin(q1).*sin(q4).*5.735764363510462e-1).*5.735764363510462e-1+sin(q5).*(cos(q2).*cos(q4).*sin(q1).*sin(q3)-cos(q3).*cos(q4).*sin(q1).*sin(q2)).*5.735764363510462e-1+cos(q2-q3).*sin(q1).*4.698463103929542e-1+sin(q2-q3).*sin(q1).*sin(q4).*6.710100716628342e-1)))./(real(sin(q6).*(cos(q4).*sin(q1).*(-6.710100716628342e-1)+cos(q5).*(cos(q4).*sin(q1).*5.735764363510462e-1+sin(q2-q3).*cos(q1).*8.191520442889917e-1+cos(q2-q3).*cos(q1).*sin(q4).*5.735764363510462e-1).*5.735764363510462e-1+sin(q2-q3).*cos(q1).*4.698463103929542e-1+sin(q5).*(-sin(q1).*sin(q4)+cos(q1).*cos(q2).*cos(q3).*cos(q4)+cos(q1).*cos(q4).*sin(q2).*sin(q3)).*5.735764363510462e-1-cos(q2-q3).*cos(q1).*sin(q4).*6.710100716628342e-1))+real(cos(q6).*(sin(q5).*(cos(q4).*sin(q1).*5.735764363510462e-1+sin(q2-q3).*cos(q1).*8.191520442889917e-1+cos(q2-q3).*cos(q1).*sin(q4).*5.735764363510462e-1)-cos(q5).*(-sin(q1).*sin(q4)+cos(q1).*cos(q2).*cos(q3).*cos(q4)+cos(q1).*cos(q4).*sin(q2).*sin(q3))))-imag(sin(q6).*(cos(q1).*cos(q4).*6.710100716628342e-1+cos(q5).*(cos(q1).*cos(q4).*(-5.735764363510462e-1)+sin(q2-q3).*sin(q1).*8.191520442889917e-1+cos(q2-q3).*sin(q1).*sin(q4).*5.735764363510462e-1).*5.735764363510462e-1+sin(q2-q3).*sin(q1).*4.698463103929542e-1+sin(q5).*(cos(q1).*sin(q4)+cos(q2).*cos(q3).*cos(q4).*sin(q1)+cos(q4).*sin(q1).*sin(q2).*sin(q3)).*5.735764363510462e-1-cos(q2-q3).*sin(q1).*sin(q4).*6.710100716628342e-1))-imag(cos(q6).*(sin(q5).*(cos(q1).*cos(q4).*(-5.735764363510462e-1)+sin(q2-q3).*sin(q1).*8.191520442889917e-1+cos(q2-q3).*sin(q1).*sin(q4).*5.735764363510462e-1)-cos(q5).*(cos(q1).*sin(q4)+cos(q2).*cos(q3).*cos(q4).*sin(q1)+cos(q4).*sin(q1).*sin(q2).*sin(q3)))))-1.0./(real(sin(q6).*(cos(q4).*sin(q1).*(-6.710100716628342e-1)+cos(q5).*(cos(q4).*sin(q1).*5.735764363510462e-1+sin(q2-q3).*cos(q1).*8.191520442889917e-1+cos(q2-q3).*cos(q1).*sin(q4).*5.735764363510462e-1).*5.735764363510462e-1+sin(q2-q3).*cos(q1).*4.698463103929542e-1+sin(q5).*(-sin(q1).*sin(q4)+cos(q1).*cos(q2).*cos(q3).*cos(q4)+cos(q1).*cos(q4).*sin(q2).*sin(q3)).*5.735764363510462e-1-cos(q2-q3).*cos(q1).*sin(q4).*6.710100716628342e-1))+real(cos(q6).*(sin(q5).*(cos(q4).*sin(q1).*5.735764363510462e-1+sin(q2-q3).*cos(q1).*8.191520442889917e-1+cos(q2-q3).*cos(q1).*sin(q4).*5.735764363510462e-1)-cos(q5).*(-sin(q1).*sin(q4)+cos(q1).*cos(q2).*cos(q3).*cos(q4)+cos(q1).*cos(q4).*sin(q2).*sin(q3))))-imag(sin(q6).*(cos(q1).*cos(q4).*6.710100716628342e-1+cos(q5).*(cos(q1).*cos(q4).*(-5.735764363510462e-1)+sin(q2-q3).*sin(q1).*8.191520442889917e-1+cos(q2-q3).*sin(q1).*sin(q4).*5.735764363510462e-1).*5.735764363510462e-1+sin(q2-q3).*sin(q1).*4.698463103929542e-1+sin(q5).*(cos(q1).*sin(q4)+cos(q2).*cos(q3).*cos(q4).*sin(q1)+cos(q4).*sin(q1).*sin(q2).*sin(q3)).*5.735764363510462e-1-cos(q2-q3).*sin(q1).*sin(q4).*6.710100716628342e-1))-imag(cos(q6).*(sin(q5).*(cos(q1).*cos(q4).*(-5.735764363510462e-1)+sin(q2-q3).*sin(q1).*8.191520442889917e-1+cos(q2-q3).*sin(q1).*sin(q4).*5.735764363510462e-1)-cos(q5).*(cos(q1).*sin(q4)+cos(q2).*cos(q3).*cos(q4).*sin(q1)+cos(q4).*sin(q1).*sin(q2).*sin(q3))))).^2.*(real(cos(q6).*(cos(q5).*(cos(q1).*cos(q2).*cos(q4).*sin(q3)-cos(q1).*cos(q3).*cos(q4).*sin(q2))-sin(q5).*(cos(q2-q3).*cos(q1).*8.191520442889917e-1-sin(q2-q3).*cos(q1).*sin(q4).*5.735764363510462e-1)))-imag(cos(q6).*(cos(q5).*(cos(q2).*cos(q4).*sin(q1).*sin(q3)-cos(q3).*cos(q4).*sin(q1).*sin(q2))-sin(q5).*(cos(q2-q3).*sin(q1).*8.191520442889917e-1-sin(q2-q3).*sin(q1).*sin(q4).*5.735764363510462e-1)))-real(sin(q6).*(cos(q5).*(cos(q2-q3).*cos(q1).*8.191520442889917e-1-sin(q2-q3).*cos(q1).*sin(q4).*5.735764363510462e-1).*5.735764363510462e-1+sin(q5).*(cos(q1).*cos(q2).*cos(q4).*sin(q3)-cos(q1).*cos(q3).*cos(q4).*sin(q2)).*5.735764363510462e-1+cos(q2-q3).*cos(q1).*4.698463103929542e-1+sin(q2-q3).*cos(q1).*sin(q4).*6.710100716628342e-1))+imag(sin(q6).*(cos(q5).*(cos(q2-q3).*sin(q1).*8.191520442889917e-1-sin(q2-q3).*sin(q1).*sin(q4).*5.735764363510462e-1).*5.735764363510462e-1+sin(q5).*(cos(q2).*cos(q4).*sin(q1).*sin(q3)-cos(q3).*cos(q4).*sin(q1).*sin(q2)).*5.735764363510462e-1+cos(q2-q3).*sin(q1).*4.698463103929542e-1+sin(q2-q3).*sin(q1).*sin(q4).*6.710100716628342e-1))).*(imag(sin(q6).*(cos(q4).*sin(q1).*(-6.710100716628342e-1)+cos(q5).*(cos(q4).*sin(q1).*5.735764363510462e-1+sin(q2-q3).*cos(q1).*8.191520442889917e-1+cos(q2-q3).*cos(q1).*sin(q4).*5.735764363510462e-1).*5.735764363510462e-1+sin(q2-q3).*cos(q1).*4.698463103929542e-1+sin(q5).*(-sin(q1).*sin(q4)+cos(q1).*cos(q2).*cos(q3).*cos(q4)+cos(q1).*cos(q4).*sin(q2).*sin(q3)).*5.735764363510462e-1-cos(q2-q3).*cos(q1).*sin(q4).*6.710100716628342e-1))+imag(cos(q6).*(sin(q5).*(cos(q4).*sin(q1).*5.735764363510462e-1+sin(q2-q3).*cos(q1).*8.191520442889917e-1+cos(q2-q3).*cos(q1).*sin(q4).*5.735764363510462e-1)-cos(q5).*(-sin(q1).*sin(q4)+cos(q1).*cos(q2).*cos(q3).*cos(q4)+cos(q1).*cos(q4).*sin(q2).*sin(q3))))+real(sin(q6).*(cos(q1).*cos(q4).*6.710100716628342e-1+cos(q5).*(cos(q1).*cos(q4).*(-5.735764363510462e-1)+sin(q2-q3).*sin(q1).*8.191520442889917e-1+cos(q2-q3).*sin(q1).*sin(q4).*5.735764363510462e-1).*5.735764363510462e-1+sin(q2-q3).*sin(q1).*4.698463103929542e-1+sin(q5).*(cos(q1).*sin(q4)+cos(q2).*cos(q3).*cos(q4).*sin(q1)+cos(q4).*sin(q1).*sin(q2).*sin(q3)).*5.735764363510462e-1-cos(q2-q3).*sin(q1).*sin(q4).*6.710100716628342e-1))+real(cos(q6).*(sin(q5).*(cos(q1).*cos(q4).*(-5.735764363510462e-1)+sin(q2-q3).*sin(q1).*8.191520442889917e-1+cos(q2-q3).*sin(q1).*sin(q4).*5.735764363510462e-1)-cos(q5).*(cos(q1).*sin(q4)+cos(q2).*cos(q3).*cos(q4).*sin(q1)+cos(q4).*sin(q1).*sin(q2).*sin(q3)))))).*1.0./((imag(sin(q6).*(cos(q4).*sin(q1).*(-6.710100716628342e-1)+cos(q5).*(cos(q4).*sin(q1).*5.735764363510462e-1+sin(q2-q3).*cos(q1).*8.191520442889917e-1+cos(q2-q3).*cos(q1).*sin(q4).*5.735764363510462e-1).*5.735764363510462e-1+sin(q2-q3).*cos(q1).*4.698463103929542e-1+sin(q5).*(-sin(q1).*sin(q4)+cos(q1).*cos(q2).*cos(q3).*cos(q4)+cos(q1).*cos(q4).*sin(q2).*sin(q3)).*5.735764363510462e-1-cos(q2-q3).*cos(q1).*sin(q4).*6.710100716628342e-1))+imag(cos(q6).*(sin(q5).*(cos(q4).*sin(q1).*5.735764363510462e-1+sin(q2-q3).*cos(q1).*8.191520442889917e-1+cos(q2-q3).*cos(q1).*sin(q4).*5.735764363510462e-1)-cos(q5).*(-sin(q1).*sin(q4)+cos(q1).*cos(q2).*cos(q3).*cos(q4)+cos(q1).*cos(q4).*sin(q2).*sin(q3))))+real(sin(q6).*(cos(q1).*cos(q4).*6.710100716628342e-1+cos(q5).*(cos(q1).*cos(q4).*(-5.735764363510462e-1)+sin(q2-q3).*sin(q1).*8.191520442889917e-1+cos(q2-q3).*sin(q1).*sin(q4).*5.735764363510462e-1).*5.735764363510462e-1+sin(q2-q3).*sin(q1).*4.698463103929542e-1+sin(q5).*(cos(q1).*sin(q4)+cos(q2).*cos(q3).*cos(q4).*sin(q1)+cos(q4).*sin(q1).*sin(q2).*sin(q3)).*5.735764363510462e-1-cos(q2-q3).*sin(q1).*sin(q4).*6.710100716628342e-1))+real(cos(q6).*(sin(q5).*(cos(q1).*cos(q4).*(-5.735764363510462e-1)+sin(q2-q3).*sin(q1).*8.191520442889917e-1+cos(q2-q3).*sin(q1).*sin(q4).*5.735764363510462e-1)-cos(q5).*(cos(q1).*sin(q4)+cos(q2).*cos(q3).*cos(q4).*sin(q1)+cos(q4).*sin(q1).*sin(q2).*sin(q3))))).^2+(real(sin(q6).*(cos(q4).*sin(q1).*(-6.710100716628342e-1)+cos(q5).*(cos(q4).*sin(q1).*5.735764363510462e-1+sin(q2-q3).*cos(q1).*8.191520442889917e-1+cos(q2-q3).*cos(q1).*sin(q4).*5.735764363510462e-1).*5.735764363510462e-1+sin(q2-q3).*cos(q1).*4.698463103929542e-1+sin(q5).*(-sin(q1).*sin(q4)+cos(q1).*cos(q2).*cos(q3).*cos(q4)+cos(q1).*cos(q4).*sin(q2).*sin(q3)).*5.735764363510462e-1-cos(q2-q3).*cos(q1).*sin(q4).*6.710100716628342e-1))+real(cos(q6).*(sin(q5).*(cos(q4).*sin(q1).*5.735764363510462e-1+sin(q2-q3).*cos(q1).*8.191520442889917e-1+cos(q2-q3).*cos(q1).*sin(q4).*5.735764363510462e-1)-cos(q5).*(-sin(q1).*sin(q4)+cos(q1).*cos(q2).*cos(q3).*cos(q4)+cos(q1).*cos(q4).*sin(q2).*sin(q3))))-imag(sin(q6).*(cos(q1).*cos(q4).*6.710100716628342e-1+cos(q5).*(cos(q1).*cos(q4).*(-5.735764363510462e-1)+sin(q2-q3).*sin(q1).*8.191520442889917e-1+cos(q2-q3).*sin(q1).*sin(q4).*5.735764363510462e-1).*5.735764363510462e-1+sin(q2-q3).*sin(q1).*4.698463103929542e-1+sin(q5).*(cos(q1).*sin(q4)+cos(q2).*cos(q3).*cos(q4).*sin(q1)+cos(q4).*sin(q1).*sin(q2).*sin(q3)).*5.735764363510462e-1-cos(q2-q3).*sin(q1).*sin(q4).*6.710100716628342e-1))-imag(cos(q6).*(sin(q5).*(cos(q1).*cos(q4).*(-5.735764363510462e-1)+sin(q2-q3).*sin(q1).*8.191520442889917e-1+cos(q2-q3).*sin(q1).*sin(q4).*5.735764363510462e-1)-cos(q5).*(cos(q1).*sin(q4)+cos(q2).*cos(q3).*cos(q4).*sin(q1)+cos(q4).*sin(q1).*sin(q2).*sin(q3))))).^2).^2.*(real(sin(q6).*(cos(q4).*sin(q1).*(-6.710100716628342e-1)+cos(q5).*(cos(q4).*sin(q1).*5.735764363510462e-1+sin(q2-q3).*cos(q1).*8.191520442889917e-1+cos(q2-q3).*cos(q1).*sin(q4).*5.735764363510462e-1).*5.735764363510462e-1+sin(q2-q3).*cos(q1).*4.698463103929542e-1+sin(q5).*(-sin(q1).*sin(q4)+cos(q1).*cos(q2).*cos(q3).*cos(q4)+cos(q1).*cos(q4).*sin(q2).*sin(q3)).*5.735764363510462e-1-cos(q2-q3).*cos(q1).*sin(q4).*6.710100716628342e-1))+real(cos(q6).*(sin(q5).*(cos(q4).*sin(q1).*5.735764363510462e-1+sin(q2-q3).*cos(q1).*8.191520442889917e-1+cos(q2-q3).*cos(q1).*sin(q4).*5.735764363510462e-1)-cos(q5).*(-sin(q1).*sin(q4)+cos(q1).*cos(q2).*cos(q3).*cos(q4)+cos(q1).*cos(q4).*sin(q2).*sin(q3))))-imag(sin(q6).*(cos(q1).*cos(q4).*6.710100716628342e-1+cos(q5).*(cos(q1).*cos(q4).*(-5.735764363510462e-1)+sin(q2-q3).*sin(q1).*8.191520442889917e-1+cos(q2-q3).*sin(q1).*sin(q4).*5.735764363510462e-1).*5.735764363510462e-1+sin(q2-q3).*sin(q1).*4.698463103929542e-1+sin(q5).*(cos(q1).*sin(q4)+cos(q2).*cos(q3).*cos(q4).*sin(q1)+cos(q4).*sin(q1).*sin(q2).*sin(q3)).*5.735764363510462e-1-cos(q2-q3).*sin(q1).*sin(q4).*6.710100716628342e-1))-imag(cos(q6).*(sin(q5).*(cos(q1).*cos(q4).*(-5.735764363510462e-1)+sin(q2-q3).*sin(q1).*8.191520442889917e-1+cos(q2-q3).*sin(q1).*sin(q4).*5.735764363510462e-1)-cos(q5).*(cos(q1).*sin(q4)+cos(q2).*cos(q3).*cos(q4).*sin(q1)+cos(q4).*sin(q1).*sin(q2).*sin(q3))))).^2,